simulink model "ScaraRobotApresentacao2023"  (R2024a)
(part 7 of 10)

out1 = ft_5({Ixx4,Ixx5,Ixx6,Ixy4,Ixy5,Ixy6,Ixz4,Ixz5,Ixz6,Iyx4,Iyx5,Iyx6,Iyy4,Iyy5,Iyy6,Iyz4,Iyz5,Iyz6,Izx4,Izx5,Izx6,Izy4,Izy5,Izy6,Izz4,Izz5,Izz6,Lx2,Lx3,Lxcm3,Lxcm4,Lxcm5,Lxcm6,Lycm4,Lycm5,Lycm6,Lz4,Lz5,Lzcm3,Lzcm4,Lzcm5,Lzcm6,dQ1,dQ2,dQ3,dQ4,dQ5,dQ6,et1,et10,et100,et101,et102,et103,et104,et105,et106,et107,et108,et109,et11,et110,et111,et112,et113,et114,et115,et116,et117,et118,et119,et12,et120,et121,et122,et123,et124,et125,et126,et127,et128,et129,et13,et130,et131,et132,et133,et134,et135,et136,et137,et138,et139,et14,et140,et141,et142,et143,et144,et145,et146,et147,et148,et149,et15,et150,et151,et152,et153,et154,et155,et156,et157,et158,et159,et16,et160,et161,et162,et163,et164,et165,et166,et167,et168,et169,et17,et170,et171,et172,et173,et174,et175,et176,et177,et178,et179,et18,et180,et181,et182,et183,et184,et185,et19,et2,et20,et21,et22,et23,et24,et25,et26,et27,et28,et29,et3,et30,et31,et32,et33,et34,et35,et36,et37,et38,et39,et4,et40,et41,et42,et43,et44,et45,et46,et47,et48,et49,et5,et50,et51,et52,et53,et54,et55,et56,et57,et58,et59,et6,et60,et61,et62,et63,et64,et65,et66,et67,et68,et69,et7,et70,et71,et72,et73,et74,et75,et76,et77,et78,et79,et8,et80,et81,et82,et83,et84,et85,et86,et87,et88,et89,et9,et90,et91,et92,et93,et94,et95,et96,et97,et98,et99,m3,m4,m5,m6,t10,t100,t1001,t1002,t1003,t1004,t1005,t1006,t1007,t1008,t1009,t1010,t1011,t1012,t1013,t1014,t1015,t1016,t1017,t1018,t1019,t102,t1020,t1021,t1022,t1023,t1024,t1025,t1026,t1027,t1028,t1029,t1030,t1033,t1034,t1035,t1036,t1037,t1038,t1039,t1041,t1046,t106,t1060,t1061,t1062,t1063,t1064,t1065,t1066,t1067,t107,t1072,t1073,t1074,t1075,t1076,t1077,t1078,t1079,t1082,t1083,t1084,t1085,t1093,t1094,t1095,t1096,t1097,t1098,t1099,t11,t1103,t1104,t1105,t1106,t1107,t1108,t1109,t1110,t1111,t1112,t1113,t1114,t1115,t1116,t1117,t1118,t1120,t1127,t1139,t1140,t1145,t1146,t1147,t1148,t1149,t1150,t1154,t1155,t1158,t1159,t1167,t1169,t1170,t1173,t1174,t1175,t1177,t1178,t1179,t118,t1180,t1181,t1182,t1187,t119,t1193,t1194,t1197,t1198,t1199,t120,t1200,t1202,t1204,t1205,t1206,t1208,t121,t1213,t1214,t1215,t1216,t1217,t1218,t1219,t122,t1223,t1224,t1225,t1226,t1227,t1228,t1229,t123,t1230,t1231,t1236,t1237,t124,t1242,t1243,t1246,t1249,t125,t1250,t1251,t1252,t1253,t1254,t1255,t1256,t1257,t1258,t1259,t126,t1262,t1263,t1264,t1265,t1266,t1269,t127,t1272,t1275,t1276,t1278,t1279,t128,t1283,t1285,t1286,t1287,t1288,t1289,t129,t1290,t1291,t1292,t1293,t1294,t1295,t1296,t1297,t1298,t1299,t130,t1300,t1301,t1302,t1303,t1304,t1305,t1306,t1307,t1308,t1309,t131,t1310,t1311,t1312,t1313,t1314,t1315,t1316,t1317,t1318,t1319,t132,t1320,t1321,t1322,t1323,t1324,t1325,t1326,t1327,t1328,t1329,t1330,t1331,t1332,t1333,t1334,t1335,t1336,t1337,t1338,t1339,t1340,t1341,t1342,t1343,t1344,t1345,t1346,t1347,t1348,t1349,t1350,t1351,t1352,t1353,t1354,t1355,t1356,t1357,t1358,t1359,t136,t1360,t1361,t1362,t1363,t1364,t1365,t1366,t1367,t1368,t1369,t137,t1370,t1371,t1372,t1373,t1374,t1375,t1376,t1377,t1378,t1379,t138,t1381,t1382,t1383,t1384,t1385,t1386,t1387,t1388,t1389,t139,t1390,t1391,t1392,t1393,t1394,t1395,t1396,t1397,t1398,t1399,t1400,t1401,t1402,t1403,t1404,t1405,t1406,t1407,t1408,t1409,t141,t1410,t1411,t142,t1420,t1421,t1422,t1423,t1424,t1425,t1426,t1427,t1428,t1429,t143,t1430,t1431,t1432,t1433,t1434,t1435,t1436,t1437,t1438,t1439,t144,t1440,t1441,t1442,t1443,t1444,t1445,t1446,t1447,t1448,t1449,t145,t1450,t1451,t1452,t1453,t1454,t1455,t1456,t1457,t1458,t146,t1461,t1462,t1469,t147,t1471,t1472,t1474,t1475,t148,t1481,t1482,t1484,t1487,t149,t1490,t1493,t1496,t1497,t1498,t1499,t15,t150,t1500,t1501,t1502,t1503,t1504,t1505,t1506,t1507,t1508,t1509,t151,t1510,t1511,t1512,t1513,t1514,t1515,t1516,t1517,t1518,t1519,t152,t1520,t1521,t1522,t1523,t1524,t1525,t1526,t153,t1531,t1532,t1533,t1534,t1535,t1536,t1539,t154,t1540,t1547,t1548,t1549,t155,t1550,t1555,t156,t1560,t1561,t1562,t1565,t1566,t157,t1575,t1576,t1577,t1578,t1579,t1580,t1581,t1582,t1583,t1589,t1590,t1591,t1592,t1593,t1594,t1595,t1596,t1597,t16,t1600,t1601,t1602,t1603,t1604,t1605,t1610,t1613,t1617,t1618,t1619,t1627,t1628,t1629,t1630,t1631,t1632,t1633,t1634,t1637,t1639,t1640,t1641,t1642,t1643,t1644,t1645,t1646,t1647,t1648,t1649,t1650,t1651,t1652,t1653,t1654,t1655,t1656,t1657,t1658,t1659,t1660,t1661,t1662,t1663,t1664,t1665,t1672,t1673,t1674,t1675,t1676,t1677,t1678,t1679,t1680,t1683,t1684,t1687,t1688,t1691,t1694,t1695,t1696,t1697,t1698,t1699,t17,t170,t1700,t171,t172,t1721,t1722,t1725,t1726,t173,t1730,t1731,t1733,t1734,t1735,t1736,t174,t1740,t1744,t1745,t1754,t1755,t1756,t1759,t1760,t1761,t1762,t1763,t1764,t1765,t1766,t1767,t1768,t1769,t177,t1770,t1771,t1772,t1773,t1774,t1775,t1777,t1778,t1779,t178,t1780,t1781,t1782,t1783,t1784,t1785,t1786,t1787,t1788,t1789,t179,t1790,t1791,t1792,t1793,t1794,t1795,t1796,t1797,t1798,t1799,t18,t180,t1800,t1801,t1802,t1803,t1804,t1808,t1809,t1814,t1815,t1816,t1817,t1818,t1819,t1820,t1821,t1822,t1823,t1827,t1828,t1829,t1830,t1831,t1832,t1833,t1834,t1835,t1840,t1841,t1847,t185,t1850,t1851,t1852,t1853,t1854,t1855,t1856,t1857,t1858,t1859,t186,t1860,t1861,t1862,t1863,t1864,t1865,t1866,t1867,t1868,t1869,t1870,t1871,t1872,t1873,t1874,t1875,t1876,t1877,t1878,t1879,t1880,t1884,t1885,t1886,t1887,t1888,t1889,t1890,t1891,t1892,t1893,t1894,t1895,t1896,t1897,t1898,t1899,t19,t1900,t1901,t1902,t1903,t1904,t1905,t1906,t1907,t1908,t1909,t1910,t1911,t1912,t1913,t1914,t1915,t1916,t1917,t1918,t1919,t1920,t1921,t1922,t1924,t1925,t1926,t1927,t1934,t1935,t1936,t1937,t1938,t1939,t1940,t1944,t1945,t1946,t1947,t1948,t1949,t1950,t1951,t1952,t1959,t1960,t1961,t1962,t1969,t1970,t1971,t1972,t1973,t1974,t1975,t1981,t1982,t1983,t1984,t1985,t1986,t1987,t1988,t1989,t1990,t1991,t1992,t1993,t1994,t1995,t1996,t1997,t1998,t1999,t2,t20,t2000,t2001,t2002,t2003,t201,t202,t2023,t2024,t2025,t2026,t2027,t203,t2034,t2035,t2036,t2037,t2038,t2039,t204,t2040,t2041,t2042,t2043,t2044,t2045,t2047,t2048,t2049,t205,t2050,t2051,t206,t2061,t2062,t2063,t2064,t2065,t2066,t2067,t2068,t207,t2076,t2077,t2078,t208,t2082,t2083,t2084,t209,t2091,t2092,t2093,t2094,t2096,t2097,t2098,t2099,t210,t2100,t2101,t2102,t2103,t2104,t2105,t2106,t2107,t2108,t2109,t211,t2110,t2111,t2112,t2113,t2114,t2115,t2116,t2117,t2118,t2119,t212,t2120,t2121,t2122,t2123,t2125,t2126,t2127,t2128,t2129,t213,t2130,t2131,t2132,t2133,t2134,t2135,t2136,t2137,t2138,t2139,t214,t2140,t2141,t2142,t2143,t2144,t2145,t2147,t2148,t2149,t215,t2150,t2151,t2152,t2153,t2154,t2155,t2156,t2157,t2158,t2159,t216,t2160,t2161,t2162,t2163,t2164,t2165,t2166,t2167,t2168,t2169,t217,t2170,t2171,t2172,t2173,t2174,t2175,t218,t2183,t2184,t2185,t2186,t2187,t2188,t2189,t219,t2190,t2191,t2192,t2193,t2194,t2195,t2196,t2198,t2199,t22,t220,t2200,t2201,t2202,t2203,t2204,t2205,t2206,t2207,t2214,t2215,t2218,t2219,t222,t2220,t2221,t2222,t2223,t2230,t2231,t2232,t2235,t2236,t2237,t2243,t2244,t2245,t2246,t2247,t2248,t225,t2263,t2264,t2265,t2266,t2267,t2268,t2269,t227,t2270,t2271,t2272,t2273,t2274,t2275,t2276,t2277,t2278,t2279,t228,t2280,t2281,t2282,t2283,t2284,t2287,t2288,t2289,t229,t2290,t2291,t2292,t2293,t2294,t2295,t2296,t2297,t2298,t230,t231,t2314,t2315,t2316,t2317,t2318,t2319,t232,t2320,t2321,t2322,t2323,t2324,t2325,t2326,t2327,t233,t2331,t2332,t2333,t2334,t2336,t2337,t2338,t2339,t234,t2340,t2341,t2342,t2343,t2344,t2345,t2346,t2347,t2348,t235,t2353,t2354,t2355,t236,t2360,t2362,t2363,t2364,t2365,t2366,t2367,t2368,t2369,t237,t2370,t2371,t2372,t2373,t2374,t2375,t2376,t2377,t2378,t2383,t2384,t2385,t2386,t2387,t2388,t2389,t239,t2390,t2391,t2392,t2393,t2394,t2395,t2396,t2397,t2398,t2399,t240,t2404,t2405,t2406,t2407,t2408,t2409,t2412,t2413,t2414,t2415,t2416,t2417,t242,t243,t244,t245,t25,t250,t251,t252,t253,t258,t259,t26,t260,t263,t264,t265,t266,t269,t270,t273,t274,t276,t277,t278,t279,t282,t283,t286,t287,t289,t290,t292,t293,t297,t298,t299,t3,t300,t301,t302,t303,t304,t305,t306,t307,t308,t309,t310,t311,t312,t313,t314,t315,t316,t317,t318,t319,t32,t320,t321,t322,t323,t324,t325,t326,t327,t328,t33,t331,t332,t333,t334,t34,t340,t341,t342,t343,t349,t35,t351,t358,t36,t363,t364,t367,t368,t369,t370,t377,t378,t379,t380,t381,t382,t383,t384,t385,t386,t39,t4,t40,t402,t403,t404,t405,t406,t407,t41,t413,t414,t415,t416,t417,t418,t419,t42,t43,t430,t431,t432,t433,t434,t435,t436,t437,t438,t44,t442,t443,t444,t445,t446,t447,t45,t454,t455,t456,t457,t458,t459,t46,t460,t461,t462,t463,t464,t465,t466,t467,t468,t469,t47,t470,t471,t472,t473,t474,t475,t476,t477,t478,t479,t48,t480,t481,t482,t483,t484,t485,t486,t487,t488,t489,t49,t490,t491,t492,t493,t494,t495,t496,t497,t498,t5,t50,t500,t506,t51,t512,t514,t515,t516,t52,t527,t528,t529,t53,t54,t540,t542,t543,t544,t546,t547,t548,t55,t550,t552,t554,t555,t556,t557,t558,t559,t56,t560,t561,t562,t563,t564,t565,t566,t567,t568,t569,t57,t570,t571,t572,t573,t574,t575,t576,t577,t578,t579,t58,t580,t581,t582,t583,t584,t585,t586,t587,t588,t589,t59,t590,t591,t592,t593,t594,t595,t596,t597,t598,t599,t6,t60,t600,t601,t602,t603,t604,t605,t606,t607,t608,t609,t61,t610,t611,t612,t613,t614,t615,t616,t617,t618,t619,t62,t620,t621,t622,t623,t624,t625,t626,t627,t628,t629,t63,t630,t631,t632,t635,t636,t637,t638,t64,t648,t650,t651,t658,t659,t660,t661,t662,t663,t664,t669,t67,t670,t671,t674,t675,t676,t677,t68,t681,t684,t687,t688,t689,t69,t690,t694,t697,t698,t699,t7,t70,t700,t701,t702,t703,t704,t705,t706,t707,t708,t709,t71,t710,t711,t716,t717,t718,t719,t72,t720,t721,t724,t725,t728,t729,t73,t730,t731,t732,t733,t734,t735,t737,t738,t739,t74,t746,t748,t749,t75,t750,t752,t754,t755,t756,t759,t760,t761,t762,t774,t775,t776,t777,t778,t779,t78,t780,t781,t782,t783,t785,t788,t79,t791,t792,t793,t794,t795,t796,t797,t798,t8,t80,t800,t801,t803,t804,t806,t807,t809,t81,t810,t82,t828,t829,t83,t830,t831,t832,t833,t834,t835,t836,t837,t838,t839,t84,t840,t843,t844,t845,t848,t849,t85,t851,t852,t857,t858,t86,t861,t862,t868,t869,t87,t870,t871,t872,t873,t874,t875,t876,t877,t878,t879,t88,t880,t881,t882,t883,t884,t885,t886,t887,t888,t889,t89,t890,t891,t892,t893,t894,t895,t896,t897,t898,t899,t9,t90,t900,t901,t902,t903,t904,t905,t906,t907,t908,t909,t91,t910,t911,t912,t913,t914,t915,t916,t917,t918,t919,t92,t920,t921,t922,t923,t924,t925,t926,t927,t928,t929,t93,t930,t931,t932,t933,t934,t935,t936,t938,t939,t94,t940,t941,t942,t943,t948,t949,t950,t951,t952,t953,t954,t955,t956,t957,t958,t959,t96,t960,t961,t962,t963,t964,t965,t966,t967,t968,t969,t972,t973,t978,t979,t984,t985,t988,t989,t990,t991,t992,t993,t994,t995,t996,t997,t998});
end
function out1 = ft_5(ct)
[Ixx4,Ixx5,Ixx6,Ixy4,Ixy5,Ixy6,Ixz4,Ixz5,Ixz6,Iyx4,Iyx5,Iyx6,Iyy4,Iyy5,Iyy6,Iyz4,Iyz5,Iyz6,Izx4,Izx5,Izx6,Izy4,Izy5,Izy6,Izz4,Izz5,Izz6,Lx2,Lx3,Lxcm3,Lxcm4,Lxcm5,Lxcm6,Lycm4,Lycm5,Lycm6,Lz4,Lz5,Lzcm3,Lzcm4,Lzcm5,Lzcm6,dQ1,dQ2,dQ3,dQ4,dQ5,dQ6,et1,et10,et100,et101,et102,et103,et104,et105,et106,et107,et108,et109,et11,et110,et111,et112,et113,et114,et115,et116,et117,et118,et119,et12,et120,et121,et122,et123,et124,et125,et126,et127,et128,et129,et13,et130,et131,et132,et133,et134,et135,et136,et137,et138,et139,et14,et140,et141,et142,et143,et144,et145,et146,et147,et148,et149,et15,et150,et151,et152,et153,et154,et155,et156,et157,et158,et159,et16,et160,et161,et162,et163,et164,et165,et166,et167,et168,et169,et17,et170,et171,et172,et173,et174,et175,et176,et177,et178,et179,et18,et180,et181,et182,et183,et184,et185,et19,et2,et20,et21,et22,et23,et24,et25,et26,et27,et28,et29,et3,et30,et31,et32,et33,et34,et35,et36,et37,et38,et39,et4,et40,et41,et42,et43,et44,et45,et46,et47,et48,et49,et5,et50,et51,et52,et53,et54,et55,et56,et57,et58,et59,et6,et60,et61,et62,et63,et64,et65,et66,et67,et68,et69,et7,et70,et71,et72,et73,et74,et75,et76,et77,et78,et79,et8,et80,et81,et82,et83,et84,et85,et86,et87,et88,et89,et9,et90,et91,et92,et93,et94,et95,et96,et97,et98,et99,m3,m4,m5,m6,t10,t100,t1001,t1002,t1003,t1004,t1005,t1006,t1007,t1008,t1009,t1010,t1011,t1012,t1013,t1014,t1015,t1016,t1017,t1018,t1019,t102,t1020,t1021,t1022,t1023,t1024,t1025,t1026,t1027,t1028,t1029,t1030,t1033,t1034,t1035,t1036,t1037,t1038,t1039,t1041,t1046,t106,t1060,t1061,t1062,t1063,t1064,t1065,t1066,t1067,t107,t1072,t1073,t1074,t1075,t1076,t1077,t1078,t1079,t1082,t1083,t1084,t1085,t1093,t1094,t1095,t1096,t1097,t1098,t1099,t11,t1103,t1104,t1105,t1106,t1107,t1108,t1109,t1110,t1111,t1112,t1113,t1114,t1115,t1116,t1117,t1118,t1120,t1127,t1139,t1140,t1145,t1146,t1147,t1148,t1149,t1150,t1154,t1155,t1158,t1159,t1167,t1169,t1170,t1173,t1174,t1175,t1177,t1178,t1179,t118,t1180,t1181,t1182,t1187,t119,t1193,t1194,t1197,t1198,t1199,t120,t1200,t1202,t1204,t1205,t1206,t1208,t121,t1213,t1214,t1215,t1216,t1217,t1218,t1219,t122,t1223,t1224,t1225,t1226,t1227,t1228,t1229,t123,t1230,t1231,t1236,t1237,t124,t1242,t1243,t1246,t1249,t125,t1250,t1251,t1252,t1253,t1254,t1255,t1256,t1257,t1258,t1259,t126,t1262,t1263,t1264,t1265,t1266,t1269,t127,t1272,t1275,t1276,t1278,t1279,t128,t1283,t1285,t1286,t1287,t1288,t1289,t129,t1290,t1291,t1292,t1293,t1294,t1295,t1296,t1297,t1298,t1299,t130,t1300,t1301,t1302,t1303,t1304,t1305,t1306,t1307,t1308,t1309,t131,t1310,t1311,t1312,t1313,t1314,t1315,t1316,t1317,t1318,t1319,t132,t1320,t1321,t1322,t1323,t1324,t1325,t1326,t1327,t1328,t1329,t1330,t1331,t1332,t1333,t1334,t1335,t1336,t1337,t1338,t1339,t1340,t1341,t1342,t1343,t1344,t1345,t1346,t1347,t1348,t1349,t1350,t1351,t1352,t1353,t1354,t1355,t1356,t1357,t1358,t1359,t136,t1360,t1361,t1362,t1363,t1364,t1365,t1366,t1367,t1368,t1369,t137,t1370,t1371,t1372,t1373,t1374,t1375,t1376,t1377,t1378,t1379,t138,t1381,t1382,t1383,t1384,t1385,t1386,t1387,t1388,t1389,t139,t1390,t1391,t1392,t1393,t1394,t1395,t1396,t1397,t1398,t1399,t1400,t1401,t1402,t1403,t1404,t1405,t1406,t1407,t1408,t1409,t141,t1410,t1411,t142,t1420,t1421,t1422,t1423,t1424,t1425,t1426,t1427,t1428,t1429,t143,t1430,t1431,t1432,t1433,t1434,t1435,t1436,t1437,t1438,t1439,t144,t1440,t1441,t1442,t1443,t1444,t1445,t1446,t1447,t1448,t1449,t145,t1450,t1451,t1452,t1453,t1454,t1455,t1456,t1457,t1458,t146,t1461,t1462,t1469,t147,t1471,t1472,t1474,t1475,t148,t1481,t1482,t1484,t1487,t149,t1490,t1493,t1496,t1497,t1498,t1499,t15,t150,t1500,t1501,t1502,t1503,t1504,t1505,t1506,t1507,t1508,t1509,t151,t1510,t1511,t1512,t1513,t1514,t1515,t1516,t1517,t1518,t1519,t152,t1520,t1521,t1522,t1523,t1524,t1525,t1526,t153,t1531,t1532,t1533,t1534,t1535,t1536,t1539,t154,t1540,t1547,t1548,t1549,t155,t1550,t1555,t156,t1560,t1561,t1562,t1565,t1566,t157,t1575,t1576,t1577,t1578,t1579,t1580,t1581,t1582,t1583,t1589,t1590,t1591,t1592,t1593,t1594,t1595,t1596,t1597,t16,t1600,t1601,t1602,t1603,t1604,t1605,t1610,t1613,t1617,t1618,t1619,t1627,t1628,t1629,t1630,t1631,t1632,t1633,t1634,t1637,t1639,t1640,t1641,t1642,t1643,t1644,t1645,t1646,t1647,t1648,t1649,t1650,t1651,t1652,t1653,t1654,t1655,t1656,t1657,t1658,t1659,t1660,t1661,t1662,t1663,t1664,t1665,t1672,t1673,t1674,t1675,t1676,t1677,t1678,t1679,t1680,t1683,t1684,t1687,t1688,t1691,t1694,t1695,t1696,t1697,t1698,t1699,t17,t170,t1700,t171,t172,t1721,t1722,t1725,t1726,t173,t1730,t1731,t1733,t1734,t1735,t1736,t174,t1740,t1744,t1745,t1754,t1755,t1756,t1759,t1760,t1761,t1762,t1763,t1764,t1765,t1766,t1767,t1768,t1769,t177,t1770,t1771,t1772,t1773,t1774,t1775,t1777,t1778,t1779,t178,t1780,t1781,t1782,t1783,t1784,t1785,t1786,t1787,t1788,t1789,t179,t1790,t1791,t1792,t1793,t1794,t1795,t1796,t1797,t1798,t1799,t18,t180,t1800,t1801,t1802,t1803,t1804,t1808,t1809,t1814,t1815,t1816,t1817,t1818,t1819,t1820,t1821,t1822,t1823,t1827,t1828,t1829,t1830,t1831,t1832,t1833,t1834,t1835,t1840,t1841,t1847,t185,t1850,t1851,t1852,t1853,t1854,t1855,t1856,t1857,t1858,t1859,t186,t1860,t1861,t1862,t1863,t1864,t1865,t1866,t1867,t1868,t1869,t1870,t1871,t1872,t1873,t1874,t1875,t1876,t1877,t1878,t1879,t1880,t1884,t1885,t1886,t1887,t1888,t1889,t1890,t1891,t1892,t1893,t1894,t1895,t1896,t1897,t1898,t1899,t19,t1900,t1901,t1902,t1903,t1904,t1905,t1906,t1907,t1908,t1909,t1910,t1911,t1912,t1913,t1914,t1915,t1916,t1917,t1918,t1919,t1920,t1921,t1922,t1924,t1925,t1926,t1927,t1934,t1935,t1936,t1937,t1938,t1939,t1940,t1944,t1945,t1946,t1947,t1948,t1949,t1950,t1951,t1952,t1959,t1960,t1961,t1962,t1969,t1970,t1971,t1972,t1973,t1974,t1975,t1981,t1982,t1983,t1984,t1985,t1986,t1987,t1988,t1989,t1990,t1991,t1992,t1993,t1994,t1995,t1996,t1997,t1998,t1999,t2,t20,t2000,t2001,t2002,t2003,t201,t202,t2023,t2024,t2025,t2026,t2027,t203,t2034,t2035,t2036,t2037,t2038,t2039,t204,t2040,t2041,t2042,t2043,t2044,t2045,t2047,t2048,t2049,t205,t2050,t2051,t206,t2061,t2062,t2063,t2064,t2065,t2066,t2067,t2068,t207,t2076,t2077,t2078,t208,t2082,t2083,t2084,t209,t2091,t2092,t2093,t2094,t2096,t2097,t2098,t2099,t210,t2100,t2101,t2102,t2103,t2104,t2105,t2106,t2107,t2108,t2109,t211,t2110,t2111,t2112,t2113,t2114,t2115,t2116,t2117,t2118,t2119,t212,t2120,t2121,t2122,t2123,t2125,t2126,t2127,t2128,t2129,t213,t2130,t2131,t2132,t2133,t2134,t2135,t2136,t2137,t2138,t2139,t214,t2140,t2141,t2142,t2143,t2144,t2145,t2147,t2148,t2149,t215,t2150,t2151,t2152,t2153,t2154,t2155,t2156,t2157,t2158,t2159,t216,t2160,t2161,t2162,t2163,t2164,t2165,t2166,t2167,t2168,t2169,t217,t2170,t2171,t2172,t2173,t2174,t2175,t218,t2183,t2184,t2185,t2186,t2187,t2188,t2189,t219,t2190,t2191,t2192,t2193,t2194,t2195,t2196,t2198,t2199,t22,t220,t2200,t2201,t2202,t2203,t2204,t2205,t2206,t2207,t2214,t2215,t2218,t2219,t222,t2220,t2221,t2222,t2223,t2230,t2231,t2232,t2235,t2236,t2237,t2243,t2244,t2245,t2246,t2247,t2248,t225,t2263,t2264,t2265,t2266,t2267,t2268,t2269,t227,t2270,t2271,t2272,t2273,t2274,t2275,t2276,t2277,t2278,t2279,t228,t2280,t2281,t2282,t2283,t2284,t2287,t2288,t2289,t229,t2290,t2291,t2292,t2293,t2294,t2295,t2296,t2297,t2298,t230,t231,t2314,t2315,t2316,t2317,t2318,t2319,t232,t2320,t2321,t2322,t2323,t2324,t2325,t2326,t2327,t233,t2331,t2332,t2333,t2334,t2336,t2337,t2338,t2339,t234,t2340,t2341,t2342,t2343,t2344,t2345,t2346,t2347,t2348,t235,t2353,t2354,t2355,t236,t2360,t2362,t2363,t2364,t2365,t2366,t2367,t2368,t2369,t237,t2370,t2371,t2372,t2373,t2374,t2375,t2376,t2377,t2378,t2383,t2384,t2385,t2386,t2387,t2388,t2389,t239,t2390,t2391,t2392,t2393,t2394,t2395,t2396,t2397,t2398,t2399,t240,t2404,t2405,t2406,t2407,t2408,t2409,t2412,t2413,t2414,t2415,t2416,t2417,t242,t243,t244,t245,t25,t250,t251,t252,t253,t258,t259,t26,t260,t263,t264,t265,t266,t269,t270,t273,t274,t276,t277,t278,t279,t282,t283,t286,t287,t289,t290,t292,t293,t297,t298,t299,t3,t300,t301,t302,t303,t304,t305,t306,t307,t308,t309,t310,t311,t312,t313,t314,t315,t316,t317,t318,t319,t32,t320,t321,t322,t323,t324,t325,t326,t327,t328,t33,t331,t332,t333,t334,t34,t340,t341,t342,t343,t349,t35,t351,t358,t36,t363,t364,t367,t368,t369,t370,t377,t378,t379,t380,t381,t382,t383,t384,t385,t386,t39,t4,t40,t402,t403,t404,t405,t406,t407,t41,t413,t414,t415,t416,t417,t418,t419,t42,t43,t430,t431,t432,t433,t434,t435,t436,t437,t438,t44,t442,t443,t444,t445,t446,t447,t45,t454,t455,t456,t457,t458,t459,t46,t460,t461,t462,t463,t464,t465,t466,t467,t468,t469,t47,t470,t471,t472,t473,t474,t475,t476,t477,t478,t479,t48,t480,t481,t482,t483,t484,t485,t486,t487,t488,t489,t49,t490,t491,t492,t493,t494,t495,t496,t497,t498,t5,t50,t500,t506,t51,t512,t514,t515,t516,t52,t527,t528,t529,t53,t54,t540,t542,t543,t544,t546,t547,t548,t55,t550,t552,t554,t555,t556,t557,t558,t559,t56,t560,t561,t562,t563,t564,t565,t566,t567,t568,t569,t57,t570,t571,t572,t573,t574,t575,t576,t577,t578,t579,t58,t580,t581,t582,t583,t584,t585,t586,t587,t588,t589,t59,t590,t591,t592,t593,t594,t595,t596,t597,t598,t599,t6,t60,t600,t601,t602,t603,t604,t605,t606,t607,t608,t609,t61,t610,t611,t612,t613,t614,t615,t616,t617,t618,t619,t62,t620,t621,t622,t623,t624,t625,t626,t627,t628,t629,t63,t630,t631,t632,t635,t636,t637,t638,t64,t648,t650,t651,t658,t659,t660,t661,t662,t663,t664,t669,t67,t670,t671,t674,t675,t676,t677,t68,t681,t684,t687,t688,t689,t69,t690,t694,t697,t698,t699,t7,t70,t700,t701,t702,t703,t704,t705,t706,t707,t708,t709,t71,t710,t711,t716,t717,t718,t719,t72,t720,t721,t724,t725,t728,t729,t73,t730,t731,t732,t733,t734,t735,t737,t738,t739,t74,t746,t748,t749,t75,t750,t752,t754,t755,t756,t759,t760,t761,t762,t774,t775,t776,t777,t778,t779,t78,t780,t781,t782,t783,t785,t788,t79,t791,t792,t793,t794,t795,t796,t797,t798,t8,t80,t800,t801,t803,t804,t806,t807,t809,t81,t810,t82,t828,t829,t83,t830,t831,t832,t833,t834,t835,t836,t837,t838,t839,t84,t840,t843,t844,t845,t848,t849,t85,t851,t852,t857,t858,t86,t861,t862,t868,t869,t87,t870,t871,t872,t873,t874,t875,t876,t877,t878,t879,t88,t880,t881,t882,t883,t884,t885,t886,t887,t888,t889,t89,t890,t891,t892,t893,t894,t895,t896,t897,t898,t899,t9,t90,t900,t901,t902,t903,t904,t905,t906,t907,t908,t909,t91,t910,t911,t912,t913,t914,t915,t916,t917,t918,t919,t92,t920,t921,t922,t923,t924,t925,t926,t927,t928,t929,t93,t930,t931,t932,t933,t934,t935,t936,t938,t939,t94,t940,t941,t942,t943,t948,t949,t950,t951,t952,t953,t954,t955,t956,t957,t958,t959,t96,t960,t961,t962,t963,t964,t965,t966,t967,t968,t969,t972,t973,t978,t979,t984,t985,t988,t989,t990,t991,t992,t993,t994,t995,t996,t997,t998] = ct{:};
et186 = Ixz6.*dQ1.*dQ4.*t4.*t5.*t6.*t9.*t10.*t33.*2.0+Ixz6.*dQ3.*dQ4.*t2.*t5.*t6.*t8.*t10.*t34.*2.0+Ixz6.*dQ3.*dQ4.*t3.*t5.*t6.*t7.*t10.*t34.*2.0+Ixz6.*dQ1.*dQ5.*t2.*t7.*t9.*t10.*t11.*t33.*2.0+Ixz6.*dQ1.*dQ5.*t3.*t8.*t9.*t10.*t11.*t32.*2.0-Ixz5.*dQ1.*dQ2.*t2.*t5.*t7.*t10.*t33.*t34.*4.0-Ixz5.*dQ1.*dQ2.*t3.*t5.*t8.*t10.*t32.*t34.*4.0-Ixz5.*dQ1.*dQ3.*t2.*t5.*t7.*t10.*t33.*t34.*4.0-Ixz5.*dQ1.*dQ5.*t2.*t3.*t7.*t8.*t34.*t35.*4.0-Ixz5.*dQ1.*dQ3.*t3.*t5.*t8.*t10.*t32.*t34.*4.0-Ixz5.*dQ1.*dQ4.*t4.*t5.*t9.*t10.*t32.*t33.*4.0-Ixz6.*dQ1.*dQ4.*t2.*t6.*t7.*t9.*t33.*t35.*4.0-Ixz6.*dQ1.*dQ4.*t3.*t6.*t8.*t9.*t32.*t35.*4.0-Ixz6.*dQ1.*dQ6.*t2.*t4.*t7.*t11.*t33.*t35.*4.0-Ixz6.*dQ1.*dQ5.*t4.*t5.*t9.*t11.*t32.*t33.*2.0-Ixz6.*dQ1.*dQ6.*t3.*t4.*t8.*t11.*t32.*t35.*4.0-Ixz6.*dQ1.*dQ6.*t4.*t6.*t9.*t10.*t32.*t33.*2.0;
et187 = Ixz6.*dQ1.*dQ6.*t5.*t10.*t11.*t32.*t33.*t34.*-2.0-Iyx6.*dQ2.*dQ3.*t2.*t3.*t4.*t6.*t9.*t11.*2.0-Iyx5.*dQ1.*dQ2.*t2.*t3.*t7.*t8.*t9.*t10.*4.0-Iyx5.*dQ1.*dQ3.*t2.*t3.*t7.*t8.*t9.*t10.*4.0+Iyx6.*dQ1.*dQ2.*t2.*t3.*t7.*t8.*t9.*t10.*4.0+Iyx6.*dQ1.*dQ3.*t2.*t3.*t7.*t8.*t9.*t10.*4.0-Iyx6.*dQ2.*dQ6.*t2.*t3.*t4.*t6.*t10.*t11.*2.0-Iyx6.*dQ3.*dQ6.*t2.*t3.*t4.*t6.*t10.*t11.*2.0+Iyx6.*dQ4.*dQ5.*t2.*t3.*t5.*t6.*t10.*t11.*2.0+Iyx6.*dQ2.*dQ3.*t4.*t6.*t7.*t8.*t9.*t11.*2.0+Iyx6.*dQ1.*dQ6.*t2.*t6.*t7.*t9.*t10.*t11.*4.0+Iyx6.*dQ1.*dQ6.*t3.*t6.*t8.*t9.*t10.*t11.*4.0+Iyx6.*dQ2.*dQ6.*t4.*t6.*t7.*t8.*t10.*t11.*2.0+Iyx6.*dQ3.*dQ6.*t4.*t6.*t7.*t8.*t10.*t11.*2.0-Iyx6.*dQ4.*dQ5.*t5.*t6.*t7.*t8.*t10.*t11.*2.0-Iyx6.*dQ4.*dQ6.*t2.*t6.*t8.*t9.*t10.*t11.*2.0-Iyx6.*dQ4.*dQ6.*t3.*t6.*t7.*t9.*t10.*t11.*2.0;
et188 = Iyx5.*dQ1.*dQ2.*t2.*t4.*t5.*t7.*t9.*t33.*4.0+Iyx5.*dQ1.*dQ2.*t3.*t4.*t5.*t8.*t9.*t32.*4.0+Iyx5.*dQ1.*dQ3.*t2.*t4.*t5.*t7.*t9.*t33.*4.0+Iyx5.*dQ1.*dQ4.*t2.*t3.*t5.*t7.*t8.*t34.*4.0-Iyx6.*dQ1.*dQ2.*t2.*t4.*t5.*t7.*t9.*t33.*4.0+Iyx5.*dQ1.*dQ3.*t3.*t4.*t5.*t8.*t9.*t32.*4.0-Iyx6.*dQ1.*dQ2.*t3.*t4.*t5.*t8.*t9.*t32.*4.0-Iyx6.*dQ1.*dQ3.*t2.*t4.*t5.*t7.*t9.*t33.*4.0-Iyx6.*dQ1.*dQ4.*t2.*t3.*t5.*t7.*t8.*t34.*4.0-Iyx6.*dQ1.*dQ3.*t3.*t4.*t5.*t8.*t9.*t32.*4.0-Iyx6.*dQ1.*dQ2.*t2.*t4.*t5.*t7.*t9.*t36.*4.0-Iyx6.*dQ1.*dQ4.*t2.*t3.*t5.*t7.*t8.*t36.*4.0-Iyx6.*dQ1.*dQ3.*t2.*t4.*t5.*t7.*t9.*t36.*4.0-Iyx6.*dQ1.*dQ2.*t3.*t4.*t5.*t8.*t9.*t36.*4.0-Iyx6.*dQ1.*dQ6.*t2.*t4.*t5.*t7.*t10.*t33.*4.0-Iyx6.*dQ1.*dQ3.*t3.*t4.*t5.*t8.*t9.*t36.*4.0-Iyx6.*dQ1.*dQ5.*t2.*t4.*t6.*t7.*t11.*t33.*4.0;
et189 = Iyx6.*dQ1.*dQ6.*t3.*t4.*t5.*t8.*t10.*t32.*-4.0-Iyx6.*dQ1.*dQ5.*t3.*t4.*t6.*t8.*t11.*t32.*4.0-Iyx6.*dQ1.*dQ2.*t4.*t5.*t6.*t10.*t11.*t32.*4.0-Iyx6.*dQ1.*dQ5.*t2.*t4.*t6.*t7.*t11.*t35.*4.0-Iyx6.*dQ1.*dQ6.*t2.*t4.*t5.*t7.*t10.*t36.*4.0-Iyx6.*dQ1.*dQ2.*t4.*t5.*t6.*t10.*t11.*t33.*4.0-Iyx6.*dQ1.*dQ3.*t4.*t5.*t6.*t10.*t11.*t32.*4.0-Iyx6.*dQ1.*dQ3.*t4.*t5.*t6.*t10.*t11.*t33.*4.0-Iyx6.*dQ1.*dQ5.*t3.*t4.*t6.*t8.*t11.*t35.*4.0-Iyx6.*dQ1.*dQ6.*t3.*t4.*t5.*t8.*t10.*t36.*4.0-Iyx6.*dQ2.*dQ5.*t2.*t3.*t6.*t9.*t11.*t35.*2.0-Iyx6.*dQ2.*dQ6.*t2.*t3.*t5.*t9.*t10.*t36.*2.0-Iyx6.*dQ1.*dQ6.*t4.*t5.*t6.*t9.*t11.*t32.*4.0-Iyx6.*dQ3.*dQ5.*t2.*t3.*t6.*t9.*t11.*t35.*2.0-Iyx6.*dQ3.*dQ6.*t2.*t3.*t5.*t9.*t10.*t36.*2.0-Iyx6.*dQ1.*dQ6.*t4.*t5.*t6.*t9.*t11.*t33.*4.0;
et190 = Iyx6.*dQ4.*dQ5.*t2.*t4.*t6.*t8.*t11.*t35.*2.0+Iyx6.*dQ4.*dQ5.*t3.*t4.*t6.*t7.*t11.*t35.*2.0+Iyx6.*dQ4.*dQ6.*t2.*t4.*t5.*t8.*t10.*t36.*2.0+Iyx6.*dQ4.*dQ6.*t3.*t4.*t5.*t7.*t10.*t36.*2.0+Iyx6.*dQ2.*dQ5.*t6.*t7.*t8.*t9.*t11.*t35.*2.0+Iyx6.*dQ2.*dQ6.*t5.*t7.*t8.*t9.*t10.*t36.*2.0+Iyx6.*dQ3.*dQ5.*t6.*t7.*t8.*t9.*t11.*t35.*2.0+Iyx6.*dQ3.*dQ6.*t5.*t7.*t8.*t9.*t10.*t36.*2.0+Iyx6.*dQ1.*dQ2.*t2.*t6.*t7.*t11.*t33.*t34.*4.0-Iyx6.*dQ1.*dQ6.*t2.*t3.*t7.*t8.*t34.*t35.*2.0+Iyx6.*dQ1.*dQ2.*t2.*t6.*t7.*t11.*t33.*t35.*4.0+Iyx6.*dQ1.*dQ2.*t3.*t6.*t8.*t11.*t32.*t34.*4.0+Iyx6.*dQ1.*dQ3.*t2.*t6.*t7.*t11.*t33.*t34.*4.0+Iyx6.*dQ1.*dQ4.*t2.*t4.*t7.*t10.*t33.*t36.*4.0+Iyx6.*dQ1.*dQ6.*t2.*t3.*t7.*t8.*t34.*t36.*4.0-Iyx6.*dQ1.*dQ2.*t2.*t6.*t7.*t11.*t34.*t35.*2.0+Iyx6.*dQ1.*dQ2.*t3.*t6.*t8.*t11.*t32.*t35.*4.0+Iyx6.*dQ1.*dQ3.*t2.*t6.*t7.*t11.*t33.*t35.*4.0;
et191 = Iyx6.*dQ1.*dQ3.*t3.*t6.*t8.*t11.*t32.*t34.*4.0+Iyx6.*dQ1.*dQ4.*t3.*t4.*t8.*t10.*t32.*t36.*4.0+Iyx6.*dQ1.*dQ5.*t2.*t5.*t7.*t9.*t33.*t36.*4.0+Iyx6.*dQ1.*dQ6.*t2.*t3.*t7.*t8.*t35.*t36.*4.0-Iyx6.*dQ1.*dQ3.*t2.*t6.*t7.*t11.*t34.*t35.*2.0+Iyx6.*dQ1.*dQ3.*t3.*t6.*t8.*t11.*t32.*t35.*4.0+Iyx6.*dQ1.*dQ5.*t3.*t5.*t8.*t9.*t32.*t36.*4.0-Iyx6.*dQ1.*dQ2.*t3.*t6.*t8.*t11.*t34.*t35.*2.0+Iyx6.*dQ1.*dQ4.*t4.*t6.*t9.*t11.*t32.*t33.*4.0-Iyx6.*dQ1.*dQ3.*t3.*t6.*t8.*t11.*t34.*t35.*2.0-Iyx6.*dQ1.*dQ4.*t4.*t6.*t9.*t11.*t32.*t35.*2.0-Iyx6.*dQ2.*dQ4.*t2.*t6.*t8.*t11.*t34.*t35.*2.0-Iyx6.*dQ2.*dQ4.*t3.*t6.*t7.*t11.*t34.*t35.*2.0-Iyx6.*dQ1.*dQ4.*t4.*t6.*t9.*t11.*t33.*t35.*2.0+Iyx6.*dQ1.*dQ5.*t5.*t6.*t10.*t11.*t32.*t33.*4.0-Iyx6.*dQ3.*dQ4.*t2.*t6.*t8.*t11.*t34.*t35.*2.0-Iyx6.*dQ3.*dQ4.*t3.*t6.*t7.*t11.*t34.*t35.*2.0;
et192 = Iyx6.*dQ1.*dQ5.*t5.*t6.*t10.*t11.*t32.*t34.*-2.0-Iyx6.*dQ1.*dQ5.*t5.*t6.*t10.*t11.*t33.*t34.*2.0+Iyx6.*dQ1.*dQ5.*t4.*t9.*t10.*t32.*t33.*t36.*4.0+Iyy6.*dQ2.*dQ5.*t2.*t3.*t4.*t5.*t6.*t11.*2.0+Iyy6.*dQ3.*dQ5.*t2.*t3.*t4.*t5.*t6.*t11.*2.0-Iyy6.*dQ1.*dQ5.*t2.*t3.*t5.*t7.*t8.*t10.*4.0-Iyy6.*dQ1.*dQ6.*t2.*t3.*t6.*t7.*t8.*t11.*8.0-Iyy6.*dQ1.*dQ4.*t2.*t4.*t6.*t7.*t10.*t11.*2.0+Iyy6.*dQ2.*dQ5.*t2.*t4.*t5.*t8.*t9.*t10.*2.0+Iyy6.*dQ2.*dQ5.*t3.*t4.*t5.*t7.*t9.*t10.*2.0-Iyy6.*dQ1.*dQ5.*t2.*t5.*t6.*t7.*t9.*t11.*2.0-Iyy6.*dQ2.*dQ3.*t2.*t4.*t6.*t8.*t10.*t11.*2.0-Iyy6.*dQ2.*dQ3.*t3.*t4.*t6.*t7.*t10.*t11.*2.0+Iyy6.*dQ3.*dQ5.*t2.*t4.*t5.*t8.*t9.*t10.*2.0+Iyy6.*dQ3.*dQ5.*t3.*t4.*t5.*t7.*t9.*t10.*2.0-Iyy6.*dQ1.*dQ4.*t3.*t4.*t6.*t8.*t10.*t11.*2.0-Iyy6.*dQ1.*dQ5.*t3.*t5.*t6.*t8.*t9.*t11.*2.0;
et193 = Iyy6.*dQ2.*dQ5.*t4.*t5.*t6.*t7.*t8.*t11.*-2.0-Iyy6.*dQ2.*dQ6.*t2.*t4.*t6.*t8.*t9.*t11.*2.0-Iyy6.*dQ2.*dQ6.*t3.*t4.*t6.*t7.*t9.*t11.*2.0-Iyy6.*dQ3.*dQ5.*t4.*t5.*t6.*t7.*t8.*t11.*2.0-Iyy6.*dQ3.*dQ6.*t2.*t4.*t6.*t8.*t9.*t11.*2.0-Iyy6.*dQ3.*dQ6.*t3.*t4.*t6.*t7.*t9.*t11.*2.0+Iyy6.*dQ2.*dQ3.*t2.*t3.*t5.*t6.*t11.*t34.*4.0-Iyy6.*dQ1.*dQ4.*t2.*t5.*t7.*t9.*t10.*t33.*4.0-Iyy6.*dQ1.*dQ4.*t3.*t5.*t8.*t9.*t10.*t32.*4.0-Iyy6.*dQ1.*dQ4.*t2.*t5.*t7.*t9.*t10.*t36.*2.0-Iyy6.*dQ2.*dQ3.*t2.*t5.*t8.*t9.*t10.*t36.*2.0-Iyy6.*dQ2.*dQ3.*t3.*t5.*t7.*t9.*t10.*t36.*2.0-Iyy6.*dQ1.*dQ4.*t3.*t5.*t8.*t9.*t10.*t36.*2.0-Iyy6.*dQ2.*dQ3.*t5.*t6.*t7.*t8.*t11.*t34.*4.0-Iyy6.*dQ1.*dQ5.*t4.*t6.*t9.*t10.*t11.*t32.*2.0-Iyy6.*dQ2.*dQ5.*t2.*t6.*t8.*t10.*t11.*t34.*2.0;
et194 = Iyy6.*dQ2.*dQ5.*t3.*t6.*t7.*t10.*t11.*t34.*-2.0-Iyy6.*dQ1.*dQ5.*t4.*t6.*t9.*t10.*t11.*t33.*2.0-Iyy6.*dQ3.*dQ5.*t2.*t6.*t8.*t10.*t11.*t34.*2.0-Iyy6.*dQ3.*dQ5.*t3.*t6.*t7.*t10.*t11.*t34.*2.0+Iyy6.*dQ2.*dQ3.*t2.*t3.*t4.*t9.*t35.*t36.*2.0+Iyy6.*dQ1.*dQ2.*t6.*t9.*t10.*t11.*t32.*t33.*8.0+Iyy6.*dQ1.*dQ6.*t2.*t7.*t9.*t10.*t33.*t36.*8.0-Iyy6.*dQ2.*dQ3.*t4.*t7.*t8.*t9.*t35.*t36.*2.0+Iyy6.*dQ1.*dQ3.*t6.*t9.*t10.*t11.*t32.*t33.*8.0+Iyy6.*dQ1.*dQ6.*t3.*t8.*t9.*t10.*t32.*t36.*8.0-Iyy6.*dQ1.*dQ2.*t4.*t5.*t10.*t32.*t33.*t36.*8.0-Iyy6.*dQ1.*dQ5.*t2.*t4.*t7.*t33.*t35.*t36.*8.0-Iyy6.*dQ1.*dQ3.*t4.*t5.*t10.*t32.*t33.*t36.*8.0-Iyy6.*dQ1.*dQ5.*t3.*t4.*t8.*t32.*t35.*t36.*8.0-Iyy6.*dQ1.*dQ4.*t5.*t6.*t11.*t32.*t33.*t34.*8.0-Iyy6.*dQ1.*dQ6.*t4.*t5.*t9.*t32.*t33.*t36.*8.0;
et195 = Iyy6.*dQ1.*dQ2.*t2.*t7.*t33.*t34.*t35.*t36.*-4.0-Iyy6.*dQ1.*dQ2.*t3.*t8.*t32.*t34.*t35.*t36.*4.0-Iyy6.*dQ1.*dQ3.*t2.*t7.*t33.*t34.*t35.*t36.*4.0-Iyy6.*dQ1.*dQ3.*t3.*t8.*t32.*t34.*t35.*t36.*4.0-Iyy6.*dQ1.*dQ4.*t4.*t9.*t32.*t33.*t35.*t36.*4.0-Iyy6.*dQ1.*dQ5.*t5.*t10.*t32.*t33.*t34.*t36.*4.0-Iyy6.*dQ1.*dQ6.*t6.*t11.*t32.*t33.*t34.*t35.*4.0+Iyz5.*dQ1.*dQ2.*t2.*t3.*t5.*t7.*t8.*t9.*4.0+Iyz5.*dQ1.*dQ3.*t2.*t3.*t5.*t7.*t8.*t9.*4.0-Iyz6.*dQ1.*dQ2.*t2.*t3.*t4.*t7.*t8.*t11.*4.0-Iyz6.*dQ1.*dQ3.*t2.*t3.*t4.*t7.*t8.*t11.*4.0-Iyz6.*dQ1.*dQ2.*t2.*t4.*t6.*t7.*t9.*t10.*2.0-Iyz6.*dQ1.*dQ4.*t2.*t3.*t6.*t7.*t8.*t10.*2.0-Iyz6.*dQ1.*dQ3.*t2.*t4.*t6.*t7.*t9.*t10.*2.0-Iyz6.*dQ1.*dQ2.*t3.*t4.*t6.*t8.*t9.*t10.*2.0-Iyz6.*dQ1.*dQ3.*t3.*t4.*t6.*t8.*t9.*t10.*2.0;
et196 = Iyz6.*dQ1.*dQ5.*t2.*t4.*t5.*t7.*t10.*t11.*-4.0-Iyz6.*dQ1.*dQ5.*t3.*t4.*t5.*t8.*t10.*t11.*4.0+Iyz6.*dQ4.*dQ5.*t2.*t4.*t5.*t8.*t10.*t11.*2.0+Iyz6.*dQ4.*dQ5.*t3.*t4.*t5.*t7.*t10.*t11.*2.0-Iyz6.*dQ1.*dQ4.*t2.*t4.*t5.*t6.*t7.*t33.*2.0-Iyz6.*dQ1.*dQ4.*t3.*t4.*t5.*t6.*t8.*t32.*2.0+Iyz5.*dQ1.*dQ2.*t2.*t4.*t7.*t9.*t10.*t33.*4.0+Iyz5.*dQ1.*dQ2.*t3.*t4.*t8.*t9.*t10.*t32.*4.0+Iyz5.*dQ1.*dQ3.*t2.*t4.*t7.*t9.*t10.*t33.*4.0+Iyz5.*dQ1.*dQ4.*t2.*t3.*t7.*t8.*t10.*t34.*4.0+Iyz5.*dQ1.*dQ3.*t3.*t4.*t8.*t9.*t10.*t32.*4.0+Iyz6.*dQ1.*dQ2.*t2.*t5.*t7.*t10.*t11.*t33.*4.0-Iyz6.*dQ1.*dQ5.*t2.*t3.*t7.*t8.*t11.*t34.*2.0-Iyz6.*dQ1.*dQ2.*t2.*t5.*t7.*t10.*t11.*t34.*2.0+Iyz6.*dQ1.*dQ2.*t3.*t5.*t8.*t10.*t11.*t32.*4.0+Iyz6.*dQ1.*dQ3.*t2.*t5.*t7.*t10.*t11.*t33.*4.0+Iyz6.*dQ1.*dQ5.*t2.*t3.*t7.*t8.*t11.*t35.*4.0;
et197 = Iyz6.*dQ1.*dQ3.*t2.*t5.*t7.*t10.*t11.*t34.*-2.0+Iyz6.*dQ1.*dQ3.*t3.*t5.*t8.*t10.*t11.*t32.*4.0+Iyz6.*dQ1.*dQ5.*t2.*t6.*t7.*t9.*t10.*t33.*2.0-Iyz6.*dQ1.*dQ2.*t3.*t5.*t8.*t10.*t11.*t34.*2.0+Iyz6.*dQ1.*dQ5.*t3.*t6.*t8.*t9.*t10.*t32.*2.0+Iyz6.*dQ1.*dQ6.*t2.*t5.*t7.*t9.*t11.*t33.*2.0-Iyz6.*dQ1.*dQ3.*t3.*t5.*t8.*t10.*t11.*t34.*2.0+Iyz6.*dQ1.*dQ6.*t3.*t5.*t8.*t9.*t11.*t32.*2.0-Iyz6.*dQ1.*dQ4.*t4.*t5.*t9.*t10.*t11.*t32.*2.0-Iyz6.*dQ2.*dQ4.*t2.*t5.*t8.*t10.*t11.*t34.*2.0-Iyz6.*dQ2.*dQ4.*t3.*t5.*t7.*t10.*t11.*t34.*2.0-Iyz6.*dQ1.*dQ4.*t4.*t5.*t9.*t10.*t11.*t33.*2.0-Iyz6.*dQ3.*dQ4.*t2.*t5.*t8.*t10.*t11.*t34.*2.0-Iyz6.*dQ3.*dQ4.*t3.*t5.*t7.*t10.*t11.*t34.*2.0-Iyz6.*dQ1.*dQ6.*t2.*t4.*t6.*t7.*t33.*t35.*4.0-Iyz6.*dQ1.*dQ5.*t4.*t5.*t6.*t9.*t32.*t33.*2.0-Iyz6.*dQ1.*dQ6.*t3.*t4.*t6.*t8.*t32.*t35.*4.0;
et198 = Iyz6.*dQ1.*dQ4.*t2.*t7.*t9.*t11.*t33.*t35.*4.0+Iyz6.*dQ1.*dQ4.*t3.*t8.*t9.*t11.*t32.*t35.*4.0+Iyz6.*dQ1.*dQ6.*t4.*t9.*t10.*t11.*t32.*t33.*2.0-Iyz6.*dQ1.*dQ6.*t5.*t6.*t10.*t32.*t33.*t34.*2.0+Izx6.*dQ1.*dQ2.*t2.*t3.*t4.*t6.*t7.*t8.*4.0+Izx6.*dQ1.*dQ3.*t2.*t3.*t4.*t6.*t7.*t8.*4.0+Izx5.*dQ2.*dQ3.*t2.*t3.*t4.*t5.*t9.*t10.*2.0+Izx6.*dQ1.*dQ5.*t2.*t4.*t5.*t6.*t7.*t10.*4.0+Izx6.*dQ1.*dQ5.*t3.*t4.*t5.*t6.*t8.*t10.*4.0-Izx6.*dQ4.*dQ5.*t2.*t4.*t5.*t6.*t8.*t10.*2.0-Izx6.*dQ4.*dQ5.*t3.*t4.*t5.*t6.*t7.*t10.*2.0-Izx6.*dQ1.*dQ2.*t2.*t4.*t7.*t9.*t10.*t11.*2.0-Izx6.*dQ1.*dQ4.*t2.*t3.*t7.*t8.*t10.*t11.*2.0-Izx5.*dQ2.*dQ3.*t4.*t5.*t7.*t8.*t9.*t10.*2.0-Izx6.*dQ1.*dQ3.*t2.*t4.*t7.*t9.*t10.*t11.*2.0-Izx6.*dQ1.*dQ2.*t3.*t4.*t8.*t9.*t10.*t11.*2.0-Izx6.*dQ1.*dQ3.*t3.*t4.*t8.*t9.*t10.*t11.*2.0;
et199 = Izx5.*dQ1.*dQ2.*t2.*t3.*t4.*t7.*t8.*t35.*-8.0-Izx5.*dQ1.*dQ3.*t2.*t3.*t4.*t7.*t8.*t35.*8.0-Izx5.*dQ1.*dQ5.*t2.*t4.*t5.*t7.*t10.*t33.*8.0-Izx6.*dQ1.*dQ2.*t2.*t5.*t6.*t7.*t10.*t33.*4.0+Izx6.*dQ1.*dQ5.*t2.*t3.*t6.*t7.*t8.*t34.*2.0-Izx5.*dQ1.*dQ5.*t3.*t4.*t5.*t8.*t10.*t32.*8.0+Izx6.*dQ1.*dQ2.*t2.*t5.*t6.*t7.*t10.*t34.*2.0-Izx6.*dQ1.*dQ2.*t3.*t5.*t6.*t8.*t10.*t32.*4.0-Izx6.*dQ1.*dQ3.*t2.*t5.*t6.*t7.*t10.*t33.*4.0-Izx6.*dQ1.*dQ4.*t2.*t4.*t5.*t7.*t11.*t33.*2.0-Izx6.*dQ1.*dQ5.*t2.*t3.*t6.*t7.*t8.*t35.*4.0+Izx6.*dQ1.*dQ3.*t2.*t5.*t6.*t7.*t10.*t34.*2.0-Izx6.*dQ1.*dQ3.*t3.*t5.*t6.*t8.*t10.*t32.*4.0-Izx6.*dQ1.*dQ4.*t3.*t4.*t5.*t8.*t11.*t32.*2.0+Izx6.*dQ1.*dQ2.*t3.*t5.*t6.*t8.*t10.*t34.*2.0-Izx6.*dQ1.*dQ6.*t2.*t5.*t6.*t7.*t9.*t33.*2.0;
et200 = Izx6.*dQ1.*dQ3.*t3.*t5.*t6.*t8.*t10.*t34.*2.0-Izx6.*dQ1.*dQ6.*t3.*t5.*t6.*t8.*t9.*t32.*2.0+Izx6.*dQ1.*dQ4.*t4.*t5.*t6.*t9.*t10.*t32.*2.0+Izx6.*dQ2.*dQ4.*t2.*t5.*t6.*t8.*t10.*t34.*2.0+Izx6.*dQ2.*dQ4.*t3.*t5.*t6.*t7.*t10.*t34.*2.0+Izx6.*dQ1.*dQ4.*t4.*t5.*t6.*t9.*t10.*t33.*2.0+Izx6.*dQ3.*dQ4.*t2.*t5.*t6.*t8.*t10.*t34.*2.0+Izx6.*dQ3.*dQ4.*t3.*t5.*t6.*t7.*t10.*t34.*2.0+Izx6.*dQ1.*dQ5.*t2.*t7.*t9.*t10.*t11.*t33.*2.0+Izx6.*dQ1.*dQ5.*t3.*t8.*t9.*t10.*t11.*t32.*2.0-Izx5.*dQ1.*dQ2.*t2.*t5.*t7.*t10.*t33.*t34.*4.0-Izx5.*dQ1.*dQ2.*t3.*t5.*t8.*t10.*t32.*t34.*4.0-Izx5.*dQ1.*dQ3.*t2.*t5.*t7.*t10.*t33.*t34.*4.0-Izx5.*dQ1.*dQ5.*t2.*t3.*t7.*t8.*t34.*t35.*4.0-Izx5.*dQ1.*dQ3.*t3.*t5.*t8.*t10.*t32.*t34.*4.0-Izx5.*dQ1.*dQ4.*t4.*t5.*t9.*t10.*t32.*t33.*4.0-Izx6.*dQ1.*dQ4.*t2.*t6.*t7.*t9.*t33.*t35.*4.0;
et201 = Izx6.*dQ1.*dQ4.*t3.*t6.*t8.*t9.*t32.*t35.*-4.0-Izx6.*dQ1.*dQ6.*t2.*t4.*t7.*t11.*t33.*t35.*4.0-Izx6.*dQ1.*dQ5.*t4.*t5.*t9.*t11.*t32.*t33.*2.0-Izx6.*dQ1.*dQ6.*t3.*t4.*t8.*t11.*t32.*t35.*4.0-Izx6.*dQ1.*dQ6.*t4.*t6.*t9.*t10.*t32.*t33.*2.0-Izx6.*dQ1.*dQ6.*t5.*t10.*t11.*t32.*t33.*t34.*2.0+Izy5.*dQ1.*dQ2.*t2.*t3.*t5.*t7.*t8.*t9.*4.0+Izy5.*dQ1.*dQ3.*t2.*t3.*t5.*t7.*t8.*t9.*4.0-Izy6.*dQ1.*dQ2.*t2.*t3.*t4.*t7.*t8.*t11.*4.0-Izy6.*dQ1.*dQ3.*t2.*t3.*t4.*t7.*t8.*t11.*4.0-Izy6.*dQ1.*dQ2.*t2.*t4.*t6.*t7.*t9.*t10.*2.0-Izy6.*dQ1.*dQ4.*t2.*t3.*t6.*t7.*t8.*t10.*2.0-Izy6.*dQ1.*dQ3.*t2.*t4.*t6.*t7.*t9.*t10.*2.0-Izy6.*dQ1.*dQ2.*t3.*t4.*t6.*t8.*t9.*t10.*2.0-Izy6.*dQ1.*dQ3.*t3.*t4.*t6.*t8.*t9.*t10.*2.0-Izy6.*dQ1.*dQ5.*t2.*t4.*t5.*t7.*t10.*t11.*4.0;
et202 = Izy6.*dQ1.*dQ5.*t3.*t4.*t5.*t8.*t10.*t11.*-4.0+Izy6.*dQ4.*dQ5.*t2.*t4.*t5.*t8.*t10.*t11.*2.0+Izy6.*dQ4.*dQ5.*t3.*t4.*t5.*t7.*t10.*t11.*2.0-Izy6.*dQ1.*dQ4.*t2.*t4.*t5.*t6.*t7.*t33.*2.0-Izy6.*dQ1.*dQ4.*t3.*t4.*t5.*t6.*t8.*t32.*2.0+Izy5.*dQ1.*dQ2.*t2.*t4.*t7.*t9.*t10.*t33.*4.0+Izy5.*dQ1.*dQ2.*t3.*t4.*t8.*t9.*t10.*t32.*4.0+Izy5.*dQ1.*dQ3.*t2.*t4.*t7.*t9.*t10.*t33.*4.0+Izy5.*dQ1.*dQ4.*t2.*t3.*t7.*t8.*t10.*t34.*4.0+Izy5.*dQ1.*dQ3.*t3.*t4.*t8.*t9.*t10.*t32.*4.0+Izy6.*dQ1.*dQ2.*t2.*t5.*t7.*t10.*t11.*t33.*4.0-Izy6.*dQ1.*dQ5.*t2.*t3.*t7.*t8.*t11.*t34.*2.0-Izy6.*dQ1.*dQ2.*t2.*t5.*t7.*t10.*t11.*t34.*2.0+Izy6.*dQ1.*dQ2.*t3.*t5.*t8.*t10.*t11.*t32.*4.0+Izy6.*dQ1.*dQ3.*t2.*t5.*t7.*t10.*t11.*t33.*4.0+Izy6.*dQ1.*dQ5.*t2.*t3.*t7.*t8.*t11.*t35.*4.0-Izy6.*dQ1.*dQ3.*t2.*t5.*t7.*t10.*t11.*t34.*2.0;
et203 = Izy6.*dQ1.*dQ3.*t3.*t5.*t8.*t10.*t11.*t32.*4.0+Izy6.*dQ1.*dQ5.*t2.*t6.*t7.*t9.*t10.*t33.*2.0-Izy6.*dQ1.*dQ2.*t3.*t5.*t8.*t10.*t11.*t34.*2.0+Izy6.*dQ1.*dQ5.*t3.*t6.*t8.*t9.*t10.*t32.*2.0+Izy6.*dQ1.*dQ6.*t2.*t5.*t7.*t9.*t11.*t33.*2.0-Izy6.*dQ1.*dQ3.*t3.*t5.*t8.*t10.*t11.*t34.*2.0+Izy6.*dQ1.*dQ6.*t3.*t5.*t8.*t9.*t11.*t32.*2.0-Izy6.*dQ1.*dQ4.*t4.*t5.*t9.*t10.*t11.*t32.*2.0-Izy6.*dQ2.*dQ4.*t2.*t5.*t8.*t10.*t11.*t34.*2.0-Izy6.*dQ2.*dQ4.*t3.*t5.*t7.*t10.*t11.*t34.*2.0-Izy6.*dQ1.*dQ4.*t4.*t5.*t9.*t10.*t11.*t33.*2.0-Izy6.*dQ3.*dQ4.*t2.*t5.*t8.*t10.*t11.*t34.*2.0-Izy6.*dQ3.*dQ4.*t3.*t5.*t7.*t10.*t11.*t34.*2.0-Izy6.*dQ1.*dQ6.*t2.*t4.*t6.*t7.*t33.*t35.*4.0-Izy6.*dQ1.*dQ5.*t4.*t5.*t6.*t9.*t32.*t33.*2.0-Izy6.*dQ1.*dQ6.*t3.*t4.*t6.*t8.*t32.*t35.*4.0+Izy6.*dQ1.*dQ4.*t2.*t7.*t9.*t11.*t33.*t35.*4.0;
et204 = Izy6.*dQ1.*dQ4.*t3.*t8.*t9.*t11.*t32.*t35.*4.0+Izy6.*dQ1.*dQ6.*t4.*t9.*t10.*t11.*t32.*t33.*2.0-Izy6.*dQ1.*dQ6.*t5.*t6.*t10.*t32.*t33.*t34.*2.0+Izz5.*dQ1.*dQ5.*t2.*t3.*t5.*t7.*t8.*t10.*4.0+Izz6.*dQ1.*dQ5.*t2.*t3.*t5.*t7.*t8.*t10.*4.0-Izz5.*dQ2.*dQ5.*t2.*t4.*t5.*t8.*t9.*t10.*2.0-Izz5.*dQ2.*dQ5.*t3.*t4.*t5.*t7.*t9.*t10.*2.0-Izz5.*dQ3.*dQ5.*t2.*t4.*t5.*t8.*t9.*t10.*2.0-Izz5.*dQ3.*dQ5.*t3.*t4.*t5.*t7.*t9.*t10.*2.0-Izz6.*dQ2.*dQ5.*t2.*t4.*t5.*t8.*t9.*t10.*2.0-Izz6.*dQ2.*dQ5.*t3.*t4.*t5.*t7.*t9.*t10.*2.0-Izz6.*dQ3.*dQ5.*t2.*t4.*t5.*t8.*t9.*t10.*2.0-Izz6.*dQ3.*dQ5.*t3.*t4.*t5.*t7.*t9.*t10.*2.0+Izz5.*dQ1.*dQ4.*t2.*t5.*t7.*t9.*t10.*t33.*4.0+Izz5.*dQ1.*dQ4.*t3.*t5.*t8.*t9.*t10.*t32.*4.0+Izz6.*dQ1.*dQ4.*t2.*t5.*t7.*t9.*t10.*t33.*4.0+Izz6.*dQ1.*dQ4.*t3.*t5.*t8.*t9.*t10.*t32.*4.0;
et205 = dQ2.*dQ3.*m6.*t2.*t3.*t5.*t6.*t11.*t17.*-2.0+dQ2.*dQ3.*m6.*t2.*t3.*t5.*t6.*t11.*t20.*2.0-dQ1.*dQ4.*m5.*t2.*t5.*t7.*t9.*t10.*t16.*2.0-dQ2.*dQ3.*m5.*t2.*t5.*t8.*t9.*t10.*t16.*2.0-dQ2.*dQ3.*m5.*t3.*t5.*t7.*t9.*t10.*t16.*2.0-dQ1.*dQ4.*m5.*t3.*t5.*t8.*t9.*t10.*t16.*2.0-dQ1.*dQ4.*m6.*t2.*t5.*t7.*t9.*t10.*t20.*2.0-dQ2.*dQ3.*m6.*t2.*t5.*t8.*t9.*t10.*t20.*2.0-dQ2.*dQ3.*m6.*t3.*t5.*t7.*t9.*t10.*t20.*2.0+dQ2.*dQ3.*m6.*t5.*t6.*t7.*t8.*t11.*t17.*2.0+dQ1.*dQ4.*m6.*t2.*t5.*t7.*t9.*t10.*t22.*2.0-dQ1.*dQ4.*m6.*t3.*t5.*t8.*t9.*t10.*t20.*2.0+dQ2.*dQ3.*m6.*t2.*t5.*t8.*t9.*t10.*t22.*2.0+dQ2.*dQ3.*m6.*t3.*t5.*t7.*t9.*t10.*t22.*2.0+dQ1.*dQ4.*m5.*t2.*t5.*t7.*t9.*t10.*t25.*2.0+dQ1.*dQ4.*m6.*t3.*t5.*t8.*t9.*t10.*t22.*2.0-dQ2.*dQ3.*m6.*t5.*t6.*t7.*t8.*t11.*t20.*2.0;
et206 = dQ2.*dQ3.*m5.*t2.*t5.*t8.*t9.*t10.*t25.*2.0+dQ2.*dQ3.*m5.*t3.*t5.*t7.*t9.*t10.*t25.*2.0+dQ1.*dQ4.*m5.*t3.*t5.*t8.*t9.*t10.*t25.*2.0+dQ1.*dQ4.*m6.*t2.*t5.*t7.*t9.*t10.*t26.*2.0-dQ5.*dQ6.*m6.*t2.*t6.*t8.*t9.*t11.*t17.*2.0-dQ5.*dQ6.*m6.*t3.*t6.*t7.*t9.*t11.*t17.*2.0+dQ2.*dQ3.*m6.*t2.*t5.*t8.*t9.*t10.*t26.*2.0+dQ2.*dQ3.*m6.*t3.*t5.*t7.*t9.*t10.*t26.*2.0+dQ1.*dQ4.*m6.*t3.*t5.*t8.*t9.*t10.*t26.*2.0+dQ5.*dQ6.*m6.*t2.*t6.*t8.*t9.*t11.*t20.*2.0+dQ5.*dQ6.*m6.*t3.*t6.*t7.*t9.*t11.*t20.*2.0+dQ2.*dQ3.*m5.*t2.*t3.*t4.*t9.*t16.*t35.*2.0+dQ2.*dQ3.*m6.*t2.*t3.*t4.*t9.*t17.*t36.*2.0+dQ2.*dQ3.*m6.*t2.*t3.*t4.*t9.*t20.*t35.*2.0-dQ2.*dQ3.*m6.*t2.*t3.*t4.*t9.*t20.*t36.*2.0-dQ2.*dQ3.*m6.*t2.*t3.*t4.*t9.*t22.*t35.*2.0+dQ2.*dQ6.*m6.*t2.*t3.*t4.*t10.*t17.*t36.*2.0;
et207 = dQ3.*dQ6.*m6.*t2.*t3.*t4.*t10.*t17.*t36.*2.0-dQ2.*dQ3.*m5.*t2.*t3.*t4.*t9.*t25.*t35.*2.0-dQ4.*dQ5.*m6.*t2.*t3.*t5.*t10.*t17.*t36.*2.0-dQ2.*dQ3.*m5.*t4.*t7.*t8.*t9.*t16.*t35.*2.0-dQ2.*dQ6.*m6.*t2.*t3.*t4.*t10.*t20.*t36.*2.0+dQ5.*dQ6.*m6.*t2.*t4.*t5.*t8.*t17.*t36.*2.0+dQ5.*dQ6.*m6.*t3.*t4.*t5.*t7.*t17.*t36.*2.0-dQ2.*dQ3.*m6.*t2.*t3.*t4.*t9.*t26.*t35.*2.0-dQ3.*dQ6.*m6.*t2.*t3.*t4.*t10.*t20.*t36.*2.0-dQ4.*dQ6.*m6.*t2.*t3.*t6.*t11.*t17.*t35.*2.0-dQ1.*dQ6.*m6.*t2.*t7.*t9.*t10.*t17.*t33.*4.0+dQ4.*dQ5.*m6.*t2.*t3.*t5.*t10.*t20.*t36.*2.0-dQ1.*dQ6.*m6.*t3.*t8.*t9.*t10.*t17.*t32.*4.0-dQ2.*dQ3.*m6.*t4.*t7.*t8.*t9.*t17.*t36.*2.0-dQ5.*dQ6.*m6.*t2.*t4.*t5.*t8.*t20.*t36.*2.0-dQ5.*dQ6.*m6.*t3.*t4.*t5.*t7.*t20.*t36.*2.0+dQ4.*dQ6.*m6.*t2.*t3.*t6.*t11.*t20.*t35.*2.0;
et208 = dQ1.*dQ2.*m6.*t6.*t9.*t10.*t11.*t17.*t32.*-4.0-dQ1.*dQ6.*m6.*t2.*t7.*t9.*t10.*t17.*t36.*4.0+dQ1.*dQ6.*m6.*t2.*t7.*t9.*t10.*t20.*t33.*4.0-dQ2.*dQ3.*m6.*t4.*t7.*t8.*t9.*t20.*t35.*2.0-dQ1.*dQ2.*m6.*t6.*t9.*t10.*t11.*t17.*t33.*4.0-dQ1.*dQ3.*m6.*t6.*t9.*t10.*t11.*t17.*t32.*4.0+dQ1.*dQ6.*m6.*t3.*t8.*t9.*t10.*t20.*t32.*4.0+dQ2.*dQ3.*m6.*t4.*t7.*t8.*t9.*t20.*t36.*2.0-dQ1.*dQ3.*m6.*t6.*t9.*t10.*t11.*t17.*t33.*4.0-dQ1.*dQ6.*m6.*t3.*t8.*t9.*t10.*t17.*t36.*4.0+dQ2.*dQ3.*m6.*t4.*t7.*t8.*t9.*t22.*t35.*2.0-dQ2.*dQ6.*m6.*t4.*t7.*t8.*t10.*t17.*t36.*2.0+dQ1.*dQ2.*m6.*t6.*t9.*t10.*t11.*t20.*t32.*4.0+dQ1.*dQ6.*m6.*t2.*t7.*t9.*t10.*t20.*t36.*4.0-dQ3.*dQ6.*m6.*t4.*t7.*t8.*t10.*t17.*t36.*2.0+dQ1.*dQ2.*m6.*t6.*t9.*t10.*t11.*t20.*t33.*4.0+dQ1.*dQ3.*m6.*t6.*t9.*t10.*t11.*t20.*t32.*4.0;
et209 = dQ2.*dQ3.*m5.*t4.*t7.*t8.*t9.*t25.*t35.*2.0+dQ4.*dQ5.*m6.*t5.*t7.*t8.*t10.*t17.*t36.*2.0+dQ4.*dQ6.*m6.*t2.*t8.*t9.*t10.*t17.*t36.*2.0+dQ4.*dQ6.*m6.*t3.*t7.*t9.*t10.*t17.*t36.*2.0+dQ1.*dQ3.*m6.*t6.*t9.*t10.*t11.*t20.*t33.*4.0+dQ1.*dQ6.*m6.*t3.*t8.*t9.*t10.*t20.*t36.*4.0+dQ2.*dQ6.*m6.*t4.*t7.*t8.*t10.*t20.*t36.*2.0+dQ2.*dQ3.*m6.*t4.*t7.*t8.*t9.*t26.*t35.*2.0+dQ3.*dQ6.*m6.*t4.*t7.*t8.*t10.*t20.*t36.*2.0+dQ4.*dQ6.*m6.*t6.*t7.*t8.*t11.*t17.*t35.*2.0-dQ4.*dQ5.*m6.*t5.*t7.*t8.*t10.*t20.*t36.*2.0-dQ4.*dQ6.*m6.*t2.*t8.*t9.*t10.*t20.*t36.*2.0-dQ4.*dQ6.*m6.*t3.*t7.*t9.*t10.*t20.*t36.*2.0-dQ4.*dQ6.*m6.*t6.*t7.*t8.*t11.*t20.*t35.*2.0-dQ1.*dQ2.*m5.*t4.*t5.*t10.*t16.*t32.*t33.*8.0-dQ1.*dQ5.*m5.*t2.*t4.*t7.*t16.*t33.*t35.*8.0-dQ1.*dQ3.*m5.*t4.*t5.*t10.*t16.*t32.*t33.*8.0;
et210 = dQ1.*dQ5.*m5.*t3.*t4.*t8.*t16.*t32.*t35.*-8.0+dQ1.*dQ5.*m6.*t2.*t4.*t7.*t17.*t33.*t36.*4.0+dQ1.*dQ5.*m6.*t3.*t4.*t8.*t17.*t32.*t36.*4.0+dQ1.*dQ2.*m6.*t4.*t5.*t10.*t17.*t32.*t36.*4.0-dQ1.*dQ2.*m6.*t4.*t5.*t10.*t20.*t32.*t33.*8.0+dQ1.*dQ5.*m6.*t2.*t4.*t7.*t17.*t35.*t36.*4.0-dQ1.*dQ5.*m6.*t2.*t4.*t7.*t20.*t33.*t35.*8.0+dQ1.*dQ6.*m6.*t4.*t5.*t9.*t17.*t32.*t33.*4.0+dQ1.*dQ2.*m6.*t4.*t5.*t10.*t17.*t33.*t36.*4.0+dQ1.*dQ3.*m6.*t4.*t5.*t10.*t17.*t32.*t36.*4.0-dQ1.*dQ3.*m6.*t4.*t5.*t10.*t20.*t32.*t33.*8.0-dQ1.*dQ5.*m6.*t2.*t4.*t7.*t20.*t33.*t36.*4.0-dQ1.*dQ5.*m6.*t3.*t4.*t8.*t20.*t32.*t35.*8.0+dQ1.*dQ2.*m6.*t4.*t5.*t10.*t22.*t32.*t33.*8.0+dQ1.*dQ3.*m6.*t4.*t5.*t10.*t17.*t33.*t36.*4.0+dQ1.*dQ4.*m6.*t5.*t6.*t11.*t17.*t32.*t33.*4.0+dQ1.*dQ5.*m6.*t2.*t4.*t7.*t22.*t33.*t35.*8.0;
et211 = dQ1.*dQ5.*m6.*t3.*t4.*t8.*t17.*t35.*t36.*4.0-dQ1.*dQ5.*m6.*t3.*t4.*t8.*t20.*t32.*t36.*4.0+dQ2.*dQ5.*m6.*t2.*t3.*t9.*t17.*t35.*t36.*2.0-dQ1.*dQ2.*m6.*t4.*t5.*t10.*t20.*t32.*t36.*4.0+dQ1.*dQ3.*m6.*t4.*t5.*t10.*t22.*t32.*t33.*8.0+dQ1.*dQ4.*m6.*t5.*t6.*t11.*t17.*t32.*t34.*4.0-dQ1.*dQ5.*m6.*t2.*t4.*t7.*t20.*t35.*t36.*4.0+dQ1.*dQ5.*m6.*t3.*t4.*t8.*t22.*t32.*t35.*8.0+dQ1.*dQ6.*m6.*t4.*t5.*t9.*t17.*t32.*t36.*4.0-dQ1.*dQ6.*m6.*t4.*t5.*t9.*t20.*t32.*t33.*4.0+dQ2.*dQ6.*m6.*t2.*t5.*t8.*t17.*t34.*t36.*4.0+dQ2.*dQ6.*m6.*t3.*t5.*t7.*t17.*t34.*t36.*4.0+dQ3.*dQ5.*m6.*t2.*t3.*t9.*t17.*t35.*t36.*2.0+dQ1.*dQ2.*m5.*t4.*t5.*t10.*t25.*t32.*t33.*8.0-dQ1.*dQ2.*m6.*t4.*t5.*t10.*t20.*t33.*t36.*4.0-dQ1.*dQ3.*m6.*t4.*t5.*t10.*t20.*t32.*t36.*4.0+dQ1.*dQ4.*m6.*t5.*t6.*t11.*t17.*t33.*t34.*4.0;
et212 = dQ1.*dQ5.*m5.*t2.*t4.*t7.*t25.*t33.*t35.*8.0+dQ1.*dQ6.*m6.*t4.*t5.*t9.*t17.*t33.*t36.*4.0+dQ3.*dQ6.*m6.*t2.*t5.*t8.*t17.*t34.*t36.*4.0+dQ3.*dQ6.*m6.*t3.*t5.*t7.*t17.*t34.*t36.*4.0-dQ4.*dQ5.*m6.*t2.*t4.*t8.*t17.*t35.*t36.*2.0-dQ4.*dQ5.*m6.*t3.*t4.*t7.*t17.*t35.*t36.*2.0+dQ1.*dQ3.*m5.*t4.*t5.*t10.*t25.*t32.*t33.*8.0-dQ1.*dQ3.*m6.*t4.*t5.*t10.*t20.*t33.*t36.*4.0-dQ1.*dQ4.*m6.*t5.*t6.*t11.*t20.*t32.*t33.*4.0+dQ1.*dQ5.*m5.*t3.*t4.*t8.*t25.*t32.*t35.*8.0-dQ1.*dQ5.*m6.*t3.*t4.*t8.*t20.*t35.*t36.*4.0-dQ2.*dQ5.*m6.*t2.*t3.*t9.*t20.*t35.*t36.*2.0+dQ1.*dQ2.*m6.*t4.*t5.*t10.*t26.*t32.*t33.*8.0-dQ1.*dQ4.*m6.*t5.*t6.*t11.*t20.*t32.*t34.*4.0+dQ1.*dQ5.*m6.*t2.*t4.*t7.*t26.*t33.*t35.*8.0-dQ1.*dQ6.*m6.*t4.*t5.*t9.*t20.*t32.*t36.*4.0;
et213 = dQ2.*dQ6.*m6.*t2.*t5.*t8.*t20.*t34.*t36.*-4.0-dQ2.*dQ6.*m6.*t3.*t5.*t7.*t20.*t34.*t36.*4.0-dQ3.*dQ5.*m6.*t2.*t3.*t9.*t20.*t35.*t36.*2.0+dQ1.*dQ3.*m6.*t4.*t5.*t10.*t26.*t32.*t33.*8.0-dQ1.*dQ4.*m6.*t5.*t6.*t11.*t20.*t33.*t34.*4.0+dQ1.*dQ5.*m6.*t3.*t4.*t8.*t26.*t32.*t35.*8.0-dQ1.*dQ6.*m6.*t4.*t5.*t9.*t20.*t33.*t36.*4.0-dQ3.*dQ6.*m6.*t2.*t5.*t8.*t20.*t34.*t36.*4.0-dQ3.*dQ6.*m6.*t3.*t5.*t7.*t20.*t34.*t36.*4.0+dQ4.*dQ5.*m6.*t2.*t4.*t8.*t20.*t35.*t36.*2.0+dQ4.*dQ5.*m6.*t3.*t4.*t7.*t20.*t35.*t36.*2.0-dQ2.*dQ5.*m6.*t7.*t8.*t9.*t17.*t35.*t36.*2.0-dQ3.*dQ5.*m6.*t7.*t8.*t9.*t17.*t35.*t36.*2.0+dQ2.*dQ5.*m6.*t7.*t8.*t9.*t20.*t35.*t36.*2.0+dQ3.*dQ5.*m6.*t7.*t8.*t9.*t20.*t35.*t36.*2.0-dQ1.*dQ2.*m5.*t2.*t7.*t16.*t33.*t34.*t35.*4.0-dQ1.*dQ2.*m5.*t3.*t8.*t16.*t32.*t34.*t35.*4.0;
et214 = dQ1.*dQ3.*m5.*t2.*t7.*t16.*t33.*t34.*t35.*-4.0-dQ1.*dQ3.*m5.*t3.*t8.*t16.*t32.*t34.*t35.*4.0-dQ1.*dQ2.*m6.*t2.*t7.*t17.*t33.*t34.*t36.*4.0-dQ1.*dQ2.*m6.*t2.*t7.*t17.*t33.*t35.*t36.*4.0-dQ1.*dQ2.*m6.*t3.*t8.*t17.*t32.*t34.*t36.*4.0-dQ1.*dQ3.*m6.*t2.*t7.*t17.*t33.*t34.*t36.*4.0-dQ1.*dQ4.*m5.*t4.*t9.*t16.*t32.*t33.*t35.*4.0+dQ1.*dQ2.*m6.*t2.*t7.*t17.*t34.*t35.*t36.*2.0-dQ1.*dQ2.*m6.*t2.*t7.*t20.*t33.*t34.*t35.*4.0-dQ1.*dQ2.*m6.*t3.*t8.*t17.*t32.*t35.*t36.*4.0-dQ1.*dQ3.*m6.*t2.*t7.*t17.*t33.*t35.*t36.*4.0-dQ1.*dQ3.*m6.*t3.*t8.*t17.*t32.*t34.*t36.*4.0+dQ1.*dQ2.*m6.*t2.*t7.*t20.*t33.*t34.*t36.*4.0-dQ1.*dQ2.*m6.*t3.*t8.*t20.*t32.*t34.*t35.*4.0+dQ1.*dQ3.*m6.*t2.*t7.*t17.*t34.*t35.*t36.*2.0-dQ1.*dQ3.*m6.*t2.*t7.*t20.*t33.*t34.*t35.*4.0;
et215 = dQ1.*dQ3.*m6.*t3.*t8.*t17.*t32.*t35.*t36.*-4.0-dQ1.*dQ5.*m5.*t5.*t10.*t16.*t32.*t33.*t34.*4.0+dQ1.*dQ2.*m6.*t2.*t7.*t20.*t33.*t35.*t36.*4.0+dQ1.*dQ2.*m6.*t2.*t7.*t22.*t33.*t34.*t35.*4.0+dQ1.*dQ2.*m6.*t3.*t8.*t17.*t34.*t35.*t36.*2.0+dQ1.*dQ2.*m6.*t3.*t8.*t20.*t32.*t34.*t36.*4.0+dQ1.*dQ3.*m6.*t2.*t7.*t20.*t33.*t34.*t36.*4.0-dQ1.*dQ3.*m6.*t3.*t8.*t20.*t32.*t34.*t35.*4.0-dQ1.*dQ4.*m6.*t4.*t9.*t17.*t32.*t33.*t36.*4.0-dQ1.*dQ2.*m6.*t2.*t7.*t20.*t34.*t35.*t36.*2.0+dQ1.*dQ2.*m6.*t3.*t8.*t20.*t32.*t35.*t36.*4.0+dQ1.*dQ2.*m6.*t3.*t8.*t22.*t32.*t34.*t35.*4.0+dQ1.*dQ3.*m6.*t2.*t7.*t20.*t33.*t35.*t36.*4.0+dQ1.*dQ3.*m6.*t2.*t7.*t22.*t33.*t34.*t35.*4.0+dQ1.*dQ3.*m6.*t3.*t8.*t17.*t34.*t35.*t36.*2.0+dQ1.*dQ3.*m6.*t3.*t8.*t20.*t32.*t34.*t36.*4.0+dQ1.*dQ2.*m5.*t2.*t7.*t25.*t33.*t34.*t35.*4.0;
et216 = dQ1.*dQ3.*m6.*t2.*t7.*t20.*t34.*t35.*t36.*-2.0+dQ1.*dQ3.*m6.*t3.*t8.*t20.*t32.*t35.*t36.*4.0+dQ1.*dQ3.*m6.*t3.*t8.*t22.*t32.*t34.*t35.*4.0+dQ1.*dQ4.*m6.*t4.*t9.*t17.*t32.*t35.*t36.*2.0-dQ1.*dQ4.*m6.*t4.*t9.*t20.*t32.*t33.*t35.*4.0+dQ2.*dQ4.*m6.*t2.*t8.*t17.*t34.*t35.*t36.*2.0+dQ2.*dQ4.*m6.*t3.*t7.*t17.*t34.*t35.*t36.*2.0+dQ1.*dQ2.*m5.*t3.*t8.*t25.*t32.*t34.*t35.*4.0-dQ1.*dQ2.*m6.*t3.*t8.*t20.*t34.*t35.*t36.*2.0+dQ1.*dQ3.*m5.*t2.*t7.*t25.*t33.*t34.*t35.*4.0+dQ1.*dQ4.*m6.*t4.*t9.*t17.*t33.*t35.*t36.*2.0+dQ1.*dQ4.*m6.*t4.*t9.*t20.*t32.*t33.*t36.*4.0-dQ1.*dQ5.*m6.*t5.*t10.*t17.*t32.*t33.*t36.*4.0+dQ3.*dQ4.*m6.*t2.*t8.*t17.*t34.*t35.*t36.*2.0+dQ3.*dQ4.*m6.*t3.*t7.*t17.*t34.*t35.*t36.*2.0+dQ1.*dQ2.*m6.*t2.*t7.*t26.*t33.*t34.*t35.*4.0+dQ1.*dQ3.*m5.*t3.*t8.*t25.*t32.*t34.*t35.*4.0;
et217 = dQ1.*dQ3.*m6.*t3.*t8.*t20.*t34.*t35.*t36.*-2.0+dQ1.*dQ4.*m6.*t4.*t9.*t22.*t32.*t33.*t35.*4.0+dQ1.*dQ5.*m6.*t5.*t10.*t17.*t32.*t34.*t36.*2.0-dQ1.*dQ5.*m6.*t5.*t10.*t20.*t32.*t33.*t34.*4.0-dQ1.*dQ6.*m6.*t6.*t11.*t17.*t32.*t33.*t34.*4.0+dQ1.*dQ2.*m6.*t3.*t8.*t26.*t32.*t34.*t35.*4.0+dQ1.*dQ3.*m6.*t2.*t7.*t26.*t33.*t34.*t35.*4.0-dQ1.*dQ4.*m6.*t4.*t9.*t20.*t32.*t35.*t36.*2.0+dQ1.*dQ5.*m6.*t5.*t10.*t17.*t33.*t34.*t36.*2.0-dQ1.*dQ6.*m6.*t6.*t11.*t17.*t32.*t33.*t35.*4.0-dQ2.*dQ4.*m6.*t2.*t8.*t20.*t34.*t35.*t36.*2.0-dQ2.*dQ4.*m6.*t3.*t7.*t20.*t34.*t35.*t36.*2.0+dQ1.*dQ3.*m6.*t3.*t8.*t26.*t32.*t34.*t35.*4.0+dQ1.*dQ4.*m5.*t4.*t9.*t25.*t32.*t33.*t35.*4.0-dQ1.*dQ4.*m6.*t4.*t9.*t20.*t33.*t35.*t36.*2.0+dQ1.*dQ5.*m6.*t5.*t10.*t20.*t32.*t33.*t36.*4.0+dQ1.*dQ5.*m6.*t5.*t10.*t22.*t32.*t33.*t34.*4.0;
et218 = dQ1.*dQ6.*m6.*t6.*t11.*t17.*t32.*t34.*t35.*2.0-dQ3.*dQ4.*m6.*t2.*t8.*t20.*t34.*t35.*t36.*2.0-dQ3.*dQ4.*m6.*t3.*t7.*t20.*t34.*t35.*t36.*2.0-dQ1.*dQ5.*m6.*t5.*t10.*t20.*t32.*t34.*t36.*2.0+dQ1.*dQ6.*m6.*t6.*t11.*t17.*t33.*t34.*t35.*2.0+dQ1.*dQ6.*m6.*t6.*t11.*t20.*t32.*t33.*t34.*4.0+dQ1.*dQ4.*m6.*t4.*t9.*t26.*t32.*t33.*t35.*4.0+dQ1.*dQ5.*m5.*t5.*t10.*t25.*t32.*t33.*t34.*4.0-dQ1.*dQ5.*m6.*t5.*t10.*t20.*t33.*t34.*t36.*2.0+dQ1.*dQ6.*m6.*t6.*t11.*t20.*t32.*t33.*t35.*4.0-dQ1.*dQ6.*m6.*t6.*t11.*t20.*t32.*t34.*t35.*2.0+dQ1.*dQ5.*m6.*t5.*t10.*t26.*t32.*t33.*t34.*4.0-dQ1.*dQ6.*m6.*t6.*t11.*t20.*t33.*t34.*t35.*2.0-Lx2.*Lxcm4.*dQ1.*dQ2.*m4.*t2.*t3.*t4.*t7.*4.0-Lx2.*Lxcm4.*dQ1.*dQ3.*m4.*t2.*t3.*t4.*t7.*2.0+Lx3.*Lxcm5.*dQ1.*dQ2.*m5.*t2.*t4.*t5.*t7.*4.0-Lx2.*Lxcm5.*dQ1.*dQ5.*m5.*t2.*t3.*t5.*t7.*2.0;
et219 = Lx3.*Lxcm5.*dQ1.*dQ3.*m5.*t2.*t4.*t5.*t7.*4.0+Lx3.*Lxcm5.*dQ1.*dQ2.*m5.*t3.*t4.*t5.*t8.*4.0+Lx3.*Lxcm5.*dQ1.*dQ3.*m5.*t3.*t4.*t5.*t8.*4.0+Lx3.*Lxcm5.*dQ2.*dQ3.*m5.*t2.*t3.*t5.*t9.*2.0+Lx2.*Lxcm6.*dQ1.*dQ2.*m6.*t4.*t5.*t6.*t8.*2.0+Lx3.*Lxcm6.*dQ2.*dQ3.*m6.*t2.*t3.*t4.*t11.*2.0+Lx2.*Lxcm4.*dQ1.*dQ4.*m4.*t2.*t7.*t8.*t9.*2.0-Lx3.*Lxcm5.*dQ4.*dQ5.*m5.*t2.*t3.*t4.*t10.*2.0+Lx3.*Lxcm6.*dQ1.*dQ5.*m6.*t2.*t5.*t6.*t7.*2.0+Lx2.*Lxcm5.*dQ1.*dQ2.*m5.*t2.*t7.*t8.*t10.*4.0+Lx2.*Lxcm5.*dQ1.*dQ3.*m5.*t2.*t7.*t8.*t10.*2.0+Lx3.*Lxcm6.*dQ1.*dQ5.*m6.*t3.*t5.*t6.*t8.*2.0-Lx2.*Lxcm6.*dQ4.*dQ5.*m6.*t2.*t4.*t6.*t10.*2.0-Lx3.*Lxcm6.*dQ4.*dQ6.*m6.*t2.*t3.*t6.*t9.*2.0-Lx2.*Lxcm6.*dQ4.*dQ6.*m6.*t2.*t4.*t5.*t11.*2.0-Lx3.*Lxcm5.*dQ2.*dQ3.*m5.*t5.*t7.*t8.*t9.*2.0-Lx3.*Lxcm6.*dQ1.*dQ2.*m6.*t2.*t7.*t9.*t11.*4.0;
et220 = Lx3.*Lxcm6.*dQ1.*dQ3.*m6.*t2.*t7.*t9.*t11.*-4.0-Lx3.*Lxcm6.*dQ1.*dQ2.*m6.*t3.*t8.*t9.*t11.*4.0-Lx3.*Lxcm6.*dQ1.*dQ3.*m6.*t3.*t8.*t9.*t11.*4.0-Lx3.*Lxcm6.*dQ2.*dQ3.*m6.*t4.*t7.*t8.*t11.*2.0+Lx3.*Lxcm5.*dQ4.*dQ5.*m5.*t4.*t7.*t8.*t10.*2.0-Lx3.*Lxcm6.*dQ1.*dQ6.*m6.*t2.*t7.*t10.*t11.*2.0-Lx3.*Lxcm6.*dQ1.*dQ6.*m6.*t3.*t8.*t10.*t11.*2.0+Lx3.*Lxcm6.*dQ4.*dQ6.*m6.*t6.*t7.*t8.*t9.*2.0+Lx2.*Lxcm6.*dQ5.*dQ6.*m6.*t2.*t9.*t10.*t11.*2.0-Lx3.*Lxcm4.*dQ1.*dQ2.*m4.*t2.*t4.*t7.*t33.*8.0-Lx3.*Lxcm4.*dQ1.*dQ2.*m4.*t3.*t4.*t8.*t32.*8.0-Lx3.*Lxcm4.*dQ1.*dQ3.*m4.*t2.*t4.*t7.*t33.*8.0-Lx3.*Lxcm4.*dQ1.*dQ3.*m4.*t3.*t4.*t8.*t32.*8.0-Lx2.*Lxcm5.*dQ1.*dQ2.*m5.*t4.*t5.*t8.*t32.*4.0-Lx2.*Lxcm5.*dQ1.*dQ3.*m5.*t4.*t5.*t8.*t32.*2.0-Lx2.*Lxcm5.*dQ1.*dQ4.*m5.*t3.*t5.*t9.*t32.*2.0;
et221 = Lx3.*Lxcm5.*dQ1.*dQ5.*m5.*t2.*t5.*t7.*t33.*-4.0-Lx2.*Lxcm5.*dQ1.*dQ5.*m5.*t3.*t4.*t10.*t32.*2.0-Lx3.*Lxcm5.*dQ1.*dQ5.*m5.*t3.*t5.*t8.*t32.*4.0-Lx2.*Lxcm6.*dQ1.*dQ2.*m6.*t3.*t6.*t10.*t32.*4.0-Lx2.*Lxcm6.*dQ1.*dQ3.*m6.*t3.*t6.*t10.*t32.*2.0-Lx2.*Lxcm6.*dQ1.*dQ4.*m6.*t3.*t4.*t11.*t32.*2.0-Lx2.*Lxcm6.*dQ1.*dQ5.*m6.*t5.*t6.*t8.*t32.*2.0-Lx2.*Lxcm6.*dQ1.*dQ6.*m6.*t3.*t6.*t9.*t32.*2.0+Lx3.*Lxcm6.*dQ1.*dQ4.*m6.*t5.*t6.*t9.*t32.*2.0+Lx3.*Lxcm6.*dQ1.*dQ4.*m6.*t5.*t6.*t9.*t33.*2.0+Lx3.*Lxcm6.*dQ1.*dQ5.*m6.*t4.*t6.*t10.*t32.*2.0+Lx3.*Lxcm6.*dQ1.*dQ5.*m6.*t4.*t6.*t10.*t33.*2.0+Lx3.*Lxcm6.*dQ1.*dQ6.*m6.*t4.*t5.*t11.*t32.*2.0+Lx3.*Lxcm6.*dQ1.*dQ6.*m6.*t4.*t5.*t11.*t33.*2.0+Lx2.*Lxcm6.*dQ1.*dQ2.*m6.*t8.*t9.*t11.*t32.*4.0+Lx2.*Lxcm6.*dQ1.*dQ3.*m6.*t8.*t9.*t11.*t32.*2.0+Lx2.*Lxcm6.*dQ1.*dQ6.*m6.*t8.*t10.*t11.*t32.*2.0;
et222 = Lx3.*Lxcm5.*dQ1.*dQ4.*m5.*t5.*t9.*t32.*t33.*-4.0-Lx3.*Lxcm5.*dQ1.*dQ5.*m5.*t4.*t10.*t32.*t33.*4.0-Lx3.*Lxcm6.*dQ1.*dQ2.*m6.*t6.*t10.*t32.*t33.*8.0-Lx3.*Lxcm6.*dQ1.*dQ3.*m6.*t6.*t10.*t32.*t33.*8.0-Lx3.*Lxcm6.*dQ1.*dQ4.*m6.*t4.*t11.*t32.*t33.*4.0-Lx3.*Lxcm6.*dQ1.*dQ6.*m6.*t6.*t9.*t32.*t33.*4.0+Lx2.*Lycm4.*dQ1.*dQ2.*m4.*t2.*t3.*t7.*t9.*4.0+Lx2.*Lycm4.*dQ1.*dQ3.*m4.*t2.*t3.*t7.*t9.*2.0+Lx3.*Lycm6.*dQ2.*dQ3.*m6.*t2.*t3.*t4.*t6.*2.0+Lx2.*Lycm4.*dQ1.*dQ4.*m4.*t2.*t4.*t7.*t8.*2.0+Lx2.*Lycm5.*dQ1.*dQ2.*m5.*t2.*t3.*t7.*t9.*4.0+Lx2.*Lycm5.*dQ1.*dQ3.*m5.*t2.*t3.*t7.*t9.*2.0+Lx2.*Lycm5.*dQ1.*dQ4.*m5.*t2.*t4.*t7.*t8.*2.0-Lx2.*Lycm6.*dQ4.*dQ6.*m6.*t2.*t4.*t5.*t6.*2.0-Lx3.*Lycm6.*dQ1.*dQ2.*m6.*t2.*t6.*t7.*t9.*4.0-Lx3.*Lycm6.*dQ1.*dQ3.*m6.*t2.*t6.*t7.*t9.*4.0-Lx3.*Lycm6.*dQ1.*dQ2.*m6.*t3.*t6.*t8.*t9.*4.0;
et223 = Lx2.*Lycm6.*dQ1.*dQ2.*m6.*t4.*t5.*t8.*t11.*-2.0-Lx3.*Lycm6.*dQ1.*dQ3.*m6.*t3.*t6.*t8.*t9.*4.0-Lx3.*Lycm6.*dQ2.*dQ3.*m6.*t4.*t6.*t7.*t8.*2.0-Lx3.*Lycm6.*dQ1.*dQ5.*m6.*t2.*t5.*t7.*t11.*2.0-Lx3.*Lycm6.*dQ1.*dQ6.*m6.*t2.*t6.*t7.*t10.*2.0-Lx3.*Lycm6.*dQ1.*dQ5.*m6.*t3.*t5.*t8.*t11.*2.0-Lx3.*Lycm6.*dQ1.*dQ6.*m6.*t3.*t6.*t8.*t10.*2.0+Lx2.*Lycm6.*dQ4.*dQ5.*m6.*t2.*t4.*t10.*t11.*2.0+Lx3.*Lycm6.*dQ4.*dQ6.*m6.*t2.*t3.*t9.*t11.*2.0+Lx2.*Lycm6.*dQ5.*dQ6.*m6.*t2.*t6.*t9.*t10.*2.0-Lx3.*Lycm6.*dQ4.*dQ6.*m6.*t7.*t8.*t9.*t11.*2.0-Lx2.*Lycm6.*dQ1.*dQ4.*m6.*t3.*t4.*t6.*t32.*2.0+Lx3.*Lycm4.*dQ1.*dQ2.*m4.*t2.*t7.*t9.*t33.*8.0+Lx3.*Lycm4.*dQ1.*dQ2.*m4.*t3.*t8.*t9.*t32.*8.0+Lx3.*Lycm4.*dQ1.*dQ3.*m4.*t2.*t7.*t9.*t33.*8.0+Lx3.*Lycm4.*dQ1.*dQ3.*m4.*t3.*t8.*t9.*t32.*8.0;
et224 = Lx3.*Lycm5.*dQ1.*dQ2.*m5.*t2.*t7.*t9.*t33.*8.0+Lx3.*Lycm5.*dQ1.*dQ2.*m5.*t3.*t8.*t9.*t32.*8.0+Lx3.*Lycm5.*dQ1.*dQ3.*m5.*t2.*t7.*t9.*t33.*8.0+Lx3.*Lycm5.*dQ1.*dQ3.*m5.*t3.*t8.*t9.*t32.*8.0+Lx3.*Lycm6.*dQ1.*dQ6.*m6.*t4.*t5.*t6.*t32.*2.0+Lx3.*Lycm6.*dQ1.*dQ6.*m6.*t4.*t5.*t6.*t33.*2.0+Lx2.*Lycm6.*dQ1.*dQ2.*m6.*t6.*t8.*t9.*t32.*4.0+Lx2.*Lycm6.*dQ1.*dQ2.*m6.*t3.*t10.*t11.*t32.*4.0+Lx2.*Lycm6.*dQ1.*dQ3.*m6.*t6.*t8.*t9.*t32.*2.0+Lx2.*Lycm6.*dQ1.*dQ3.*m6.*t3.*t10.*t11.*t32.*2.0+Lx2.*Lycm6.*dQ1.*dQ5.*m6.*t5.*t8.*t11.*t32.*2.0+Lx2.*Lycm6.*dQ1.*dQ6.*m6.*t3.*t9.*t11.*t32.*2.0+Lx2.*Lycm6.*dQ1.*dQ6.*m6.*t6.*t8.*t10.*t32.*2.0-Lx3.*Lycm6.*dQ1.*dQ4.*m6.*t5.*t9.*t11.*t32.*2.0-Lx3.*Lycm6.*dQ1.*dQ4.*m6.*t5.*t9.*t11.*t33.*2.0-Lx3.*Lycm6.*dQ1.*dQ5.*m6.*t4.*t10.*t11.*t32.*2.0-Lx3.*Lycm6.*dQ1.*dQ5.*m6.*t4.*t10.*t11.*t33.*2.0;
et225 = Lx3.*Lycm6.*dQ1.*dQ4.*m6.*t4.*t6.*t32.*t33.*-4.0+Lx3.*Lycm6.*dQ1.*dQ2.*m6.*t10.*t11.*t32.*t33.*8.0+Lx3.*Lycm6.*dQ1.*dQ3.*m6.*t10.*t11.*t32.*t33.*8.0+Lx3.*Lycm6.*dQ1.*dQ6.*m6.*t9.*t11.*t32.*t33.*4.0+Lxcm5.*Lycm5.*dQ2.*dQ5.*m5.*t2.*t3.*t4.*t5.*2.0-Lxcm4.*Lycm4.*dQ1.*dQ2.*m4.*t2.*t4.*t7.*t9.*4.0-Lxcm4.*Lycm4.*dQ1.*dQ4.*m4.*t2.*t3.*t7.*t8.*4.0+Lxcm5.*Lycm5.*dQ3.*dQ5.*m5.*t2.*t3.*t4.*t5.*2.0-Lxcm4.*Lycm4.*dQ1.*dQ3.*m4.*t2.*t4.*t7.*t9.*4.0-Lxcm4.*Lycm4.*dQ1.*dQ2.*m4.*t3.*t4.*t8.*t9.*4.0-Lxcm6.*Lycm6.*dQ2.*dQ5.*m6.*t2.*t3.*t4.*t5.*2.0-Lxcm4.*Lycm4.*dQ1.*dQ3.*m4.*t3.*t4.*t8.*t9.*4.0-Lxcm6.*Lycm6.*dQ3.*dQ5.*m6.*t2.*t3.*t4.*t5.*2.0-Lxcm4.*Lycm4.*dQ2.*dQ4.*m4.*t2.*t4.*t8.*t9.*4.0-Lxcm4.*Lycm4.*dQ2.*dQ4.*m4.*t3.*t4.*t7.*t9.*4.0-Lxcm4.*Lycm4.*dQ3.*dQ4.*m4.*t2.*t4.*t8.*t9.*4.0;
et226 = Lxcm4.*Lycm4.*dQ3.*dQ4.*m4.*t3.*t4.*t7.*t9.*-4.0-Lxcm5.*Lycm5.*dQ1.*dQ4.*m5.*t2.*t4.*t7.*t10.*2.0-Lxcm5.*Lycm5.*dQ1.*dQ5.*m5.*t2.*t5.*t7.*t9.*2.0-Lxcm5.*Lycm5.*dQ2.*dQ3.*m5.*t2.*t4.*t8.*t10.*2.0-Lxcm5.*Lycm5.*dQ2.*dQ3.*m5.*t3.*t4.*t7.*t10.*2.0-Lxcm5.*Lycm5.*dQ1.*dQ4.*m5.*t3.*t4.*t8.*t10.*2.0+Lxcm6.*Lycm6.*dQ1.*dQ6.*m6.*t2.*t3.*t7.*t8.*8.0-Lxcm5.*Lycm5.*dQ1.*dQ5.*m5.*t3.*t5.*t8.*t9.*2.0-Lxcm5.*Lycm5.*dQ2.*dQ5.*m5.*t4.*t5.*t7.*t8.*2.0+Lxcm6.*Lycm6.*dQ1.*dQ4.*m6.*t2.*t4.*t7.*t10.*2.0-Lxcm5.*Lycm5.*dQ3.*dQ5.*m5.*t4.*t5.*t7.*t8.*2.0+Lxcm6.*Lycm6.*dQ1.*dQ2.*m6.*t2.*t6.*t7.*t11.*8.0+Lxcm6.*Lycm6.*dQ1.*dQ5.*m6.*t2.*t5.*t7.*t9.*2.0+Lxcm6.*Lycm6.*dQ2.*dQ3.*m6.*t2.*t4.*t8.*t10.*2.0+Lxcm6.*Lycm6.*dQ2.*dQ3.*m6.*t3.*t4.*t7.*t10.*2.0+Lxcm6.*Lycm6.*dQ1.*dQ3.*m6.*t2.*t6.*t7.*t11.*8.0+Lxcm6.*Lycm6.*dQ1.*dQ4.*m6.*t3.*t4.*t8.*t10.*2.0;
et227 = Lxcm6.*Lycm6.*dQ1.*dQ2.*m6.*t3.*t6.*t8.*t11.*8.0+Lxcm6.*Lycm6.*dQ1.*dQ5.*m6.*t3.*t5.*t8.*t9.*2.0+Lxcm6.*Lycm6.*dQ2.*dQ5.*m6.*t4.*t5.*t7.*t8.*2.0+Lxcm6.*Lycm6.*dQ2.*dQ6.*m6.*t2.*t4.*t8.*t9.*2.0+Lxcm6.*Lycm6.*dQ2.*dQ6.*m6.*t3.*t4.*t7.*t9.*2.0+Lxcm6.*Lycm6.*dQ1.*dQ3.*m6.*t3.*t6.*t8.*t11.*8.0+Lxcm6.*Lycm6.*dQ3.*dQ5.*m6.*t4.*t5.*t7.*t8.*2.0+Lxcm6.*Lycm6.*dQ3.*dQ6.*m6.*t2.*t4.*t8.*t9.*2.0+Lxcm6.*Lycm6.*dQ3.*dQ6.*m6.*t3.*t4.*t7.*t9.*2.0+Lxcm6.*Lycm6.*dQ1.*dQ5.*m6.*t5.*t6.*t10.*t11.*4.0+Lxcm5.*Lycm5.*dQ2.*dQ3.*m5.*t2.*t3.*t5.*t34.*4.0-Lxcm6.*Lycm6.*dQ2.*dQ3.*m6.*t2.*t3.*t5.*t34.*4.0-Lxcm6.*Lycm6.*dQ2.*dQ3.*m6.*t2.*t3.*t5.*t36.*4.0-Lxcm5.*Lycm5.*dQ2.*dQ3.*m5.*t5.*t7.*t8.*t34.*4.0-Lxcm5.*Lycm5.*dQ1.*dQ5.*m5.*t4.*t9.*t10.*t32.*2.0-Lxcm5.*Lycm5.*dQ2.*dQ5.*m5.*t2.*t8.*t10.*t34.*2.0-Lxcm5.*Lycm5.*dQ2.*dQ5.*m5.*t3.*t7.*t10.*t34.*2.0;
et228 = Lxcm5.*Lycm5.*dQ1.*dQ5.*m5.*t4.*t9.*t10.*t33.*-2.0-Lxcm5.*Lycm5.*dQ3.*dQ5.*m5.*t2.*t8.*t10.*t34.*2.0-Lxcm5.*Lycm5.*dQ3.*dQ5.*m5.*t3.*t7.*t10.*t34.*2.0+Lxcm6.*Lycm6.*dQ2.*dQ3.*m6.*t5.*t7.*t8.*t34.*4.0+Lxcm6.*Lycm6.*dQ1.*dQ5.*m6.*t4.*t9.*t10.*t32.*2.0+Lxcm6.*Lycm6.*dQ2.*dQ3.*m6.*t5.*t7.*t8.*t36.*4.0+Lxcm6.*Lycm6.*dQ2.*dQ5.*m6.*t2.*t8.*t10.*t34.*2.0+Lxcm6.*Lycm6.*dQ2.*dQ5.*m6.*t3.*t7.*t10.*t34.*2.0+Lxcm6.*Lycm6.*dQ1.*dQ5.*m6.*t4.*t9.*t10.*t33.*2.0+Lxcm6.*Lycm6.*dQ3.*dQ5.*m6.*t2.*t8.*t10.*t34.*2.0+Lxcm6.*Lycm6.*dQ3.*dQ5.*m6.*t3.*t7.*t10.*t34.*2.0-Lxcm6.*Lycm6.*dQ5.*dQ6.*m6.*t2.*t8.*t9.*t36.*4.0-Lxcm6.*Lycm6.*dQ5.*dQ6.*m6.*t3.*t7.*t9.*t36.*4.0+Lxcm5.*Lycm5.*dQ1.*dQ2.*m5.*t9.*t10.*t32.*t33.*8.0+Lxcm5.*Lycm5.*dQ1.*dQ3.*m5.*t9.*t10.*t32.*t33.*8.0-Lxcm6.*Lycm6.*dQ4.*dQ6.*m6.*t2.*t3.*t35.*t36.*4.0-Lxcm6.*Lycm6.*dQ1.*dQ2.*m6.*t9.*t10.*t32.*t33.*8.0;
et229 = Lxcm6.*Lycm6.*dQ1.*dQ3.*m6.*t9.*t10.*t32.*t33.*-8.0-Lxcm6.*Lycm6.*dQ1.*dQ2.*m6.*t9.*t10.*t32.*t36.*8.0-Lxcm6.*Lycm6.*dQ1.*dQ2.*m6.*t9.*t10.*t33.*t36.*8.0-Lxcm6.*Lycm6.*dQ1.*dQ3.*m6.*t9.*t10.*t32.*t36.*8.0-Lxcm6.*Lycm6.*dQ1.*dQ3.*m6.*t9.*t10.*t33.*t36.*8.0+Lxcm6.*Lycm6.*dQ4.*dQ6.*m6.*t7.*t8.*t35.*t36.*4.0-Lxcm5.*Lycm5.*dQ1.*dQ4.*m5.*t5.*t32.*t33.*t34.*8.0+Lxcm6.*Lycm6.*dQ1.*dQ4.*m6.*t5.*t32.*t33.*t34.*8.0+Lxcm6.*Lycm6.*dQ1.*dQ4.*m6.*t5.*t32.*t33.*t36.*8.0+Lxcm6.*Lycm6.*dQ1.*dQ4.*m6.*t5.*t32.*t34.*t36.*8.0+Lxcm6.*Lycm6.*dQ1.*dQ4.*m6.*t5.*t33.*t34.*t36.*8.0+Lxcm6.*Lycm6.*dQ1.*dQ6.*m6.*t32.*t33.*t34.*t35.*4.0-Lxcm6.*Lycm6.*dQ1.*dQ6.*m6.*t32.*t33.*t34.*t36.*8.0-Lxcm6.*Lycm6.*dQ1.*dQ6.*m6.*t32.*t33.*t35.*t36.*8.0+Lxcm6.*Lycm6.*dQ1.*dQ6.*m6.*t32.*t34.*t35.*t36.*4.0+Lxcm6.*Lycm6.*dQ1.*dQ6.*m6.*t33.*t34.*t35.*t36.*4.0;
et230 = Lx3.*Lz4.*dQ1.*dQ2.*m5.*t2.*t3.*t7.*t8.*-8.0-Lx3.*Lz4.*dQ1.*dQ2.*m6.*t2.*t3.*t7.*t8.*8.0-Lx3.*Lz4.*dQ1.*dQ3.*m5.*t2.*t3.*t7.*t8.*8.0-Lx3.*Lz4.*dQ1.*dQ3.*m6.*t2.*t3.*t7.*t8.*8.0+Lx3.*Lz5.*dQ4.*dQ5.*m6.*t2.*t3.*t4.*t5.*2.0-Lx2.*Lz5.*dQ1.*dQ2.*m6.*t2.*t5.*t7.*t8.*4.0-Lx2.*Lz5.*dQ1.*dQ3.*m6.*t2.*t5.*t7.*t8.*2.0+Lx3.*Lz5.*dQ1.*dQ2.*m6.*t2.*t4.*t7.*t10.*4.0-Lx2.*Lz5.*dQ1.*dQ5.*m6.*t2.*t3.*t7.*t10.*2.0+Lx3.*Lz5.*dQ1.*dQ3.*m6.*t2.*t4.*t7.*t10.*4.0+Lx3.*Lz5.*dQ1.*dQ2.*m6.*t3.*t4.*t8.*t10.*4.0+Lx3.*Lz5.*dQ1.*dQ3.*m6.*t3.*t4.*t8.*t10.*4.0+Lx3.*Lz5.*dQ2.*dQ3.*m6.*t2.*t3.*t9.*t10.*2.0-Lx3.*Lz5.*dQ4.*dQ5.*m6.*t4.*t5.*t7.*t8.*2.0-Lx3.*Lz5.*dQ2.*dQ3.*m6.*t7.*t8.*t9.*t10.*2.0+Lx2.*Lz5.*dQ1.*dQ5.*m6.*t3.*t4.*t5.*t32.*2.0;
et231 = Lx2.*Lz5.*dQ1.*dQ2.*m6.*t4.*t8.*t10.*t32.*-4.0-Lx2.*Lz5.*dQ1.*dQ3.*m6.*t4.*t8.*t10.*t32.*2.0-Lx2.*Lz5.*dQ1.*dQ4.*m6.*t3.*t9.*t10.*t32.*2.0-Lx3.*Lz5.*dQ1.*dQ5.*m6.*t2.*t7.*t10.*t33.*4.0-Lx3.*Lz5.*dQ1.*dQ5.*m6.*t3.*t8.*t10.*t32.*4.0+Lx3.*Lz5.*dQ1.*dQ5.*m6.*t4.*t5.*t32.*t33.*4.0-Lx3.*Lz5.*dQ1.*dQ4.*m6.*t9.*t10.*t32.*t33.*4.0-Lx3.*Lzcm4.*dQ1.*dQ2.*m4.*t2.*t3.*t7.*t8.*8.0-Lx3.*Lzcm4.*dQ1.*dQ3.*m4.*t2.*t3.*t7.*t8.*8.0+Lx3.*Lzcm5.*dQ4.*dQ5.*m5.*t2.*t3.*t4.*t5.*2.0-Lx2.*Lzcm5.*dQ1.*dQ2.*m5.*t2.*t5.*t7.*t8.*4.0-Lx2.*Lzcm5.*dQ1.*dQ3.*m5.*t2.*t5.*t7.*t8.*2.0+Lx3.*Lzcm6.*dQ4.*dQ5.*m6.*t2.*t3.*t4.*t5.*2.0-Lx2.*Lzcm6.*dQ1.*dQ2.*m6.*t2.*t5.*t7.*t8.*4.0+Lx3.*Lzcm5.*dQ1.*dQ2.*m5.*t2.*t4.*t7.*t10.*4.0-Lx2.*Lzcm5.*dQ1.*dQ5.*m5.*t2.*t3.*t7.*t10.*2.0;
et232 = Lx2.*Lzcm6.*dQ1.*dQ3.*m6.*t2.*t5.*t7.*t8.*-2.0+Lx3.*Lzcm5.*dQ1.*dQ3.*m5.*t2.*t4.*t7.*t10.*4.0+Lx3.*Lzcm5.*dQ1.*dQ2.*m5.*t3.*t4.*t8.*t10.*4.0+Lx3.*Lzcm6.*dQ1.*dQ2.*m6.*t2.*t4.*t7.*t10.*4.0-Lx2.*Lzcm6.*dQ1.*dQ5.*m6.*t2.*t3.*t7.*t10.*2.0+Lx3.*Lzcm5.*dQ1.*dQ3.*m5.*t3.*t4.*t8.*t10.*4.0+Lx3.*Lzcm5.*dQ2.*dQ3.*m5.*t2.*t3.*t9.*t10.*2.0+Lx3.*Lzcm6.*dQ1.*dQ3.*m6.*t2.*t4.*t7.*t10.*4.0+Lxcm5.*Lz4.*dQ1.*dQ4.*m5.*t2.*t5.*t7.*t9.*2.0+Lx3.*Lzcm6.*dQ1.*dQ2.*m6.*t3.*t4.*t8.*t10.*4.0+Lxcm5.*Lz4.*dQ1.*dQ5.*m5.*t2.*t4.*t7.*t10.*2.0+Lxcm5.*Lz4.*dQ2.*dQ3.*m5.*t2.*t5.*t8.*t9.*2.0+Lxcm5.*Lz4.*dQ2.*dQ3.*m5.*t3.*t5.*t7.*t9.*2.0+Lx3.*Lzcm6.*dQ1.*dQ3.*m6.*t3.*t4.*t8.*t10.*4.0+Lx3.*Lzcm6.*dQ2.*dQ3.*m6.*t2.*t3.*t9.*t10.*2.0+Lxcm5.*Lz4.*dQ1.*dQ4.*m5.*t3.*t5.*t8.*t9.*2.0+Lxcm6.*Lz4.*dQ1.*dQ2.*m6.*t2.*t6.*t7.*t10.*4.0+Lxcm5.*Lz4.*dQ1.*dQ5.*m5.*t3.*t4.*t8.*t10.*2.0;
et233 = Lxcm6.*Lz4.*dQ1.*dQ3.*m6.*t2.*t6.*t7.*t10.*4.0+Lxcm6.*Lz4.*dQ1.*dQ4.*m6.*t2.*t4.*t7.*t11.*2.0-Lx3.*Lzcm5.*dQ4.*dQ5.*m5.*t4.*t5.*t7.*t8.*2.0+Lxcm6.*Lz4.*dQ1.*dQ2.*m6.*t3.*t6.*t8.*t10.*4.0+Lxcm6.*Lz4.*dQ2.*dQ3.*m6.*t2.*t4.*t8.*t11.*2.0+Lxcm6.*Lz4.*dQ2.*dQ3.*m6.*t3.*t4.*t7.*t11.*2.0-Lxcm6.*Lz5.*dQ1.*dQ4.*m6.*t2.*t6.*t7.*t9.*2.0-Lxcm5.*Lz4.*dQ4.*dQ5.*m5.*t2.*t4.*t8.*t10.*2.0-Lxcm5.*Lz4.*dQ4.*dQ5.*m5.*t3.*t4.*t7.*t10.*2.0+Lxcm6.*Lz4.*dQ1.*dQ3.*m6.*t3.*t6.*t8.*t10.*4.0+Lxcm6.*Lz4.*dQ1.*dQ4.*m6.*t3.*t4.*t8.*t11.*2.0+Lxcm6.*Lz4.*dQ1.*dQ6.*m6.*t2.*t6.*t7.*t9.*2.0-Lxcm6.*Lz5.*dQ2.*dQ3.*m6.*t2.*t6.*t8.*t9.*2.0-Lxcm6.*Lz5.*dQ2.*dQ3.*m6.*t3.*t6.*t7.*t9.*2.0-Lx3.*Lzcm6.*dQ4.*dQ5.*m6.*t4.*t5.*t7.*t8.*2.0-Lxcm6.*Lz5.*dQ1.*dQ4.*m6.*t3.*t6.*t8.*t9.*2.0-Lxcm6.*Lz5.*dQ1.*dQ6.*m6.*t2.*t4.*t7.*t11.*2.0;
et234 = Lxcm6.*Lz5.*dQ2.*dQ3.*m6.*t2.*t3.*t10.*t11.*-2.0+Lxcm6.*Lz4.*dQ1.*dQ6.*m6.*t3.*t6.*t8.*t9.*2.0-Lxcm6.*Lz5.*dQ1.*dQ6.*m6.*t3.*t4.*t8.*t11.*2.0-Lxcm6.*Lz5.*dQ2.*dQ6.*m6.*t2.*t3.*t9.*t11.*2.0-Lxcm6.*Lz4.*dQ4.*dQ6.*m6.*t2.*t6.*t8.*t9.*2.0-Lxcm6.*Lz4.*dQ4.*dQ6.*m6.*t3.*t6.*t7.*t9.*2.0-Lxcm6.*Lz5.*dQ2.*dQ6.*m6.*t2.*t6.*t8.*t10.*2.0-Lxcm6.*Lz5.*dQ2.*dQ6.*m6.*t3.*t6.*t7.*t10.*2.0-Lxcm6.*Lz5.*dQ3.*dQ6.*m6.*t2.*t3.*t9.*t11.*2.0-Lx3.*Lzcm5.*dQ2.*dQ3.*m5.*t7.*t8.*t9.*t10.*2.0-Lxcm6.*Lz5.*dQ3.*dQ6.*m6.*t2.*t6.*t8.*t10.*2.0-Lxcm6.*Lz5.*dQ3.*dQ6.*m6.*t3.*t6.*t7.*t10.*2.0-Lx3.*Lzcm6.*dQ2.*dQ3.*m6.*t7.*t8.*t9.*t10.*2.0+Lxcm6.*Lz5.*dQ2.*dQ3.*m6.*t7.*t8.*t10.*t11.*2.0+Lxcm6.*Lz5.*dQ2.*dQ6.*m6.*t7.*t8.*t9.*t11.*2.0+Lxcm6.*Lz5.*dQ3.*dQ6.*m6.*t7.*t8.*t9.*t11.*2.0+Lx2.*Lzcm5.*dQ1.*dQ5.*m5.*t3.*t4.*t5.*t32.*2.0;
et235 = Lx2.*Lzcm6.*dQ1.*dQ5.*m6.*t3.*t4.*t5.*t32.*2.0-Lxcm6.*Lz4.*dQ1.*dQ2.*m6.*t4.*t5.*t6.*t32.*4.0-Lxcm6.*Lz4.*dQ1.*dQ2.*m6.*t4.*t5.*t6.*t33.*4.0-Lxcm6.*Lz4.*dQ1.*dQ3.*m6.*t4.*t5.*t6.*t32.*4.0-Lxcm6.*Lz4.*dQ1.*dQ3.*m6.*t4.*t5.*t6.*t33.*4.0-Lx2.*Lzcm5.*dQ1.*dQ2.*m5.*t4.*t8.*t10.*t32.*4.0-Lxcm5.*Lz4.*dQ1.*dQ2.*m5.*t2.*t7.*t10.*t33.*8.0-Lx2.*Lzcm5.*dQ1.*dQ3.*m5.*t4.*t8.*t10.*t32.*2.0-Lxcm5.*Lz4.*dQ1.*dQ2.*m5.*t3.*t8.*t10.*t32.*8.0-Lxcm5.*Lz4.*dQ1.*dQ3.*m5.*t2.*t7.*t10.*t33.*8.0-Lx2.*Lzcm5.*dQ1.*dQ4.*m5.*t3.*t9.*t10.*t32.*2.0-Lx2.*Lzcm6.*dQ1.*dQ2.*m6.*t4.*t8.*t10.*t32.*4.0-Lx3.*Lzcm5.*dQ1.*dQ5.*m5.*t2.*t7.*t10.*t33.*4.0-Lxcm5.*Lz4.*dQ1.*dQ3.*m5.*t3.*t8.*t10.*t32.*8.0-Lx2.*Lzcm6.*dQ1.*dQ3.*m6.*t4.*t8.*t10.*t32.*2.0-Lx3.*Lzcm5.*dQ1.*dQ5.*m5.*t3.*t8.*t10.*t32.*4.0;
et236 = Lxcm6.*Lz5.*dQ4.*dQ5.*m6.*t2.*t3.*t6.*t35.*4.0-Lx2.*Lzcm6.*dQ1.*dQ4.*m6.*t3.*t9.*t10.*t32.*2.0-Lx3.*Lzcm6.*dQ1.*dQ5.*m6.*t2.*t7.*t10.*t33.*4.0-Lx3.*Lzcm6.*dQ1.*dQ5.*m6.*t3.*t8.*t10.*t32.*4.0+Lxcm6.*Lz5.*dQ1.*dQ2.*m6.*t5.*t9.*t11.*t32.*4.0+Lxcm6.*Lz5.*dQ1.*dQ2.*m6.*t5.*t9.*t11.*t33.*4.0+Lxcm6.*Lz5.*dQ1.*dQ3.*m6.*t5.*t9.*t11.*t32.*4.0+Lxcm6.*Lz5.*dQ1.*dQ3.*m6.*t5.*t9.*t11.*t33.*4.0+Lxcm6.*Lz5.*dQ1.*dQ6.*m6.*t5.*t10.*t11.*t32.*2.0-Lxcm6.*Lz5.*dQ4.*dQ5.*m6.*t6.*t7.*t8.*t35.*4.0+Lxcm6.*Lz5.*dQ1.*dQ6.*m6.*t5.*t10.*t11.*t33.*2.0+Lxcm5.*Lz4.*dQ1.*dQ2.*m5.*t4.*t5.*t32.*t33.*8.0+Lxcm5.*Lz4.*dQ1.*dQ3.*m5.*t4.*t5.*t32.*t33.*8.0+Lx3.*Lzcm5.*dQ1.*dQ5.*m5.*t4.*t5.*t32.*t33.*4.0+Lx3.*Lzcm6.*dQ1.*dQ5.*m6.*t4.*t5.*t32.*t33.*4.0-Lxcm6.*Lz5.*dQ1.*dQ2.*m6.*t4.*t6.*t32.*t33.*8.0-Lxcm6.*Lz5.*dQ1.*dQ3.*m6.*t4.*t6.*t32.*t33.*8.0;
et237 = Lxcm6.*Lz5.*dQ1.*dQ2.*m6.*t4.*t6.*t32.*t35.*-8.0+Lxcm6.*Lz4.*dQ1.*dQ5.*m6.*t5.*t6.*t32.*t33.*4.0-Lxcm6.*Lz5.*dQ1.*dQ2.*m6.*t4.*t6.*t33.*t35.*8.0-Lxcm6.*Lz5.*dQ1.*dQ3.*m6.*t4.*t6.*t32.*t35.*8.0-Lxcm6.*Lz5.*dQ1.*dQ3.*m6.*t4.*t6.*t33.*t35.*8.0-Lx3.*Lzcm5.*dQ1.*dQ4.*m5.*t9.*t10.*t32.*t33.*4.0-Lx3.*Lzcm6.*dQ1.*dQ4.*m6.*t9.*t10.*t32.*t33.*4.0-Lxcm6.*Lz4.*dQ1.*dQ2.*m6.*t9.*t11.*t32.*t33.*8.0-Lxcm6.*Lz4.*dQ1.*dQ3.*m6.*t9.*t11.*t32.*t33.*8.0+Lxcm6.*Lz5.*dQ1.*dQ4.*m6.*t10.*t11.*t32.*t33.*4.0-Lxcm6.*Lz4.*dQ1.*dQ6.*m6.*t10.*t11.*t32.*t33.*4.0+Lxcm6.*Lz5.*dQ1.*dQ4.*m6.*t10.*t11.*t32.*t34.*4.0+Lxcm6.*Lz5.*dQ1.*dQ4.*m6.*t10.*t11.*t33.*t34.*4.0-Lxcm6.*Lz5.*dQ1.*dQ5.*m6.*t6.*t32.*t33.*t34.*4.0+Lxcm6.*Lz5.*dQ1.*dQ5.*m6.*t6.*t32.*t33.*t35.*8.0-Lxcm6.*Lz5.*dQ1.*dQ5.*m6.*t6.*t32.*t34.*t35.*4.0;
et238 = Lxcm6.*Lz5.*dQ1.*dQ5.*m6.*t6.*t33.*t34.*t35.*-4.0-Lxcm3.*Lzcm3.*dQ1.*dQ2.*m3.*t2.*t3.*t7.*t8.*8.0-Lxcm3.*Lzcm3.*dQ1.*dQ3.*m3.*t2.*t3.*t7.*t8.*8.0+Lxcm5.*Lzcm5.*dQ1.*dQ5.*m5.*t2.*t3.*t7.*t8.*4.0+Lxcm5.*Lzcm5.*dQ1.*dQ2.*m5.*t2.*t5.*t7.*t10.*4.0+Lxcm5.*Lzcm5.*dQ1.*dQ3.*m5.*t2.*t5.*t7.*t10.*4.0+Lxcm5.*Lzcm5.*dQ1.*dQ2.*m5.*t3.*t5.*t8.*t10.*4.0+Lxcm5.*Lzcm5.*dQ1.*dQ3.*m5.*t3.*t5.*t8.*t10.*4.0-Lxcm5.*Lzcm5.*dQ2.*dQ5.*m5.*t2.*t4.*t8.*t9.*2.0-Lxcm5.*Lzcm5.*dQ2.*dQ5.*m5.*t3.*t4.*t7.*t9.*2.0-Lxcm5.*Lzcm5.*dQ2.*dQ4.*m5.*t2.*t5.*t8.*t10.*4.0-Lxcm5.*Lzcm5.*dQ2.*dQ4.*m5.*t3.*t5.*t7.*t10.*4.0-Lxcm5.*Lzcm5.*dQ3.*dQ5.*m5.*t2.*t4.*t8.*t9.*2.0-Lxcm5.*Lzcm5.*dQ3.*dQ5.*m5.*t3.*t4.*t7.*t9.*2.0-Lxcm5.*Lzcm5.*dQ3.*dQ4.*m5.*t2.*t5.*t8.*t10.*4.0-Lxcm5.*Lzcm5.*dQ3.*dQ4.*m5.*t3.*t5.*t7.*t10.*4.0;
et239 = Lxcm6.*Lzcm6.*dQ1.*dQ4.*m6.*t2.*t6.*t7.*t9.*-2.0-Lxcm6.*Lzcm6.*dQ2.*dQ3.*m6.*t2.*t6.*t8.*t9.*2.0-Lxcm6.*Lzcm6.*dQ2.*dQ3.*m6.*t3.*t6.*t7.*t9.*2.0-Lxcm6.*Lzcm6.*dQ1.*dQ4.*m6.*t3.*t6.*t8.*t9.*2.0-Lxcm6.*Lzcm6.*dQ1.*dQ6.*m6.*t2.*t4.*t7.*t11.*2.0-Lxcm6.*Lzcm6.*dQ2.*dQ3.*m6.*t2.*t3.*t10.*t11.*2.0-Lxcm6.*Lzcm6.*dQ1.*dQ6.*m6.*t3.*t4.*t8.*t11.*2.0-Lxcm6.*Lzcm6.*dQ2.*dQ6.*m6.*t2.*t3.*t9.*t11.*2.0-Lxcm6.*Lzcm6.*dQ2.*dQ6.*m6.*t2.*t6.*t8.*t10.*2.0-Lxcm6.*Lzcm6.*dQ2.*dQ6.*m6.*t3.*t6.*t7.*t10.*2.0-Lxcm6.*Lzcm6.*dQ3.*dQ6.*m6.*t2.*t3.*t9.*t11.*2.0-Lxcm6.*Lzcm6.*dQ3.*dQ6.*m6.*t2.*t6.*t8.*t10.*2.0-Lxcm6.*Lzcm6.*dQ3.*dQ6.*m6.*t3.*t6.*t7.*t10.*2.0+Lxcm6.*Lzcm6.*dQ2.*dQ3.*m6.*t7.*t8.*t10.*t11.*2.0+Lxcm6.*Lzcm6.*dQ2.*dQ6.*m6.*t7.*t8.*t9.*t11.*2.0+Lxcm6.*Lzcm6.*dQ3.*dQ6.*m6.*t7.*t8.*t9.*t11.*2.0;
et240 = Lxcm4.*Lzcm4.*dQ1.*dQ4.*m4.*t2.*t7.*t9.*t33.*-4.0-Lxcm4.*Lzcm4.*dQ1.*dQ4.*m4.*t3.*t8.*t9.*t32.*4.0+Lxcm5.*Lzcm5.*dQ1.*dQ4.*m5.*t2.*t7.*t9.*t33.*4.0+Lxcm5.*Lzcm5.*dQ1.*dQ4.*m5.*t3.*t8.*t9.*t32.*4.0+Lxcm5.*Lzcm5.*dQ1.*dQ4.*m5.*t2.*t7.*t9.*t35.*4.0+Lxcm6.*Lzcm6.*dQ4.*dQ5.*m6.*t2.*t3.*t6.*t35.*4.0+Lxcm5.*Lzcm5.*dQ2.*dQ3.*m5.*t2.*t8.*t9.*t35.*4.0+Lxcm5.*Lzcm5.*dQ2.*dQ3.*m5.*t3.*t7.*t9.*t35.*4.0+Lxcm5.*Lzcm5.*dQ1.*dQ4.*m5.*t3.*t8.*t9.*t35.*4.0+Lxcm6.*Lzcm6.*dQ1.*dQ2.*m6.*t5.*t9.*t11.*t32.*4.0+Lxcm6.*Lzcm6.*dQ1.*dQ2.*m6.*t5.*t9.*t11.*t33.*4.0+Lxcm6.*Lzcm6.*dQ1.*dQ3.*m6.*t5.*t9.*t11.*t32.*4.0+Lxcm6.*Lzcm6.*dQ1.*dQ3.*m6.*t5.*t9.*t11.*t33.*4.0+Lxcm6.*Lzcm6.*dQ1.*dQ6.*m6.*t5.*t10.*t11.*t32.*2.0-Lxcm6.*Lzcm6.*dQ4.*dQ5.*m6.*t6.*t7.*t8.*t35.*4.0+Lxcm6.*Lzcm6.*dQ1.*dQ6.*m6.*t5.*t10.*t11.*t33.*2.0-Lxcm6.*Lzcm6.*dQ1.*dQ2.*m6.*t4.*t6.*t32.*t33.*8.0;
et241 = Lxcm6.*Lzcm6.*dQ1.*dQ3.*m6.*t4.*t6.*t32.*t33.*-8.0-Lxcm6.*Lzcm6.*dQ1.*dQ2.*m6.*t4.*t6.*t32.*t35.*8.0-Lxcm6.*Lzcm6.*dQ1.*dQ2.*m6.*t4.*t6.*t33.*t35.*8.0-Lxcm6.*Lzcm6.*dQ1.*dQ3.*m6.*t4.*t6.*t32.*t35.*8.0-Lxcm6.*Lzcm6.*dQ1.*dQ3.*m6.*t4.*t6.*t33.*t35.*8.0+Lxcm6.*Lzcm6.*dQ1.*dQ4.*m6.*t10.*t11.*t32.*t33.*4.0+Lxcm6.*Lzcm6.*dQ1.*dQ4.*m6.*t10.*t11.*t32.*t34.*4.0+Lxcm6.*Lzcm6.*dQ1.*dQ4.*m6.*t10.*t11.*t33.*t34.*4.0+Lxcm5.*Lzcm5.*dQ1.*dQ2.*m5.*t4.*t32.*t33.*t35.*1.6e+1+Lxcm5.*Lzcm5.*dQ1.*dQ3.*m5.*t4.*t32.*t33.*t35.*1.6e+1-Lxcm6.*Lzcm6.*dQ1.*dQ5.*m6.*t6.*t32.*t33.*t34.*4.0+Lxcm6.*Lzcm6.*dQ1.*dQ5.*m6.*t6.*t32.*t33.*t35.*8.0-Lxcm6.*Lzcm6.*dQ1.*dQ5.*m6.*t6.*t32.*t34.*t35.*4.0-Lxcm6.*Lzcm6.*dQ1.*dQ5.*m6.*t6.*t33.*t34.*t35.*4.0+Lxcm5.*Lzcm5.*dQ1.*dQ5.*m5.*t32.*t33.*t34.*t35.*8.0+Lycm6.*Lz4.*dQ1.*dQ4.*m6.*t2.*t4.*t6.*t7.*2.0;
et242 = Lycm6.*Lz4.*dQ2.*dQ3.*m6.*t2.*t4.*t6.*t8.*2.0+Lycm6.*Lz4.*dQ2.*dQ3.*m6.*t3.*t4.*t6.*t7.*2.0+Lycm6.*Lz4.*dQ1.*dQ4.*m6.*t3.*t4.*t6.*t8.*2.0-Lycm6.*Lz5.*dQ1.*dQ6.*m6.*t2.*t4.*t6.*t7.*2.0-Lycm6.*Lz5.*dQ2.*dQ3.*m6.*t2.*t3.*t6.*t10.*2.0-Lycm6.*Lz5.*dQ1.*dQ6.*m6.*t3.*t4.*t6.*t8.*2.0-Lycm6.*Lz5.*dQ2.*dQ6.*m6.*t2.*t3.*t6.*t9.*2.0-Lycm6.*Lz5.*dQ3.*dQ6.*m6.*t2.*t3.*t6.*t9.*2.0-Lycm6.*Lz4.*dQ1.*dQ2.*m6.*t2.*t7.*t10.*t11.*4.0-Lycm6.*Lz4.*dQ1.*dQ3.*m6.*t2.*t7.*t10.*t11.*4.0-Lycm6.*Lz4.*dQ1.*dQ2.*m6.*t3.*t8.*t10.*t11.*4.0+Lycm6.*Lz5.*dQ1.*dQ4.*m6.*t2.*t7.*t9.*t11.*2.0-Lycm6.*Lz4.*dQ1.*dQ3.*m6.*t3.*t8.*t10.*t11.*4.0-Lycm6.*Lz4.*dQ1.*dQ6.*m6.*t2.*t7.*t9.*t11.*2.0+Lycm6.*Lz5.*dQ2.*dQ3.*m6.*t2.*t8.*t9.*t11.*2.0+Lycm6.*Lz5.*dQ2.*dQ3.*m6.*t3.*t7.*t9.*t11.*2.0+Lycm6.*Lz5.*dQ1.*dQ4.*m6.*t3.*t8.*t9.*t11.*2.0;
et243 = Lycm6.*Lz5.*dQ2.*dQ3.*m6.*t6.*t7.*t8.*t10.*2.0-Lycm6.*Lz4.*dQ1.*dQ6.*m6.*t3.*t8.*t9.*t11.*2.0+Lycm6.*Lz5.*dQ2.*dQ6.*m6.*t6.*t7.*t8.*t9.*2.0+Lycm6.*Lz4.*dQ4.*dQ6.*m6.*t2.*t8.*t9.*t11.*2.0+Lycm6.*Lz4.*dQ4.*dQ6.*m6.*t3.*t7.*t9.*t11.*2.0+Lycm6.*Lz5.*dQ2.*dQ6.*m6.*t2.*t8.*t10.*t11.*2.0+Lycm6.*Lz5.*dQ2.*dQ6.*m6.*t3.*t7.*t10.*t11.*2.0+Lycm6.*Lz5.*dQ3.*dQ6.*m6.*t6.*t7.*t8.*t9.*2.0+Lycm6.*Lz5.*dQ3.*dQ6.*m6.*t2.*t8.*t10.*t11.*2.0+Lycm6.*Lz5.*dQ3.*dQ6.*m6.*t3.*t7.*t10.*t11.*2.0-Lycm5.*Lz4.*dQ1.*dQ4.*m5.*t2.*t4.*t7.*t33.*4.0-Lycm5.*Lz4.*dQ1.*dQ4.*m5.*t3.*t4.*t8.*t32.*4.0+Lycm6.*Lz4.*dQ1.*dQ2.*m6.*t4.*t5.*t11.*t32.*4.0+Lycm6.*Lz4.*dQ1.*dQ2.*m6.*t4.*t5.*t11.*t33.*4.0+Lycm6.*Lz4.*dQ1.*dQ3.*m6.*t4.*t5.*t11.*t32.*4.0+Lycm6.*Lz5.*dQ1.*dQ2.*m6.*t5.*t6.*t9.*t32.*4.0+Lycm6.*Lz4.*dQ1.*dQ3.*m6.*t4.*t5.*t11.*t33.*4.0;
et244 = Lycm6.*Lz5.*dQ1.*dQ2.*m6.*t5.*t6.*t9.*t33.*4.0+Lycm6.*Lz5.*dQ1.*dQ3.*m6.*t5.*t6.*t9.*t32.*4.0+Lycm6.*Lz5.*dQ1.*dQ3.*m6.*t5.*t6.*t9.*t33.*4.0+Lycm6.*Lz5.*dQ1.*dQ6.*m6.*t5.*t6.*t10.*t32.*2.0-Lycm6.*Lz5.*dQ4.*dQ5.*m6.*t2.*t3.*t11.*t35.*4.0+Lycm6.*Lz5.*dQ1.*dQ6.*m6.*t5.*t6.*t10.*t33.*2.0+Lycm6.*Lz5.*dQ4.*dQ5.*m6.*t7.*t8.*t11.*t35.*4.0-Lycm6.*Lz4.*dQ1.*dQ2.*m6.*t6.*t9.*t32.*t33.*8.0-Lycm6.*Lz4.*dQ1.*dQ3.*m6.*t6.*t9.*t32.*t33.*8.0+Lycm6.*Lz5.*dQ1.*dQ2.*m6.*t4.*t11.*t32.*t33.*8.0+Lycm6.*Lz5.*dQ1.*dQ3.*m6.*t4.*t11.*t32.*t33.*8.0+Lycm6.*Lz5.*dQ1.*dQ2.*m6.*t4.*t11.*t32.*t35.*8.0-Lycm6.*Lz4.*dQ1.*dQ5.*m6.*t5.*t11.*t32.*t33.*4.0+Lycm6.*Lz5.*dQ1.*dQ2.*m6.*t4.*t11.*t33.*t35.*8.0+Lycm6.*Lz5.*dQ1.*dQ3.*m6.*t4.*t11.*t32.*t35.*8.0+Lycm6.*Lz5.*dQ1.*dQ4.*m6.*t6.*t10.*t32.*t33.*4.0-Lycm6.*Lz4.*dQ1.*dQ6.*m6.*t6.*t10.*t32.*t33.*4.0;
et245 = Lycm6.*Lz5.*dQ1.*dQ3.*m6.*t4.*t11.*t33.*t35.*8.0+Lycm6.*Lz5.*dQ1.*dQ4.*m6.*t6.*t10.*t32.*t34.*4.0+Lycm6.*Lz5.*dQ1.*dQ4.*m6.*t6.*t10.*t33.*t34.*4.0+Lycm6.*Lz5.*dQ1.*dQ5.*m6.*t11.*t32.*t33.*t34.*4.0-Lycm6.*Lz5.*dQ1.*dQ5.*m6.*t11.*t32.*t33.*t35.*8.0+Lycm6.*Lz5.*dQ1.*dQ5.*m6.*t11.*t32.*t34.*t35.*4.0+Lycm6.*Lz5.*dQ1.*dQ5.*m6.*t11.*t33.*t34.*t35.*4.0+Lycm5.*Lzcm5.*dQ1.*dQ4.*m5.*t2.*t4.*t5.*t7.*2.0+Lycm5.*Lzcm5.*dQ2.*dQ3.*m5.*t2.*t4.*t5.*t8.*2.0+Lycm5.*Lzcm5.*dQ2.*dQ3.*m5.*t3.*t4.*t5.*t7.*2.0+Lycm5.*Lzcm5.*dQ1.*dQ4.*m5.*t3.*t4.*t5.*t8.*2.0+Lycm5.*Lzcm5.*dQ2.*dQ5.*m5.*t2.*t3.*t4.*t10.*2.0+Lycm5.*Lzcm5.*dQ3.*dQ5.*m5.*t2.*t3.*t4.*t10.*2.0-Lycm6.*Lzcm6.*dQ1.*dQ6.*m6.*t2.*t4.*t6.*t7.*2.0-Lycm6.*Lzcm6.*dQ2.*dQ3.*m6.*t2.*t3.*t6.*t10.*2.0-Lycm6.*Lzcm6.*dQ1.*dQ6.*m6.*t3.*t4.*t6.*t8.*2.0-Lycm6.*Lzcm6.*dQ2.*dQ6.*m6.*t2.*t3.*t6.*t9.*2.0;
et246 = Lycm6.*Lzcm6.*dQ3.*dQ6.*m6.*t2.*t3.*t6.*t9.*-2.0-Lycm5.*Lzcm5.*dQ1.*dQ5.*m5.*t2.*t7.*t9.*t10.*2.0-Lycm5.*Lzcm5.*dQ1.*dQ5.*m5.*t3.*t8.*t9.*t10.*2.0-Lycm5.*Lzcm5.*dQ2.*dQ5.*m5.*t4.*t7.*t8.*t10.*2.0-Lycm5.*Lzcm5.*dQ3.*dQ5.*m5.*t4.*t7.*t8.*t10.*2.0+Lycm6.*Lzcm6.*dQ1.*dQ4.*m6.*t2.*t7.*t9.*t11.*2.0+Lycm6.*Lzcm6.*dQ2.*dQ3.*m6.*t2.*t8.*t9.*t11.*2.0+Lycm6.*Lzcm6.*dQ2.*dQ3.*m6.*t3.*t7.*t9.*t11.*2.0+Lycm6.*Lzcm6.*dQ1.*dQ4.*m6.*t3.*t8.*t9.*t11.*2.0+Lycm6.*Lzcm6.*dQ2.*dQ3.*m6.*t6.*t7.*t8.*t10.*2.0+Lycm6.*Lzcm6.*dQ2.*dQ6.*m6.*t6.*t7.*t8.*t9.*2.0+Lycm6.*Lzcm6.*dQ2.*dQ6.*m6.*t2.*t8.*t10.*t11.*2.0+Lycm6.*Lzcm6.*dQ2.*dQ6.*m6.*t3.*t7.*t10.*t11.*2.0+Lycm6.*Lzcm6.*dQ3.*dQ6.*m6.*t6.*t7.*t8.*t9.*2.0+Lycm6.*Lzcm6.*dQ3.*dQ6.*m6.*t2.*t8.*t10.*t11.*2.0+Lycm6.*Lzcm6.*dQ3.*dQ6.*m6.*t3.*t7.*t10.*t11.*2.0-Lycm4.*Lzcm4.*dQ1.*dQ4.*m4.*t2.*t4.*t7.*t33.*4.0;
et247 = Lycm4.*Lzcm4.*dQ1.*dQ4.*m4.*t3.*t4.*t8.*t32.*-4.0+Lycm5.*Lzcm5.*dQ2.*dQ3.*m5.*t2.*t3.*t10.*t34.*4.0+Lycm5.*Lzcm5.*dQ1.*dQ5.*m5.*t4.*t5.*t9.*t32.*2.0+Lycm5.*Lzcm5.*dQ2.*dQ5.*m5.*t2.*t5.*t8.*t34.*2.0+Lycm5.*Lzcm5.*dQ2.*dQ5.*m5.*t3.*t5.*t7.*t34.*2.0+Lycm5.*Lzcm5.*dQ1.*dQ5.*m5.*t4.*t5.*t9.*t33.*2.0+Lycm5.*Lzcm5.*dQ3.*dQ5.*m5.*t2.*t5.*t8.*t34.*2.0+Lycm5.*Lzcm5.*dQ3.*dQ5.*m5.*t3.*t5.*t7.*t34.*2.0+Lycm6.*Lzcm6.*dQ1.*dQ2.*m6.*t5.*t6.*t9.*t32.*4.0+Lycm6.*Lzcm6.*dQ1.*dQ2.*m6.*t5.*t6.*t9.*t33.*4.0+Lycm6.*Lzcm6.*dQ1.*dQ3.*m6.*t5.*t6.*t9.*t32.*4.0+Lycm6.*Lzcm6.*dQ1.*dQ3.*m6.*t5.*t6.*t9.*t33.*4.0+Lycm6.*Lzcm6.*dQ1.*dQ6.*m6.*t5.*t6.*t10.*t32.*2.0-Lycm6.*Lzcm6.*dQ4.*dQ5.*m6.*t2.*t3.*t11.*t35.*4.0-Lycm5.*Lzcm5.*dQ2.*dQ3.*m5.*t7.*t8.*t10.*t34.*4.0+Lycm6.*Lzcm6.*dQ1.*dQ6.*m6.*t5.*t6.*t10.*t33.*2.0+Lycm6.*Lzcm6.*dQ4.*dQ5.*m6.*t7.*t8.*t11.*t35.*4.0;
et248 = Lycm5.*Lzcm5.*dQ1.*dQ2.*m5.*t5.*t9.*t32.*t33.*-8.0-Lycm5.*Lzcm5.*dQ1.*dQ3.*m5.*t5.*t9.*t32.*t33.*8.0+Lycm6.*Lzcm6.*dQ1.*dQ2.*m6.*t4.*t11.*t32.*t33.*8.0+Lycm6.*Lzcm6.*dQ1.*dQ3.*m6.*t4.*t11.*t32.*t33.*8.0+Lycm6.*Lzcm6.*dQ1.*dQ2.*m6.*t4.*t11.*t32.*t35.*8.0+Lycm6.*Lzcm6.*dQ1.*dQ2.*m6.*t4.*t11.*t33.*t35.*8.0+Lycm6.*Lzcm6.*dQ1.*dQ3.*m6.*t4.*t11.*t32.*t35.*8.0+Lycm6.*Lzcm6.*dQ1.*dQ4.*m6.*t6.*t10.*t32.*t33.*4.0+Lycm6.*Lzcm6.*dQ1.*dQ3.*m6.*t4.*t11.*t33.*t35.*8.0+Lycm6.*Lzcm6.*dQ1.*dQ4.*m6.*t6.*t10.*t32.*t34.*4.0+Lycm6.*Lzcm6.*dQ1.*dQ4.*m6.*t6.*t10.*t33.*t34.*4.0-Lycm5.*Lzcm5.*dQ1.*dQ4.*m5.*t10.*t32.*t33.*t34.*8.0+Lycm6.*Lzcm6.*dQ1.*dQ5.*m6.*t11.*t32.*t33.*t34.*4.0-Lycm6.*Lzcm6.*dQ1.*dQ5.*m6.*t11.*t32.*t33.*t35.*8.0+Lycm6.*Lzcm6.*dQ1.*dQ5.*m6.*t11.*t32.*t34.*t35.*4.0+Lycm6.*Lzcm6.*dQ1.*dQ5.*m6.*t11.*t33.*t34.*t35.*4.0;
et249 = Lz4.*Lz5.*dQ1.*dQ5.*m6.*t2.*t4.*t5.*t7.*-2.0-Lz4.*Lz5.*dQ1.*dQ5.*m6.*t3.*t4.*t5.*t8.*2.0+Lz4.*Lz5.*dQ4.*dQ5.*m6.*t2.*t4.*t5.*t8.*2.0+Lz4.*Lz5.*dQ4.*dQ5.*m6.*t3.*t4.*t5.*t7.*2.0+Lz4.*Lz5.*dQ1.*dQ4.*m6.*t2.*t7.*t9.*t10.*2.0+Lz4.*Lz5.*dQ2.*dQ3.*m6.*t2.*t8.*t9.*t10.*2.0+Lz4.*Lz5.*dQ2.*dQ3.*m6.*t3.*t7.*t9.*t10.*2.0+Lz4.*Lz5.*dQ1.*dQ4.*m6.*t3.*t8.*t9.*t10.*2.0+Lz4.*Lz5.*dQ1.*dQ2.*m6.*t2.*t5.*t7.*t33.*8.0+Lz4.*Lz5.*dQ1.*dQ2.*m6.*t3.*t5.*t8.*t32.*8.0+Lz4.*Lz5.*dQ1.*dQ3.*m6.*t2.*t5.*t7.*t33.*8.0+Lz4.*Lz5.*dQ1.*dQ3.*m6.*t3.*t5.*t8.*t32.*8.0+Lz4.*Lz5.*dQ1.*dQ2.*m6.*t4.*t10.*t32.*t33.*8.0+Lz4.*Lz5.*dQ1.*dQ3.*m6.*t4.*t10.*t32.*t33.*8.0-Lz4.*Lzcm5.*dQ1.*dQ5.*m5.*t2.*t4.*t5.*t7.*2.0-Lz4.*Lzcm5.*dQ1.*dQ5.*m5.*t3.*t4.*t5.*t8.*2.0-Lz4.*Lzcm6.*dQ1.*dQ5.*m6.*t2.*t4.*t5.*t7.*2.0;
et250 = Lz5.*Lzcm6.*dQ2.*dQ3.*m6.*t2.*t3.*t4.*t9.*4.0+Lz4.*Lzcm5.*dQ4.*dQ5.*m5.*t2.*t4.*t5.*t8.*2.0+Lz4.*Lzcm5.*dQ4.*dQ5.*m5.*t3.*t4.*t5.*t7.*2.0-Lz4.*Lzcm6.*dQ1.*dQ5.*m6.*t3.*t4.*t5.*t8.*2.0+Lz4.*Lzcm6.*dQ4.*dQ5.*m6.*t2.*t4.*t5.*t8.*2.0+Lz4.*Lzcm6.*dQ4.*dQ5.*m6.*t3.*t4.*t5.*t7.*2.0+Lz5.*Lzcm6.*dQ4.*dQ5.*m6.*t2.*t3.*t5.*t10.*4.0+Lz4.*Lzcm5.*dQ1.*dQ4.*m5.*t2.*t7.*t9.*t10.*2.0+Lz4.*Lzcm5.*dQ2.*dQ3.*m5.*t2.*t8.*t9.*t10.*2.0+Lz4.*Lzcm5.*dQ2.*dQ3.*m5.*t3.*t7.*t9.*t10.*2.0+Lz4.*Lzcm5.*dQ1.*dQ4.*m5.*t3.*t8.*t9.*t10.*2.0+Lz4.*Lzcm6.*dQ1.*dQ4.*m6.*t2.*t7.*t9.*t10.*2.0+Lz4.*Lzcm6.*dQ2.*dQ3.*m6.*t2.*t8.*t9.*t10.*2.0+Lz4.*Lzcm6.*dQ2.*dQ3.*m6.*t3.*t7.*t9.*t10.*2.0-Lz5.*Lzcm6.*dQ2.*dQ3.*m6.*t4.*t7.*t8.*t9.*4.0+Lz4.*Lzcm6.*dQ1.*dQ4.*m6.*t3.*t8.*t9.*t10.*2.0-Lz5.*Lzcm6.*dQ4.*dQ5.*m6.*t5.*t7.*t8.*t10.*4.0;
et251 = Lz4.*Lzcm5.*dQ1.*dQ2.*m5.*t2.*t5.*t7.*t33.*8.0+Lz4.*Lzcm5.*dQ1.*dQ2.*m5.*t3.*t5.*t8.*t32.*8.0+Lz4.*Lzcm5.*dQ1.*dQ3.*m5.*t2.*t5.*t7.*t33.*8.0+Lz4.*Lzcm5.*dQ1.*dQ3.*m5.*t3.*t5.*t8.*t32.*8.0+Lz4.*Lzcm6.*dQ1.*dQ2.*m6.*t2.*t5.*t7.*t33.*8.0+Lz4.*Lzcm6.*dQ1.*dQ2.*m6.*t3.*t5.*t8.*t32.*8.0+Lz4.*Lzcm6.*dQ1.*dQ3.*m6.*t2.*t5.*t7.*t33.*8.0+Lz4.*Lzcm6.*dQ1.*dQ3.*m6.*t3.*t5.*t8.*t32.*8.0-Lz5.*Lzcm6.*dQ1.*dQ5.*m6.*t2.*t4.*t7.*t33.*8.0-Lz5.*Lzcm6.*dQ1.*dQ5.*m6.*t3.*t4.*t8.*t32.*8.0-Lz5.*Lzcm6.*dQ1.*dQ2.*m6.*t4.*t5.*t10.*t32.*8.0-Lz5.*Lzcm6.*dQ1.*dQ5.*m6.*t2.*t4.*t7.*t35.*8.0-Lz5.*Lzcm6.*dQ1.*dQ2.*m6.*t4.*t5.*t10.*t33.*8.0-Lz5.*Lzcm6.*dQ1.*dQ3.*m6.*t4.*t5.*t10.*t32.*8.0-Lz5.*Lzcm6.*dQ1.*dQ3.*m6.*t4.*t5.*t10.*t33.*8.0-Lz5.*Lzcm6.*dQ1.*dQ5.*m6.*t3.*t4.*t8.*t35.*8.0;
et252 = Lz5.*Lzcm6.*dQ2.*dQ5.*m6.*t2.*t3.*t9.*t35.*-4.0-Lz5.*Lzcm6.*dQ3.*dQ5.*m6.*t2.*t3.*t9.*t35.*4.0+Lz5.*Lzcm6.*dQ4.*dQ5.*m6.*t2.*t4.*t8.*t35.*4.0+Lz5.*Lzcm6.*dQ4.*dQ5.*m6.*t3.*t4.*t7.*t35.*4.0+Lz5.*Lzcm6.*dQ2.*dQ5.*m6.*t7.*t8.*t9.*t35.*4.0+Lz5.*Lzcm6.*dQ3.*dQ5.*m6.*t7.*t8.*t9.*t35.*4.0+Lz4.*Lzcm5.*dQ1.*dQ2.*m5.*t4.*t10.*t32.*t33.*8.0-Lz5.*Lzcm6.*dQ1.*dQ2.*m6.*t2.*t7.*t33.*t34.*8.0+Lz4.*Lzcm5.*dQ1.*dQ3.*m5.*t4.*t10.*t32.*t33.*8.0+Lz5.*Lzcm6.*dQ1.*dQ2.*m6.*t2.*t7.*t33.*t35.*8.0-Lz5.*Lzcm6.*dQ1.*dQ2.*m6.*t3.*t8.*t32.*t34.*8.0-Lz5.*Lzcm6.*dQ1.*dQ3.*m6.*t2.*t7.*t33.*t34.*8.0+Lz4.*Lzcm6.*dQ1.*dQ2.*m6.*t4.*t10.*t32.*t33.*8.0-Lz5.*Lzcm6.*dQ1.*dQ2.*m6.*t2.*t7.*t34.*t35.*4.0+Lz5.*Lzcm6.*dQ1.*dQ2.*m6.*t3.*t8.*t32.*t35.*8.0+Lz5.*Lzcm6.*dQ1.*dQ3.*m6.*t2.*t7.*t33.*t35.*8.0;
et253 = Lz5.*Lzcm6.*dQ1.*dQ3.*m6.*t3.*t8.*t32.*t34.*-8.0+Lz4.*Lzcm6.*dQ1.*dQ3.*m6.*t4.*t10.*t32.*t33.*8.0-Lz5.*Lzcm6.*dQ1.*dQ3.*m6.*t2.*t7.*t34.*t35.*4.0+Lz5.*Lzcm6.*dQ1.*dQ3.*m6.*t3.*t8.*t32.*t35.*8.0-Lz5.*Lzcm6.*dQ1.*dQ2.*m6.*t3.*t8.*t34.*t35.*4.0-Lz5.*Lzcm6.*dQ1.*dQ4.*m6.*t4.*t9.*t32.*t33.*8.0-Lz5.*Lzcm6.*dQ1.*dQ3.*m6.*t3.*t8.*t34.*t35.*4.0-Lz5.*Lzcm6.*dQ1.*dQ4.*m6.*t4.*t9.*t32.*t35.*4.0-Lz5.*Lzcm6.*dQ2.*dQ4.*m6.*t2.*t8.*t34.*t35.*4.0-Lz5.*Lzcm6.*dQ2.*dQ4.*m6.*t3.*t7.*t34.*t35.*4.0-Lz5.*Lzcm6.*dQ1.*dQ4.*m6.*t4.*t9.*t33.*t35.*4.0+Lz5.*Lzcm6.*dQ1.*dQ5.*m6.*t5.*t10.*t32.*t33.*8.0-Lz5.*Lzcm6.*dQ3.*dQ4.*m6.*t2.*t8.*t34.*t35.*4.0-Lz5.*Lzcm6.*dQ3.*dQ4.*m6.*t3.*t7.*t34.*t35.*4.0-Lz5.*Lzcm6.*dQ1.*dQ5.*m6.*t5.*t10.*t32.*t34.*4.0-Lz5.*Lzcm6.*dQ1.*dQ5.*m6.*t5.*t10.*t33.*t34.*4.0;
et254 = Lx2.*Lxcm5.*dQ1.*dQ2.*m5.*t2.*t3.*t4.*t5.*t7.*-4.0-Lx2.*Lxcm5.*dQ1.*dQ3.*m5.*t2.*t3.*t4.*t5.*t7.*2.0+Lx3.*Lxcm6.*dQ1.*dQ2.*m6.*t2.*t4.*t5.*t6.*t7.*4.0-Lx2.*Lxcm6.*dQ1.*dQ5.*m6.*t2.*t3.*t5.*t6.*t7.*2.0+Lx3.*Lxcm6.*dQ1.*dQ3.*m6.*t2.*t4.*t5.*t6.*t7.*4.0+Lx3.*Lxcm6.*dQ1.*dQ2.*m6.*t3.*t4.*t5.*t6.*t8.*4.0+Lx3.*Lxcm4.*dQ1.*dQ4.*m4.*t2.*t3.*t7.*t8.*t9.*4.0+Lx3.*Lxcm6.*dQ1.*dQ3.*m6.*t3.*t4.*t5.*t6.*t8.*4.0+Lx3.*Lxcm6.*dQ2.*dQ3.*m6.*t2.*t3.*t5.*t6.*t9.*2.0+Lx3.*Lxcm5.*dQ1.*dQ2.*m5.*t2.*t3.*t7.*t8.*t10.*8.0+Lx3.*Lxcm5.*dQ1.*dQ3.*m5.*t2.*t3.*t7.*t8.*t10.*8.0+Lx2.*Lxcm5.*dQ1.*dQ4.*m5.*t2.*t5.*t7.*t8.*t9.*2.0+Lx2.*Lxcm5.*dQ1.*dQ5.*m5.*t2.*t4.*t7.*t8.*t10.*2.0+Lx2.*Lxcm6.*dQ1.*dQ2.*m6.*t2.*t3.*t7.*t9.*t11.*4.0-Lx3.*Lxcm6.*dQ4.*dQ5.*m6.*t2.*t3.*t4.*t6.*t10.*2.0+Lx2.*Lxcm6.*dQ1.*dQ2.*m6.*t2.*t6.*t7.*t8.*t10.*4.0;
et255 = Lx2.*Lxcm6.*dQ1.*dQ3.*m6.*t2.*t3.*t7.*t9.*t11.*2.0-Lx3.*Lxcm6.*dQ4.*dQ6.*m6.*t2.*t3.*t4.*t5.*t11.*2.0+Lx2.*Lxcm6.*dQ1.*dQ3.*m6.*t2.*t6.*t7.*t8.*t10.*2.0+Lx2.*Lxcm6.*dQ1.*dQ4.*m6.*t2.*t4.*t7.*t8.*t11.*2.0+Lx2.*Lxcm6.*dQ1.*dQ6.*m6.*t2.*t6.*t7.*t8.*t9.*2.0+Lx2.*Lxcm6.*dQ1.*dQ6.*m6.*t2.*t3.*t7.*t10.*t11.*2.0-Lx3.*Lxcm6.*dQ2.*dQ3.*m6.*t5.*t6.*t7.*t8.*t9.*2.0+Lx3.*Lxcm6.*dQ4.*dQ5.*m6.*t4.*t6.*t7.*t8.*t10.*2.0+Lx3.*Lxcm6.*dQ4.*dQ6.*m6.*t4.*t5.*t7.*t8.*t11.*2.0+Lx3.*Lxcm6.*dQ5.*dQ6.*m6.*t2.*t3.*t9.*t10.*t11.*2.0-Lx3.*Lxcm5.*dQ1.*dQ2.*m5.*t2.*t4.*t5.*t7.*t33.*8.0-Lx3.*Lxcm5.*dQ1.*dQ2.*m5.*t3.*t4.*t5.*t8.*t32.*8.0-Lx3.*Lxcm5.*dQ1.*dQ3.*m5.*t2.*t4.*t5.*t7.*t33.*8.0-Lx3.*Lxcm5.*dQ1.*dQ3.*m5.*t3.*t4.*t5.*t8.*t32.*8.0-Lx3.*Lxcm6.*dQ5.*dQ6.*m6.*t7.*t8.*t9.*t10.*t11.*2.0;
et256 = Lx2.*Lxcm6.*dQ1.*dQ2.*m6.*t4.*t5.*t6.*t8.*t32.*-4.0-Lx2.*Lxcm6.*dQ1.*dQ3.*m6.*t4.*t5.*t6.*t8.*t32.*2.0-Lx2.*Lxcm6.*dQ1.*dQ4.*m6.*t3.*t5.*t6.*t9.*t32.*2.0-Lx3.*Lxcm6.*dQ1.*dQ5.*m6.*t2.*t5.*t6.*t7.*t33.*4.0-Lx2.*Lxcm6.*dQ1.*dQ5.*m6.*t3.*t4.*t6.*t10.*t32.*2.0-Lx3.*Lxcm6.*dQ1.*dQ5.*m6.*t3.*t5.*t6.*t8.*t32.*4.0-Lx2.*Lxcm6.*dQ1.*dQ6.*m6.*t3.*t4.*t5.*t11.*t32.*2.0+Lx3.*Lxcm6.*dQ1.*dQ2.*m6.*t2.*t7.*t9.*t11.*t33.*8.0+Lx3.*Lxcm6.*dQ1.*dQ2.*m6.*t3.*t8.*t9.*t11.*t32.*8.0+Lx3.*Lxcm6.*dQ1.*dQ3.*m6.*t2.*t7.*t9.*t11.*t33.*8.0+Lx3.*Lxcm6.*dQ1.*dQ3.*m6.*t3.*t8.*t9.*t11.*t32.*8.0+Lx3.*Lxcm6.*dQ1.*dQ6.*m6.*t2.*t7.*t10.*t11.*t33.*4.0+Lx3.*Lxcm6.*dQ1.*dQ6.*m6.*t3.*t8.*t10.*t11.*t32.*4.0-Lx3.*Lxcm6.*dQ1.*dQ4.*m6.*t5.*t6.*t9.*t32.*t33.*4.0-Lx3.*Lxcm6.*dQ1.*dQ5.*m6.*t4.*t6.*t10.*t32.*t33.*4.0;
et257 = Lx3.*Lxcm6.*dQ1.*dQ6.*m6.*t4.*t5.*t11.*t32.*t33.*-4.0+Lx3.*Lycm4.*dQ1.*dQ4.*m4.*t2.*t3.*t4.*t7.*t8.*4.0+Lx3.*Lycm5.*dQ1.*dQ4.*m5.*t2.*t3.*t4.*t7.*t8.*4.0+Lx2.*Lycm6.*dQ1.*dQ2.*m6.*t2.*t3.*t6.*t7.*t9.*4.0+Lx2.*Lycm6.*dQ1.*dQ3.*m6.*t2.*t3.*t6.*t7.*t9.*2.0-Lx3.*Lycm6.*dQ4.*dQ6.*m6.*t2.*t3.*t4.*t5.*t6.*2.0+Lx2.*Lycm6.*dQ1.*dQ4.*m6.*t2.*t4.*t6.*t7.*t8.*2.0-Lx3.*Lycm6.*dQ1.*dQ2.*m6.*t2.*t4.*t5.*t7.*t11.*4.0+Lx2.*Lycm6.*dQ1.*dQ5.*m6.*t2.*t3.*t5.*t7.*t11.*2.0-Lx3.*Lycm6.*dQ1.*dQ3.*m6.*t2.*t4.*t5.*t7.*t11.*4.0+Lx2.*Lycm6.*dQ1.*dQ6.*m6.*t2.*t3.*t6.*t7.*t10.*2.0-Lx3.*Lycm6.*dQ1.*dQ2.*m6.*t3.*t4.*t5.*t8.*t11.*4.0-Lx3.*Lycm6.*dQ1.*dQ3.*m6.*t3.*t4.*t5.*t8.*t11.*4.0-Lx3.*Lycm6.*dQ2.*dQ3.*m6.*t2.*t3.*t5.*t9.*t11.*2.0+Lx3.*Lycm6.*dQ4.*dQ5.*m6.*t2.*t3.*t4.*t10.*t11.*2.0-Lx2.*Lycm6.*dQ1.*dQ2.*m6.*t2.*t7.*t8.*t10.*t11.*4.0;
et258 = Lx3.*Lycm6.*dQ4.*dQ6.*m6.*t4.*t5.*t6.*t7.*t8.*2.0-Lx2.*Lycm6.*dQ1.*dQ3.*m6.*t2.*t7.*t8.*t10.*t11.*2.0+Lx3.*Lycm6.*dQ5.*dQ6.*m6.*t2.*t3.*t6.*t9.*t10.*2.0-Lx2.*Lycm6.*dQ1.*dQ6.*m6.*t2.*t7.*t8.*t9.*t11.*2.0+Lx3.*Lycm6.*dQ2.*dQ3.*m6.*t5.*t7.*t8.*t9.*t11.*2.0-Lx3.*Lycm6.*dQ4.*dQ5.*m6.*t4.*t7.*t8.*t10.*t11.*2.0-Lx3.*Lycm6.*dQ5.*dQ6.*m6.*t6.*t7.*t8.*t9.*t10.*2.0-Lx2.*Lycm6.*dQ1.*dQ6.*m6.*t3.*t4.*t5.*t6.*t32.*2.0+Lx3.*Lycm6.*dQ1.*dQ2.*m6.*t2.*t6.*t7.*t9.*t33.*8.0+Lx3.*Lycm6.*dQ1.*dQ2.*m6.*t3.*t6.*t8.*t9.*t32.*8.0+Lx3.*Lycm6.*dQ1.*dQ3.*m6.*t2.*t6.*t7.*t9.*t33.*8.0+Lx2.*Lycm6.*dQ1.*dQ2.*m6.*t4.*t5.*t8.*t11.*t32.*4.0+Lx3.*Lycm6.*dQ1.*dQ3.*m6.*t3.*t6.*t8.*t9.*t32.*8.0+Lx2.*Lycm6.*dQ1.*dQ3.*m6.*t4.*t5.*t8.*t11.*t32.*2.0+Lx2.*Lycm6.*dQ1.*dQ4.*m6.*t3.*t5.*t9.*t11.*t32.*2.0;
et259 = Lx3.*Lycm6.*dQ1.*dQ5.*m6.*t2.*t5.*t7.*t11.*t33.*4.0+Lx2.*Lycm6.*dQ1.*dQ5.*m6.*t3.*t4.*t10.*t11.*t32.*2.0+Lx3.*Lycm6.*dQ1.*dQ5.*m6.*t3.*t5.*t8.*t11.*t32.*4.0+Lx3.*Lycm6.*dQ1.*dQ6.*m6.*t2.*t6.*t7.*t10.*t33.*4.0+Lx3.*Lycm6.*dQ1.*dQ6.*m6.*t3.*t6.*t8.*t10.*t32.*4.0-Lx3.*Lycm6.*dQ1.*dQ6.*m6.*t4.*t5.*t6.*t32.*t33.*4.0+Lx3.*Lycm6.*dQ1.*dQ4.*m6.*t5.*t9.*t11.*t32.*t33.*4.0+Lx3.*Lycm6.*dQ1.*dQ5.*m6.*t4.*t10.*t11.*t32.*t33.*4.0-Lxcm5.*Lycm5.*dQ1.*dQ2.*m5.*t2.*t4.*t5.*t7.*t9.*4.0-Lxcm5.*Lycm5.*dQ1.*dQ4.*m5.*t2.*t3.*t5.*t7.*t8.*4.0-Lxcm5.*Lycm5.*dQ1.*dQ3.*m5.*t2.*t4.*t5.*t7.*t9.*4.0-Lxcm5.*Lycm5.*dQ1.*dQ2.*m5.*t3.*t4.*t5.*t8.*t9.*4.0-Lxcm5.*Lycm5.*dQ1.*dQ3.*m5.*t3.*t4.*t5.*t8.*t9.*4.0+Lxcm6.*Lycm6.*dQ1.*dQ2.*m6.*t2.*t4.*t5.*t7.*t9.*4.0+Lxcm6.*Lycm6.*dQ1.*dQ4.*m6.*t2.*t3.*t5.*t7.*t8.*4.0-Lxcm5.*Lycm5.*dQ2.*dQ4.*m5.*t2.*t4.*t5.*t8.*t9.*4.0;
et260 = Lxcm5.*Lycm5.*dQ2.*dQ4.*m5.*t3.*t4.*t5.*t7.*t9.*-4.0+Lxcm6.*Lycm6.*dQ1.*dQ3.*m6.*t2.*t4.*t5.*t7.*t9.*4.0-Lxcm5.*Lycm5.*dQ3.*dQ4.*m5.*t2.*t4.*t5.*t8.*t9.*4.0-Lxcm5.*Lycm5.*dQ3.*dQ4.*m5.*t3.*t4.*t5.*t7.*t9.*4.0+Lxcm6.*Lycm6.*dQ1.*dQ2.*m6.*t3.*t4.*t5.*t8.*t9.*4.0+Lxcm6.*Lycm6.*dQ1.*dQ3.*m6.*t3.*t4.*t5.*t8.*t9.*4.0+Lxcm6.*Lycm6.*dQ2.*dQ4.*m6.*t2.*t4.*t5.*t8.*t9.*4.0+Lxcm6.*Lycm6.*dQ2.*dQ4.*m6.*t3.*t4.*t5.*t7.*t9.*4.0+Lxcm6.*Lycm6.*dQ1.*dQ6.*m6.*t2.*t4.*t5.*t7.*t10.*4.0+Lxcm6.*Lycm6.*dQ3.*dQ4.*m6.*t2.*t4.*t5.*t8.*t9.*4.0+Lxcm6.*Lycm6.*dQ3.*dQ4.*m6.*t3.*t4.*t5.*t7.*t9.*4.0+Lxcm6.*Lycm6.*dQ1.*dQ5.*m6.*t2.*t4.*t6.*t7.*t11.*4.0+Lxcm6.*Lycm6.*dQ1.*dQ6.*m6.*t3.*t4.*t5.*t8.*t10.*4.0+Lxcm6.*Lycm6.*dQ2.*dQ6.*m6.*t2.*t3.*t5.*t9.*t10.*2.0+Lxcm6.*Lycm6.*dQ1.*dQ5.*m6.*t3.*t4.*t6.*t8.*t11.*4.0+Lxcm6.*Lycm6.*dQ3.*dQ6.*m6.*t2.*t3.*t5.*t9.*t10.*2.0;
et261 = Lxcm6.*Lycm6.*dQ1.*dQ2.*m6.*t4.*t5.*t6.*t10.*t11.*4.0-Lxcm6.*Lycm6.*dQ4.*dQ6.*m6.*t2.*t4.*t5.*t8.*t10.*2.0-Lxcm6.*Lycm6.*dQ4.*dQ6.*m6.*t3.*t4.*t5.*t7.*t10.*2.0+Lxcm6.*Lycm6.*dQ1.*dQ3.*m6.*t4.*t5.*t6.*t10.*t11.*4.0+Lxcm6.*Lycm6.*dQ2.*dQ6.*m6.*t2.*t5.*t6.*t8.*t11.*4.0+Lxcm6.*Lycm6.*dQ2.*dQ6.*m6.*t3.*t5.*t6.*t7.*t11.*4.0-Lxcm6.*Lycm6.*dQ4.*dQ5.*m6.*t2.*t4.*t6.*t8.*t11.*4.0-Lxcm6.*Lycm6.*dQ4.*dQ5.*m6.*t3.*t4.*t6.*t7.*t11.*4.0+Lxcm6.*Lycm6.*dQ3.*dQ6.*m6.*t2.*t5.*t6.*t8.*t11.*4.0+Lxcm6.*Lycm6.*dQ3.*dQ6.*m6.*t3.*t5.*t6.*t7.*t11.*4.0-Lxcm6.*Lycm6.*dQ5.*dQ6.*m6.*t2.*t3.*t6.*t10.*t11.*4.0-Lxcm6.*Lycm6.*dQ2.*dQ6.*m6.*t5.*t7.*t8.*t9.*t10.*2.0-Lxcm6.*Lycm6.*dQ3.*dQ6.*m6.*t5.*t7.*t8.*t9.*t10.*2.0+Lxcm4.*Lycm4.*dQ1.*dQ2.*m4.*t2.*t4.*t7.*t9.*t33.*8.0+Lxcm4.*Lycm4.*dQ1.*dQ2.*m4.*t3.*t4.*t8.*t9.*t32.*8.0;
et262 = Lxcm4.*Lycm4.*dQ1.*dQ3.*m4.*t2.*t4.*t7.*t9.*t33.*8.0+Lxcm4.*Lycm4.*dQ1.*dQ4.*m4.*t2.*t3.*t7.*t8.*t34.*8.0+Lxcm6.*Lycm6.*dQ5.*dQ6.*m6.*t6.*t7.*t8.*t10.*t11.*4.0+Lxcm4.*Lycm4.*dQ1.*dQ3.*m4.*t3.*t4.*t8.*t9.*t32.*8.0+Lxcm6.*Lycm6.*dQ2.*dQ5.*m6.*t2.*t3.*t4.*t5.*t36.*4.0+Lxcm5.*Lycm5.*dQ1.*dQ4.*m5.*t2.*t4.*t7.*t10.*t33.*4.0+Lxcm6.*Lycm6.*dQ3.*dQ5.*m6.*t2.*t3.*t4.*t5.*t36.*4.0+Lxcm5.*Lycm5.*dQ1.*dQ4.*m5.*t3.*t4.*t8.*t10.*t32.*4.0+Lxcm5.*Lycm5.*dQ1.*dQ5.*m5.*t2.*t5.*t7.*t9.*t33.*4.0+Lxcm5.*Lycm5.*dQ1.*dQ5.*m5.*t3.*t5.*t8.*t9.*t32.*4.0-Lxcm6.*Lycm6.*dQ1.*dQ4.*m6.*t2.*t4.*t7.*t10.*t33.*4.0-Lxcm6.*Lycm6.*dQ1.*dQ6.*m6.*t2.*t3.*t7.*t8.*t34.*4.0-Lxcm6.*Lycm6.*dQ1.*dQ2.*m6.*t2.*t6.*t7.*t11.*t33.*1.6e+1-Lxcm6.*Lycm6.*dQ1.*dQ4.*m6.*t3.*t4.*t8.*t10.*t32.*4.0-Lxcm6.*Lycm6.*dQ1.*dQ5.*m6.*t2.*t5.*t7.*t9.*t33.*4.0;
et263 = Lxcm6.*Lycm6.*dQ1.*dQ6.*m6.*t2.*t3.*t7.*t8.*t35.*-4.0-Lxcm6.*Lycm6.*dQ1.*dQ2.*m6.*t2.*t6.*t7.*t11.*t34.*4.0-Lxcm6.*Lycm6.*dQ1.*dQ2.*m6.*t3.*t6.*t8.*t11.*t32.*1.6e+1-Lxcm6.*Lycm6.*dQ1.*dQ3.*m6.*t2.*t6.*t7.*t11.*t33.*1.6e+1-Lxcm6.*Lycm6.*dQ1.*dQ5.*m6.*t3.*t5.*t8.*t9.*t32.*4.0-Lxcm6.*Lycm6.*dQ1.*dQ6.*m6.*t2.*t3.*t7.*t8.*t36.*1.6e+1-Lxcm6.*Lycm6.*dQ1.*dQ2.*m6.*t2.*t6.*t7.*t11.*t35.*4.0-Lxcm6.*Lycm6.*dQ1.*dQ3.*m6.*t2.*t6.*t7.*t11.*t34.*4.0-Lxcm6.*Lycm6.*dQ1.*dQ3.*m6.*t3.*t6.*t8.*t11.*t32.*1.6e+1-Lxcm6.*Lycm6.*dQ1.*dQ4.*m6.*t2.*t4.*t7.*t10.*t36.*4.0-Lxcm6.*Lycm6.*dQ1.*dQ2.*m6.*t3.*t6.*t8.*t11.*t34.*4.0-Lxcm6.*Lycm6.*dQ1.*dQ3.*m6.*t2.*t6.*t7.*t11.*t35.*4.0-Lxcm6.*Lycm6.*dQ1.*dQ5.*m6.*t2.*t5.*t7.*t9.*t36.*4.0-Lxcm6.*Lycm6.*dQ2.*dQ3.*m6.*t2.*t4.*t8.*t10.*t36.*4.0-Lxcm6.*Lycm6.*dQ2.*dQ3.*m6.*t3.*t4.*t7.*t10.*t36.*4.0;
et264 = Lxcm6.*Lycm6.*dQ1.*dQ2.*m6.*t3.*t6.*t8.*t11.*t35.*-4.0-Lxcm6.*Lycm6.*dQ1.*dQ3.*m6.*t3.*t6.*t8.*t11.*t34.*4.0-Lxcm6.*Lycm6.*dQ1.*dQ4.*m6.*t3.*t4.*t8.*t10.*t36.*4.0-Lxcm6.*Lycm6.*dQ1.*dQ3.*m6.*t3.*t6.*t8.*t11.*t35.*4.0-Lxcm6.*Lycm6.*dQ1.*dQ4.*m6.*t4.*t6.*t9.*t11.*t32.*4.0-Lxcm6.*Lycm6.*dQ1.*dQ5.*m6.*t3.*t5.*t8.*t9.*t36.*4.0-Lxcm6.*Lycm6.*dQ2.*dQ4.*m6.*t2.*t6.*t8.*t11.*t34.*4.0-Lxcm6.*Lycm6.*dQ2.*dQ4.*m6.*t3.*t6.*t7.*t11.*t34.*4.0-Lxcm6.*Lycm6.*dQ2.*dQ5.*m6.*t4.*t5.*t7.*t8.*t36.*4.0-Lxcm6.*Lycm6.*dQ2.*dQ6.*m6.*t2.*t4.*t8.*t9.*t36.*4.0-Lxcm6.*Lycm6.*dQ2.*dQ6.*m6.*t3.*t4.*t7.*t9.*t36.*4.0-Lxcm6.*Lycm6.*dQ1.*dQ4.*m6.*t4.*t6.*t9.*t11.*t33.*4.0+Lxcm6.*Lycm6.*dQ2.*dQ4.*m6.*t2.*t6.*t8.*t11.*t35.*4.0+Lxcm6.*Lycm6.*dQ2.*dQ4.*m6.*t3.*t6.*t7.*t11.*t35.*4.0-Lxcm6.*Lycm6.*dQ3.*dQ4.*m6.*t2.*t6.*t8.*t11.*t34.*4.0;
et265 = Lxcm6.*Lycm6.*dQ3.*dQ4.*m6.*t3.*t6.*t7.*t11.*t34.*-4.0-Lxcm6.*Lycm6.*dQ3.*dQ5.*m6.*t4.*t5.*t7.*t8.*t36.*4.0-Lxcm6.*Lycm6.*dQ3.*dQ6.*m6.*t2.*t4.*t8.*t9.*t36.*4.0-Lxcm6.*Lycm6.*dQ3.*dQ6.*m6.*t3.*t4.*t7.*t9.*t36.*4.0+Lxcm6.*Lycm6.*dQ3.*dQ4.*m6.*t2.*t6.*t8.*t11.*t35.*4.0+Lxcm6.*Lycm6.*dQ3.*dQ4.*m6.*t3.*t6.*t7.*t11.*t35.*4.0-Lxcm6.*Lycm6.*dQ1.*dQ5.*m6.*t5.*t6.*t10.*t11.*t32.*4.0-Lxcm6.*Lycm6.*dQ1.*dQ5.*m6.*t5.*t6.*t10.*t11.*t33.*4.0+Lxcm6.*Lycm6.*dQ2.*dQ3.*m6.*t2.*t3.*t5.*t34.*t36.*8.0+Lxcm5.*Lycm5.*dQ1.*dQ5.*m5.*t4.*t9.*t10.*t32.*t33.*4.0-Lxcm6.*Lycm6.*dQ1.*dQ5.*m6.*t4.*t9.*t10.*t32.*t33.*4.0-Lxcm6.*Lycm6.*dQ2.*dQ3.*m6.*t5.*t7.*t8.*t34.*t36.*8.0-Lxcm6.*Lycm6.*dQ1.*dQ5.*m6.*t4.*t9.*t10.*t32.*t36.*4.0-Lxcm6.*Lycm6.*dQ2.*dQ5.*m6.*t2.*t8.*t10.*t34.*t36.*4.0-Lxcm6.*Lycm6.*dQ2.*dQ5.*m6.*t3.*t7.*t10.*t34.*t36.*4.0;
et266 = Lxcm6.*Lycm6.*dQ1.*dQ5.*m6.*t4.*t9.*t10.*t33.*t36.*-4.0-Lxcm6.*Lycm6.*dQ3.*dQ5.*m6.*t2.*t8.*t10.*t34.*t36.*4.0-Lxcm6.*Lycm6.*dQ3.*dQ5.*m6.*t3.*t7.*t10.*t34.*t36.*4.0+Lxcm6.*Lycm6.*dQ1.*dQ2.*m6.*t9.*t10.*t32.*t33.*t36.*1.6e+1+Lxcm6.*Lycm6.*dQ1.*dQ3.*m6.*t9.*t10.*t32.*t33.*t36.*1.6e+1-Lxcm6.*Lycm6.*dQ1.*dQ4.*m6.*t5.*t32.*t33.*t34.*t36.*1.6e+1-Lxcm6.*Lycm6.*dQ1.*dQ6.*m6.*t32.*t33.*t34.*t35.*t36.*8.0-Lx2.*Lz5.*dQ1.*dQ2.*m6.*t2.*t3.*t4.*t7.*t10.*4.0-Lx3.*Lz5.*dQ1.*dQ2.*m6.*t2.*t3.*t5.*t7.*t8.*8.0-Lx2.*Lz5.*dQ1.*dQ3.*m6.*t2.*t3.*t4.*t7.*t10.*2.0-Lx3.*Lz5.*dQ1.*dQ3.*m6.*t2.*t3.*t5.*t7.*t8.*8.0-Lx2.*Lz5.*dQ1.*dQ5.*m6.*t2.*t4.*t5.*t7.*t8.*2.0+Lx2.*Lz5.*dQ1.*dQ4.*m6.*t2.*t7.*t8.*t9.*t10.*2.0-Lx3.*Lz5.*dQ1.*dQ2.*m6.*t2.*t4.*t7.*t10.*t33.*8.0-Lx3.*Lz5.*dQ1.*dQ2.*m6.*t3.*t4.*t8.*t10.*t32.*8.0;
et267 = Lx3.*Lz5.*dQ1.*dQ3.*m6.*t2.*t4.*t7.*t10.*t33.*-8.0-Lx3.*Lz5.*dQ1.*dQ3.*m6.*t3.*t4.*t8.*t10.*t32.*8.0-Lx2.*Lzcm5.*dQ1.*dQ2.*m5.*t2.*t3.*t4.*t7.*t10.*4.0-Lx3.*Lzcm5.*dQ1.*dQ2.*m5.*t2.*t3.*t5.*t7.*t8.*8.0-Lx2.*Lzcm5.*dQ1.*dQ3.*m5.*t2.*t3.*t4.*t7.*t10.*2.0-Lx3.*Lzcm5.*dQ1.*dQ3.*m5.*t2.*t3.*t5.*t7.*t8.*8.0-Lx2.*Lzcm6.*dQ1.*dQ2.*m6.*t2.*t3.*t4.*t7.*t10.*4.0-Lx3.*Lzcm6.*dQ1.*dQ2.*m6.*t2.*t3.*t5.*t7.*t8.*8.0-Lx2.*Lzcm5.*dQ1.*dQ5.*m5.*t2.*t4.*t5.*t7.*t8.*2.0-Lx2.*Lzcm6.*dQ1.*dQ3.*m6.*t2.*t3.*t4.*t7.*t10.*2.0-Lx3.*Lzcm6.*dQ1.*dQ3.*m6.*t2.*t3.*t5.*t7.*t8.*8.0-Lxcm5.*Lz4.*dQ1.*dQ5.*m5.*t2.*t3.*t5.*t7.*t8.*4.0-Lx2.*Lzcm6.*dQ1.*dQ5.*m6.*t2.*t4.*t5.*t7.*t8.*2.0+Lxcm6.*Lz5.*dQ1.*dQ5.*m6.*t2.*t3.*t6.*t7.*t8.*4.0+Lxcm6.*Lz4.*dQ1.*dQ4.*m6.*t2.*t5.*t6.*t7.*t9.*2.0;
et268 = Lxcm6.*Lz5.*dQ1.*dQ2.*m6.*t2.*t5.*t6.*t7.*t10.*4.0+Lxcm6.*Lz4.*dQ1.*dQ5.*m6.*t2.*t4.*t6.*t7.*t10.*2.0+Lxcm6.*Lz4.*dQ2.*dQ3.*m6.*t2.*t5.*t6.*t8.*t9.*2.0+Lxcm6.*Lz4.*dQ2.*dQ3.*m6.*t3.*t5.*t6.*t7.*t9.*2.0+Lxcm6.*Lz5.*dQ1.*dQ3.*m6.*t2.*t5.*t6.*t7.*t10.*4.0+Lxcm6.*Lz5.*dQ1.*dQ4.*m6.*t2.*t4.*t5.*t7.*t11.*2.0+Lxcm6.*Lz4.*dQ1.*dQ4.*m6.*t3.*t5.*t6.*t8.*t9.*2.0+Lxcm6.*Lz4.*dQ1.*dQ6.*m6.*t2.*t4.*t5.*t7.*t11.*2.0+Lxcm6.*Lz5.*dQ1.*dQ2.*m6.*t3.*t5.*t6.*t8.*t10.*4.0+Lxcm6.*Lz5.*dQ2.*dQ3.*m6.*t2.*t4.*t5.*t8.*t11.*2.0+Lxcm6.*Lz5.*dQ2.*dQ3.*m6.*t3.*t4.*t5.*t7.*t11.*2.0+Lx2.*Lzcm5.*dQ1.*dQ4.*m5.*t2.*t7.*t8.*t9.*t10.*2.0+Lxcm6.*Lz4.*dQ1.*dQ5.*m6.*t3.*t4.*t6.*t8.*t10.*2.0+Lxcm6.*Lz5.*dQ1.*dQ3.*m6.*t3.*t5.*t6.*t8.*t10.*4.0+Lxcm6.*Lz5.*dQ1.*dQ4.*m6.*t3.*t4.*t5.*t8.*t11.*2.0+Lxcm6.*Lz5.*dQ1.*dQ6.*m6.*t2.*t5.*t6.*t7.*t9.*2.0;
et269 = Lxcm6.*Lz5.*dQ2.*dQ5.*m6.*t2.*t4.*t6.*t8.*t9.*-2.0-Lxcm6.*Lz5.*dQ2.*dQ5.*m6.*t3.*t4.*t6.*t7.*t9.*2.0+Lxcm6.*Lz4.*dQ1.*dQ6.*m6.*t3.*t4.*t5.*t8.*t11.*2.0-Lxcm6.*Lz5.*dQ2.*dQ4.*m6.*t2.*t5.*t6.*t8.*t10.*4.0-Lxcm6.*Lz5.*dQ2.*dQ4.*m6.*t3.*t5.*t6.*t7.*t10.*4.0+Lxcm6.*Lz5.*dQ2.*dQ5.*m6.*t2.*t3.*t4.*t10.*t11.*2.0-Lxcm6.*Lz5.*dQ3.*dQ5.*m6.*t2.*t4.*t6.*t8.*t9.*2.0-Lxcm6.*Lz5.*dQ3.*dQ5.*m6.*t3.*t4.*t6.*t7.*t9.*2.0+Lx2.*Lzcm6.*dQ1.*dQ4.*m6.*t2.*t7.*t8.*t9.*t10.*2.0-Lxcm6.*Lz4.*dQ4.*dQ5.*m6.*t2.*t4.*t6.*t8.*t10.*2.0-Lxcm6.*Lz4.*dQ4.*dQ5.*m6.*t3.*t4.*t6.*t7.*t10.*2.0+Lxcm6.*Lz5.*dQ1.*dQ6.*m6.*t3.*t5.*t6.*t8.*t9.*2.0-Lxcm6.*Lz5.*dQ3.*dQ4.*m6.*t2.*t5.*t6.*t8.*t10.*4.0-Lxcm6.*Lz5.*dQ3.*dQ4.*m6.*t3.*t5.*t6.*t7.*t10.*4.0+Lxcm6.*Lz5.*dQ3.*dQ5.*m6.*t2.*t3.*t4.*t10.*t11.*2.0;
et270 = Lxcm6.*Lz4.*dQ4.*dQ6.*m6.*t2.*t4.*t5.*t8.*t11.*-2.0-Lxcm6.*Lz4.*dQ4.*dQ6.*m6.*t3.*t4.*t5.*t7.*t11.*2.0-Lxcm6.*Lz5.*dQ4.*dQ6.*m6.*t2.*t5.*t6.*t8.*t9.*2.0-Lxcm6.*Lz5.*dQ4.*dQ6.*m6.*t3.*t5.*t6.*t7.*t9.*2.0-Lxcm6.*Lz5.*dQ4.*dQ6.*m6.*t2.*t3.*t5.*t10.*t11.*2.0-Lxcm6.*Lz5.*dQ1.*dQ5.*m6.*t2.*t7.*t9.*t10.*t11.*2.0-Lxcm6.*Lz5.*dQ1.*dQ5.*m6.*t3.*t8.*t9.*t10.*t11.*2.0-Lxcm6.*Lz5.*dQ2.*dQ5.*m6.*t4.*t7.*t8.*t10.*t11.*2.0-Lxcm6.*Lz5.*dQ3.*dQ5.*m6.*t4.*t7.*t8.*t10.*t11.*2.0+Lxcm6.*Lz4.*dQ5.*dQ6.*m6.*t2.*t8.*t9.*t10.*t11.*2.0+Lxcm6.*Lz4.*dQ5.*dQ6.*m6.*t3.*t7.*t9.*t10.*t11.*2.0+Lxcm6.*Lz5.*dQ4.*dQ6.*m6.*t5.*t7.*t8.*t10.*t11.*2.0-Lx3.*Lzcm5.*dQ1.*dQ2.*m5.*t2.*t4.*t7.*t10.*t33.*8.0-Lx3.*Lzcm5.*dQ1.*dQ2.*m5.*t3.*t4.*t8.*t10.*t32.*8.0-Lx3.*Lzcm5.*dQ1.*dQ3.*m5.*t2.*t4.*t7.*t10.*t33.*8.0;
et271 = Lx3.*Lzcm5.*dQ1.*dQ3.*m5.*t3.*t4.*t8.*t10.*t32.*-8.0-Lx3.*Lzcm6.*dQ1.*dQ2.*m6.*t2.*t4.*t7.*t10.*t33.*8.0-Lx3.*Lzcm6.*dQ1.*dQ2.*m6.*t3.*t4.*t8.*t10.*t32.*8.0-Lx3.*Lzcm6.*dQ1.*dQ3.*m6.*t2.*t4.*t7.*t10.*t33.*8.0-Lxcm5.*Lz4.*dQ1.*dQ4.*m5.*t2.*t5.*t7.*t9.*t33.*4.0-Lx3.*Lzcm6.*dQ1.*dQ3.*m6.*t3.*t4.*t8.*t10.*t32.*8.0-Lxcm5.*Lz4.*dQ1.*dQ4.*m5.*t3.*t5.*t8.*t9.*t32.*4.0-Lxcm5.*Lz4.*dQ1.*dQ5.*m5.*t2.*t4.*t7.*t10.*t33.*4.0-Lxcm5.*Lz4.*dQ1.*dQ5.*m5.*t3.*t4.*t8.*t10.*t32.*4.0-Lxcm6.*Lz4.*dQ1.*dQ2.*m6.*t2.*t6.*t7.*t10.*t33.*8.0-Lxcm6.*Lz4.*dQ1.*dQ2.*m6.*t3.*t6.*t8.*t10.*t32.*8.0-Lxcm6.*Lz4.*dQ1.*dQ3.*m6.*t2.*t6.*t7.*t10.*t33.*8.0-Lxcm6.*Lz4.*dQ1.*dQ4.*m6.*t2.*t4.*t7.*t11.*t33.*4.0-Lxcm6.*Lz4.*dQ1.*dQ3.*m6.*t3.*t6.*t8.*t10.*t32.*8.0;
et272 = Lxcm6.*Lz4.*dQ1.*dQ4.*m6.*t3.*t4.*t8.*t11.*t32.*-4.0+Lxcm6.*Lz5.*dQ1.*dQ4.*m6.*t2.*t6.*t7.*t9.*t33.*4.0-Lxcm6.*Lz4.*dQ1.*dQ6.*m6.*t2.*t6.*t7.*t9.*t33.*4.0+Lxcm6.*Lz5.*dQ1.*dQ4.*m6.*t3.*t6.*t8.*t9.*t32.*4.0-Lxcm6.*Lz4.*dQ1.*dQ6.*m6.*t3.*t6.*t8.*t9.*t32.*4.0+Lxcm6.*Lz5.*dQ1.*dQ4.*m6.*t2.*t6.*t7.*t9.*t35.*4.0+Lxcm6.*Lz5.*dQ1.*dQ6.*m6.*t2.*t4.*t7.*t11.*t33.*4.0+Lxcm6.*Lz5.*dQ1.*dQ6.*m6.*t3.*t4.*t8.*t11.*t32.*4.0+Lxcm6.*Lz5.*dQ2.*dQ3.*m6.*t2.*t3.*t10.*t11.*t34.*4.0+Lxcm6.*Lz5.*dQ2.*dQ3.*m6.*t2.*t6.*t8.*t9.*t35.*4.0+Lxcm6.*Lz5.*dQ2.*dQ3.*m6.*t3.*t6.*t7.*t9.*t35.*4.0+Lxcm6.*Lz5.*dQ1.*dQ4.*m6.*t3.*t6.*t8.*t9.*t35.*4.0+Lxcm6.*Lz5.*dQ1.*dQ6.*m6.*t2.*t4.*t7.*t11.*t35.*4.0+Lxcm6.*Lz5.*dQ1.*dQ5.*m6.*t4.*t5.*t9.*t11.*t32.*2.0+Lxcm6.*Lz5.*dQ2.*dQ5.*m6.*t2.*t5.*t8.*t11.*t34.*2.0+Lxcm6.*Lz5.*dQ2.*dQ5.*m6.*t3.*t5.*t7.*t11.*t34.*2.0;
et273 = Lxcm6.*Lz5.*dQ1.*dQ5.*m6.*t4.*t5.*t9.*t11.*t33.*2.0+Lxcm6.*Lz5.*dQ1.*dQ6.*m6.*t3.*t4.*t8.*t11.*t35.*4.0+Lxcm6.*Lz5.*dQ1.*dQ6.*m6.*t4.*t6.*t9.*t10.*t32.*2.0+Lxcm6.*Lz5.*dQ2.*dQ6.*m6.*t2.*t3.*t9.*t11.*t35.*2.0+Lxcm6.*Lz5.*dQ2.*dQ6.*m6.*t2.*t6.*t8.*t10.*t34.*2.0+Lxcm6.*Lz5.*dQ2.*dQ6.*m6.*t3.*t6.*t7.*t10.*t34.*2.0+Lxcm6.*Lz5.*dQ3.*dQ5.*m6.*t2.*t5.*t8.*t11.*t34.*2.0+Lxcm6.*Lz5.*dQ3.*dQ5.*m6.*t3.*t5.*t7.*t11.*t34.*2.0+Lxcm6.*Lz5.*dQ1.*dQ6.*m6.*t4.*t6.*t9.*t10.*t33.*2.0+Lxcm6.*Lz5.*dQ3.*dQ6.*m6.*t2.*t3.*t9.*t11.*t35.*2.0+Lxcm6.*Lz5.*dQ3.*dQ6.*m6.*t2.*t6.*t8.*t10.*t34.*2.0+Lxcm6.*Lz5.*dQ3.*dQ6.*m6.*t3.*t6.*t7.*t10.*t34.*2.0-Lxcm6.*Lz5.*dQ4.*dQ6.*m6.*t2.*t4.*t8.*t11.*t35.*2.0-Lxcm6.*Lz5.*dQ4.*dQ6.*m6.*t3.*t4.*t7.*t11.*t35.*2.0-Lxcm6.*Lz5.*dQ2.*dQ3.*m6.*t7.*t8.*t10.*t11.*t34.*4.0-Lxcm6.*Lz5.*dQ2.*dQ6.*m6.*t7.*t8.*t9.*t11.*t35.*2.0;
et274 = Lxcm6.*Lz5.*dQ3.*dQ6.*m6.*t7.*t8.*t9.*t11.*t35.*-2.0+Lxcm6.*Lz4.*dQ1.*dQ2.*m6.*t4.*t5.*t6.*t32.*t33.*8.0+Lxcm6.*Lz4.*dQ1.*dQ3.*m6.*t4.*t5.*t6.*t32.*t33.*8.0-Lxcm6.*Lz5.*dQ1.*dQ2.*m6.*t5.*t9.*t11.*t32.*t33.*8.0-Lxcm6.*Lz5.*dQ1.*dQ3.*m6.*t5.*t9.*t11.*t32.*t33.*8.0-Lxcm6.*Lz5.*dQ1.*dQ6.*m6.*t5.*t10.*t11.*t32.*t33.*4.0+Lxcm6.*Lz5.*dQ1.*dQ6.*m6.*t5.*t10.*t11.*t32.*t34.*2.0+Lxcm6.*Lz5.*dQ1.*dQ6.*m6.*t5.*t10.*t11.*t33.*t34.*2.0+Lxcm6.*Lz5.*dQ1.*dQ2.*m6.*t4.*t6.*t32.*t33.*t35.*1.6e+1+Lxcm6.*Lz5.*dQ1.*dQ3.*m6.*t4.*t6.*t32.*t33.*t35.*1.6e+1-Lxcm6.*Lz5.*dQ1.*dQ4.*m6.*t10.*t11.*t32.*t33.*t34.*8.0+Lxcm6.*Lz5.*dQ1.*dQ5.*m6.*t6.*t32.*t33.*t34.*t35.*8.0-Lxcm4.*Lzcm4.*dQ1.*dQ2.*m4.*t2.*t3.*t4.*t7.*t8.*8.0-Lxcm4.*Lzcm4.*dQ1.*dQ3.*m4.*t2.*t3.*t4.*t7.*t8.*8.0+Lxcm5.*Lzcm5.*dQ1.*dQ2.*m5.*t2.*t3.*t4.*t7.*t8.*8.0;
et275 = Lxcm5.*Lzcm5.*dQ1.*dQ3.*m5.*t2.*t3.*t4.*t7.*t8.*8.0+Lxcm5.*Lzcm5.*dQ1.*dQ5.*m5.*t2.*t4.*t5.*t7.*t10.*8.0+Lxcm6.*Lzcm6.*dQ1.*dQ5.*m6.*t2.*t3.*t6.*t7.*t8.*4.0+Lxcm5.*Lzcm5.*dQ1.*dQ5.*m5.*t3.*t4.*t5.*t8.*t10.*8.0+Lxcm5.*Lzcm5.*dQ2.*dQ5.*m5.*t2.*t3.*t5.*t9.*t10.*4.0+Lxcm6.*Lzcm6.*dQ1.*dQ2.*m6.*t2.*t5.*t6.*t7.*t10.*4.0+Lxcm5.*Lzcm5.*dQ3.*dQ5.*m5.*t2.*t3.*t5.*t9.*t10.*4.0+Lxcm6.*Lzcm6.*dQ1.*dQ3.*m6.*t2.*t5.*t6.*t7.*t10.*4.0+Lxcm6.*Lzcm6.*dQ1.*dQ4.*m6.*t2.*t4.*t5.*t7.*t11.*2.0-Lxcm5.*Lzcm5.*dQ4.*dQ5.*m5.*t2.*t4.*t5.*t8.*t10.*4.0-Lxcm5.*Lzcm5.*dQ4.*dQ5.*m5.*t3.*t4.*t5.*t7.*t10.*4.0+Lxcm6.*Lzcm6.*dQ1.*dQ2.*m6.*t3.*t5.*t6.*t8.*t10.*4.0+Lxcm6.*Lzcm6.*dQ2.*dQ3.*m6.*t2.*t4.*t5.*t8.*t11.*2.0+Lxcm6.*Lzcm6.*dQ2.*dQ3.*m6.*t3.*t4.*t5.*t7.*t11.*2.0+Lxcm6.*Lzcm6.*dQ1.*dQ3.*m6.*t3.*t5.*t6.*t8.*t10.*4.0+Lxcm6.*Lzcm6.*dQ1.*dQ4.*m6.*t3.*t4.*t5.*t8.*t11.*2.0;
et276 = Lxcm6.*Lzcm6.*dQ1.*dQ6.*m6.*t2.*t5.*t6.*t7.*t9.*2.0-Lxcm6.*Lzcm6.*dQ2.*dQ5.*m6.*t2.*t4.*t6.*t8.*t9.*2.0-Lxcm6.*Lzcm6.*dQ2.*dQ5.*m6.*t3.*t4.*t6.*t7.*t9.*2.0-Lxcm6.*Lzcm6.*dQ2.*dQ4.*m6.*t2.*t5.*t6.*t8.*t10.*4.0-Lxcm6.*Lzcm6.*dQ2.*dQ4.*m6.*t3.*t5.*t6.*t7.*t10.*4.0+Lxcm6.*Lzcm6.*dQ2.*dQ5.*m6.*t2.*t3.*t4.*t10.*t11.*2.0-Lxcm6.*Lzcm6.*dQ3.*dQ5.*m6.*t2.*t4.*t6.*t8.*t9.*2.0-Lxcm6.*Lzcm6.*dQ3.*dQ5.*m6.*t3.*t4.*t6.*t7.*t9.*2.0+Lxcm6.*Lzcm6.*dQ1.*dQ6.*m6.*t3.*t5.*t6.*t8.*t9.*2.0-Lxcm6.*Lzcm6.*dQ3.*dQ4.*m6.*t2.*t5.*t6.*t8.*t10.*4.0-Lxcm6.*Lzcm6.*dQ3.*dQ4.*m6.*t3.*t5.*t6.*t7.*t10.*4.0+Lxcm6.*Lzcm6.*dQ3.*dQ5.*m6.*t2.*t3.*t4.*t10.*t11.*2.0-Lxcm6.*Lzcm6.*dQ4.*dQ6.*m6.*t2.*t5.*t6.*t8.*t9.*2.0-Lxcm6.*Lzcm6.*dQ4.*dQ6.*m6.*t3.*t5.*t6.*t7.*t9.*2.0-Lxcm6.*Lzcm6.*dQ4.*dQ6.*m6.*t2.*t3.*t5.*t10.*t11.*2.0;
et277 = Lxcm5.*Lzcm5.*dQ2.*dQ5.*m5.*t5.*t7.*t8.*t9.*t10.*-4.0-Lxcm5.*Lzcm5.*dQ3.*dQ5.*m5.*t5.*t7.*t8.*t9.*t10.*4.0-Lxcm6.*Lzcm6.*dQ1.*dQ5.*m6.*t2.*t7.*t9.*t10.*t11.*2.0-Lxcm6.*Lzcm6.*dQ1.*dQ5.*m6.*t3.*t8.*t9.*t10.*t11.*2.0-Lxcm6.*Lzcm6.*dQ2.*dQ5.*m6.*t4.*t7.*t8.*t10.*t11.*2.0-Lxcm6.*Lzcm6.*dQ3.*dQ5.*m6.*t4.*t7.*t8.*t10.*t11.*2.0+Lxcm6.*Lzcm6.*dQ4.*dQ6.*m6.*t5.*t7.*t8.*t10.*t11.*2.0-Lxcm5.*Lzcm5.*dQ1.*dQ2.*m5.*t2.*t5.*t7.*t10.*t33.*8.0+Lxcm5.*Lzcm5.*dQ1.*dQ5.*m5.*t2.*t3.*t7.*t8.*t34.*4.0+Lxcm5.*Lzcm5.*dQ1.*dQ2.*m5.*t2.*t5.*t7.*t10.*t34.*4.0-Lxcm5.*Lzcm5.*dQ1.*dQ2.*m5.*t3.*t5.*t8.*t10.*t32.*8.0-Lxcm5.*Lzcm5.*dQ1.*dQ3.*m5.*t2.*t5.*t7.*t10.*t33.*8.0-Lxcm5.*Lzcm5.*dQ1.*dQ5.*m5.*t2.*t3.*t7.*t8.*t35.*8.0+Lxcm5.*Lzcm5.*dQ1.*dQ3.*m5.*t2.*t5.*t7.*t10.*t34.*4.0-Lxcm5.*Lzcm5.*dQ1.*dQ3.*m5.*t3.*t5.*t8.*t10.*t32.*8.0;
et278 = Lxcm5.*Lzcm5.*dQ1.*dQ2.*m5.*t3.*t5.*t8.*t10.*t34.*4.0+Lxcm5.*Lzcm5.*dQ1.*dQ3.*m5.*t3.*t5.*t8.*t10.*t34.*4.0+Lxcm5.*Lzcm5.*dQ1.*dQ4.*m5.*t4.*t5.*t9.*t10.*t32.*4.0+Lxcm5.*Lzcm5.*dQ2.*dQ4.*m5.*t2.*t5.*t8.*t10.*t34.*4.0+Lxcm5.*Lzcm5.*dQ2.*dQ4.*m5.*t3.*t5.*t7.*t10.*t34.*4.0+Lxcm6.*Lzcm6.*dQ1.*dQ4.*m6.*t2.*t6.*t7.*t9.*t33.*4.0+Lxcm5.*Lzcm5.*dQ1.*dQ4.*m5.*t4.*t5.*t9.*t10.*t33.*4.0+Lxcm5.*Lzcm5.*dQ3.*dQ4.*m5.*t2.*t5.*t8.*t10.*t34.*4.0+Lxcm5.*Lzcm5.*dQ3.*dQ4.*m5.*t3.*t5.*t7.*t10.*t34.*4.0+Lxcm6.*Lzcm6.*dQ1.*dQ4.*m6.*t3.*t6.*t8.*t9.*t32.*4.0+Lxcm6.*Lzcm6.*dQ1.*dQ4.*m6.*t2.*t6.*t7.*t9.*t35.*4.0+Lxcm6.*Lzcm6.*dQ1.*dQ6.*m6.*t2.*t4.*t7.*t11.*t33.*4.0+Lxcm6.*Lzcm6.*dQ1.*dQ6.*m6.*t3.*t4.*t8.*t11.*t32.*4.0+Lxcm6.*Lzcm6.*dQ2.*dQ3.*m6.*t2.*t3.*t10.*t11.*t34.*4.0+Lxcm6.*Lzcm6.*dQ2.*dQ3.*m6.*t2.*t6.*t8.*t9.*t35.*4.0+Lxcm6.*Lzcm6.*dQ2.*dQ3.*m6.*t3.*t6.*t7.*t9.*t35.*4.0;
et279 = Lxcm6.*Lzcm6.*dQ1.*dQ4.*m6.*t3.*t6.*t8.*t9.*t35.*4.0+Lxcm6.*Lzcm6.*dQ1.*dQ6.*m6.*t2.*t4.*t7.*t11.*t35.*4.0+Lxcm6.*Lzcm6.*dQ1.*dQ5.*m6.*t4.*t5.*t9.*t11.*t32.*2.0+Lxcm6.*Lzcm6.*dQ2.*dQ5.*m6.*t2.*t5.*t8.*t11.*t34.*2.0+Lxcm6.*Lzcm6.*dQ2.*dQ5.*m6.*t3.*t5.*t7.*t11.*t34.*2.0+Lxcm6.*Lzcm6.*dQ1.*dQ5.*m6.*t4.*t5.*t9.*t11.*t33.*2.0+Lxcm6.*Lzcm6.*dQ1.*dQ6.*m6.*t3.*t4.*t8.*t11.*t35.*4.0+Lxcm6.*Lzcm6.*dQ1.*dQ6.*m6.*t4.*t6.*t9.*t10.*t32.*2.0+Lxcm6.*Lzcm6.*dQ2.*dQ6.*m6.*t2.*t3.*t9.*t11.*t35.*2.0+Lxcm6.*Lzcm6.*dQ2.*dQ6.*m6.*t2.*t6.*t8.*t10.*t34.*2.0+Lxcm6.*Lzcm6.*dQ2.*dQ6.*m6.*t3.*t6.*t7.*t10.*t34.*2.0+Lxcm6.*Lzcm6.*dQ3.*dQ5.*m6.*t2.*t5.*t8.*t11.*t34.*2.0+Lxcm6.*Lzcm6.*dQ3.*dQ5.*m6.*t3.*t5.*t7.*t11.*t34.*2.0+Lxcm6.*Lzcm6.*dQ1.*dQ6.*m6.*t4.*t6.*t9.*t10.*t33.*2.0+Lxcm6.*Lzcm6.*dQ3.*dQ6.*m6.*t2.*t3.*t9.*t11.*t35.*2.0+Lxcm6.*Lzcm6.*dQ3.*dQ6.*m6.*t2.*t6.*t8.*t10.*t34.*2.0;
et280 = Lxcm6.*Lzcm6.*dQ3.*dQ6.*m6.*t3.*t6.*t7.*t10.*t34.*2.0-Lxcm6.*Lzcm6.*dQ4.*dQ6.*m6.*t2.*t4.*t8.*t11.*t35.*2.0-Lxcm6.*Lzcm6.*dQ4.*dQ6.*m6.*t3.*t4.*t7.*t11.*t35.*2.0-Lxcm6.*Lzcm6.*dQ2.*dQ3.*m6.*t7.*t8.*t10.*t11.*t34.*4.0-Lxcm6.*Lzcm6.*dQ2.*dQ6.*m6.*t7.*t8.*t9.*t11.*t35.*2.0-Lxcm6.*Lzcm6.*dQ3.*dQ6.*m6.*t7.*t8.*t9.*t11.*t35.*2.0-Lxcm5.*Lzcm5.*dQ1.*dQ4.*m5.*t2.*t7.*t9.*t33.*t35.*8.0-Lxcm5.*Lzcm5.*dQ1.*dQ4.*m5.*t3.*t8.*t9.*t32.*t35.*8.0-Lxcm6.*Lzcm6.*dQ1.*dQ2.*m6.*t5.*t9.*t11.*t32.*t33.*8.0-Lxcm6.*Lzcm6.*dQ1.*dQ3.*m6.*t5.*t9.*t11.*t32.*t33.*8.0-Lxcm6.*Lzcm6.*dQ1.*dQ6.*m6.*t5.*t10.*t11.*t32.*t33.*4.0+Lxcm6.*Lzcm6.*dQ1.*dQ6.*m6.*t5.*t10.*t11.*t32.*t34.*2.0+Lxcm6.*Lzcm6.*dQ1.*dQ6.*m6.*t5.*t10.*t11.*t33.*t34.*2.0+Lxcm6.*Lzcm6.*dQ1.*dQ2.*m6.*t4.*t6.*t32.*t33.*t35.*1.6e+1+Lxcm6.*Lzcm6.*dQ1.*dQ3.*m6.*t4.*t6.*t32.*t33.*t35.*1.6e+1;
et281 = Lxcm6.*Lzcm6.*dQ1.*dQ4.*m6.*t10.*t11.*t32.*t33.*t34.*-8.0+Lxcm6.*Lzcm6.*dQ1.*dQ5.*m6.*t6.*t32.*t33.*t34.*t35.*8.0+Lycm5.*Lz4.*dQ1.*dQ2.*m5.*t2.*t3.*t7.*t8.*t9.*8.0+Lycm6.*Lz5.*dQ1.*dQ4.*m6.*t2.*t4.*t5.*t6.*t7.*2.0+Lycm5.*Lz4.*dQ1.*dQ3.*m5.*t2.*t3.*t7.*t8.*t9.*8.0+Lycm6.*Lz4.*dQ1.*dQ6.*m6.*t2.*t4.*t5.*t6.*t7.*2.0+Lycm6.*Lz5.*dQ2.*dQ3.*m6.*t2.*t4.*t5.*t6.*t8.*2.0+Lycm6.*Lz5.*dQ2.*dQ3.*m6.*t3.*t4.*t5.*t6.*t7.*2.0+Lycm6.*Lz5.*dQ1.*dQ4.*m6.*t3.*t4.*t5.*t6.*t8.*2.0+Lycm6.*Lz4.*dQ1.*dQ6.*m6.*t3.*t4.*t5.*t6.*t8.*2.0+Lycm6.*Lz5.*dQ2.*dQ5.*m6.*t2.*t3.*t4.*t6.*t10.*2.0+Lycm6.*Lz5.*dQ3.*dQ5.*m6.*t2.*t3.*t4.*t6.*t10.*2.0-Lycm6.*Lz4.*dQ4.*dQ6.*m6.*t2.*t4.*t5.*t6.*t8.*2.0-Lycm6.*Lz4.*dQ4.*dQ6.*m6.*t3.*t4.*t5.*t6.*t7.*2.0-Lycm6.*Lz5.*dQ4.*dQ6.*m6.*t2.*t3.*t5.*t6.*t10.*2.0;
et282 = Lycm6.*Lz5.*dQ1.*dQ5.*m6.*t2.*t3.*t7.*t8.*t11.*-4.0-Lycm6.*Lz4.*dQ1.*dQ4.*m6.*t2.*t5.*t7.*t9.*t11.*2.0-Lycm6.*Lz5.*dQ1.*dQ2.*m6.*t2.*t5.*t7.*t10.*t11.*4.0-Lycm6.*Lz4.*dQ1.*dQ5.*m6.*t2.*t4.*t7.*t10.*t11.*2.0-Lycm6.*Lz4.*dQ2.*dQ3.*m6.*t2.*t5.*t8.*t9.*t11.*2.0-Lycm6.*Lz4.*dQ2.*dQ3.*m6.*t3.*t5.*t7.*t9.*t11.*2.0-Lycm6.*Lz5.*dQ1.*dQ3.*m6.*t2.*t5.*t7.*t10.*t11.*4.0-Lycm6.*Lz4.*dQ1.*dQ4.*m6.*t3.*t5.*t8.*t9.*t11.*2.0-Lycm6.*Lz5.*dQ1.*dQ2.*m6.*t3.*t5.*t8.*t10.*t11.*4.0-Lycm6.*Lz5.*dQ1.*dQ5.*m6.*t2.*t6.*t7.*t9.*t10.*2.0-Lycm6.*Lz4.*dQ1.*dQ5.*m6.*t3.*t4.*t8.*t10.*t11.*2.0-Lycm6.*Lz5.*dQ1.*dQ3.*m6.*t3.*t5.*t8.*t10.*t11.*4.0-Lycm6.*Lz5.*dQ1.*dQ6.*m6.*t2.*t5.*t7.*t9.*t11.*2.0-Lycm6.*Lz5.*dQ1.*dQ5.*m6.*t3.*t6.*t8.*t9.*t10.*2.0+Lycm6.*Lz5.*dQ2.*dQ4.*m6.*t2.*t5.*t8.*t10.*t11.*4.0;
et283 = Lycm6.*Lz5.*dQ2.*dQ4.*m6.*t3.*t5.*t7.*t10.*t11.*4.0-Lycm6.*Lz5.*dQ2.*dQ5.*m6.*t4.*t6.*t7.*t8.*t10.*2.0+Lycm6.*Lz4.*dQ4.*dQ5.*m6.*t2.*t4.*t8.*t10.*t11.*2.0+Lycm6.*Lz4.*dQ4.*dQ5.*m6.*t3.*t4.*t7.*t10.*t11.*2.0-Lycm6.*Lz5.*dQ1.*dQ6.*m6.*t3.*t5.*t8.*t9.*t11.*2.0+Lycm6.*Lz5.*dQ3.*dQ4.*m6.*t2.*t5.*t8.*t10.*t11.*4.0+Lycm6.*Lz5.*dQ3.*dQ4.*m6.*t3.*t5.*t7.*t10.*t11.*4.0-Lycm6.*Lz5.*dQ3.*dQ5.*m6.*t4.*t6.*t7.*t8.*t10.*2.0+Lycm6.*Lz4.*dQ5.*dQ6.*m6.*t2.*t6.*t8.*t9.*t10.*2.0+Lycm6.*Lz4.*dQ5.*dQ6.*m6.*t3.*t6.*t7.*t9.*t10.*2.0+Lycm6.*Lz5.*dQ4.*dQ6.*m6.*t2.*t5.*t8.*t9.*t11.*2.0+Lycm6.*Lz5.*dQ4.*dQ6.*m6.*t3.*t5.*t7.*t9.*t11.*2.0+Lycm6.*Lz5.*dQ4.*dQ6.*m6.*t5.*t6.*t7.*t8.*t10.*2.0-Lycm6.*Lz4.*dQ1.*dQ4.*m6.*t2.*t4.*t6.*t7.*t33.*4.0-Lycm6.*Lz4.*dQ1.*dQ4.*m6.*t3.*t4.*t6.*t8.*t32.*4.0+Lycm6.*Lz5.*dQ1.*dQ6.*m6.*t2.*t4.*t6.*t7.*t33.*4.0;
et284 = Lycm6.*Lz5.*dQ1.*dQ6.*m6.*t3.*t4.*t6.*t8.*t32.*4.0+Lycm6.*Lz5.*dQ2.*dQ3.*m6.*t2.*t3.*t6.*t10.*t34.*4.0+Lycm6.*Lz5.*dQ1.*dQ6.*m6.*t2.*t4.*t6.*t7.*t35.*4.0+Lycm6.*Lz5.*dQ1.*dQ5.*m6.*t4.*t5.*t6.*t9.*t32.*2.0+Lycm6.*Lz5.*dQ2.*dQ5.*m6.*t2.*t5.*t6.*t8.*t34.*2.0+Lycm6.*Lz5.*dQ2.*dQ5.*m6.*t3.*t5.*t6.*t7.*t34.*2.0+Lycm6.*Lz5.*dQ1.*dQ5.*m6.*t4.*t5.*t6.*t9.*t33.*2.0+Lycm6.*Lz5.*dQ1.*dQ6.*m6.*t3.*t4.*t6.*t8.*t35.*4.0+Lycm6.*Lz5.*dQ2.*dQ6.*m6.*t2.*t3.*t6.*t9.*t35.*2.0+Lycm6.*Lz5.*dQ3.*dQ5.*m6.*t2.*t5.*t6.*t8.*t34.*2.0+Lycm6.*Lz5.*dQ3.*dQ5.*m6.*t3.*t5.*t6.*t7.*t34.*2.0+Lycm6.*Lz5.*dQ3.*dQ6.*m6.*t2.*t3.*t6.*t9.*t35.*2.0+Lycm6.*Lz4.*dQ1.*dQ2.*m6.*t2.*t7.*t10.*t11.*t33.*8.0-Lycm6.*Lz5.*dQ4.*dQ6.*m6.*t2.*t4.*t6.*t8.*t35.*2.0-Lycm6.*Lz5.*dQ4.*dQ6.*m6.*t3.*t4.*t6.*t7.*t35.*2.0+Lycm6.*Lz4.*dQ1.*dQ2.*m6.*t3.*t8.*t10.*t11.*t32.*8.0;
et285 = Lycm6.*Lz4.*dQ1.*dQ3.*m6.*t2.*t7.*t10.*t11.*t33.*8.0+Lycm6.*Lz4.*dQ1.*dQ3.*m6.*t3.*t8.*t10.*t11.*t32.*8.0-Lycm6.*Lz5.*dQ1.*dQ4.*m6.*t2.*t7.*t9.*t11.*t33.*4.0+Lycm6.*Lz4.*dQ1.*dQ6.*m6.*t2.*t7.*t9.*t11.*t33.*4.0-Lycm6.*Lz5.*dQ1.*dQ4.*m6.*t3.*t8.*t9.*t11.*t32.*4.0+Lycm6.*Lz4.*dQ1.*dQ6.*m6.*t3.*t8.*t9.*t11.*t32.*4.0-Lycm6.*Lz5.*dQ1.*dQ4.*m6.*t2.*t7.*t9.*t11.*t35.*4.0-Lycm6.*Lz5.*dQ2.*dQ3.*m6.*t2.*t8.*t9.*t11.*t35.*4.0-Lycm6.*Lz5.*dQ2.*dQ3.*m6.*t3.*t7.*t9.*t11.*t35.*4.0-Lycm6.*Lz5.*dQ2.*dQ3.*m6.*t6.*t7.*t8.*t10.*t34.*4.0-Lycm6.*Lz5.*dQ1.*dQ4.*m6.*t3.*t8.*t9.*t11.*t35.*4.0-Lycm6.*Lz5.*dQ1.*dQ6.*m6.*t4.*t9.*t10.*t11.*t32.*2.0-Lycm6.*Lz5.*dQ2.*dQ6.*m6.*t2.*t8.*t10.*t11.*t34.*2.0-Lycm6.*Lz5.*dQ2.*dQ6.*m6.*t3.*t7.*t10.*t11.*t34.*2.0-Lycm6.*Lz5.*dQ2.*dQ6.*m6.*t6.*t7.*t8.*t9.*t35.*2.0;
et286 = Lycm6.*Lz5.*dQ1.*dQ6.*m6.*t4.*t9.*t10.*t11.*t33.*-2.0-Lycm6.*Lz5.*dQ3.*dQ6.*m6.*t2.*t8.*t10.*t11.*t34.*2.0-Lycm6.*Lz5.*dQ3.*dQ6.*m6.*t3.*t7.*t10.*t11.*t34.*2.0-Lycm6.*Lz5.*dQ3.*dQ6.*m6.*t6.*t7.*t8.*t9.*t35.*2.0-Lycm6.*Lz4.*dQ1.*dQ2.*m6.*t4.*t5.*t11.*t32.*t33.*8.0-Lycm6.*Lz4.*dQ1.*dQ3.*m6.*t4.*t5.*t11.*t32.*t33.*8.0-Lycm6.*Lz5.*dQ1.*dQ2.*m6.*t5.*t6.*t9.*t32.*t33.*8.0-Lycm6.*Lz5.*dQ1.*dQ3.*m6.*t5.*t6.*t9.*t32.*t33.*8.0-Lycm6.*Lz5.*dQ1.*dQ6.*m6.*t5.*t6.*t10.*t32.*t33.*4.0+Lycm6.*Lz5.*dQ1.*dQ6.*m6.*t5.*t6.*t10.*t32.*t34.*2.0+Lycm6.*Lz5.*dQ1.*dQ6.*m6.*t5.*t6.*t10.*t33.*t34.*2.0-Lycm6.*Lz5.*dQ1.*dQ2.*m6.*t4.*t11.*t32.*t33.*t35.*1.6e+1-Lycm6.*Lz5.*dQ1.*dQ3.*m6.*t4.*t11.*t32.*t33.*t35.*1.6e+1-Lycm6.*Lz5.*dQ1.*dQ4.*m6.*t6.*t10.*t32.*t33.*t34.*8.0;
et287 = Lycm6.*Lz5.*dQ1.*dQ5.*m6.*t11.*t32.*t33.*t34.*t35.*-8.0+Lycm4.*Lzcm4.*dQ1.*dQ2.*m4.*t2.*t3.*t7.*t8.*t9.*8.0+Lycm4.*Lzcm4.*dQ1.*dQ3.*m4.*t2.*t3.*t7.*t8.*t9.*8.0+Lycm6.*Lzcm6.*dQ1.*dQ4.*m6.*t2.*t4.*t5.*t6.*t7.*2.0+Lycm6.*Lzcm6.*dQ2.*dQ3.*m6.*t2.*t4.*t5.*t6.*t8.*2.0+Lycm6.*Lzcm6.*dQ2.*dQ3.*m6.*t3.*t4.*t5.*t6.*t7.*2.0+Lycm6.*Lzcm6.*dQ1.*dQ4.*m6.*t3.*t4.*t5.*t6.*t8.*2.0-Lycm5.*Lzcm5.*dQ1.*dQ2.*m5.*t2.*t4.*t7.*t9.*t10.*4.0-Lycm5.*Lzcm5.*dQ1.*dQ4.*m5.*t2.*t3.*t7.*t8.*t10.*4.0+Lycm6.*Lzcm6.*dQ2.*dQ5.*m6.*t2.*t3.*t4.*t6.*t10.*2.0-Lycm5.*Lzcm5.*dQ1.*dQ3.*m5.*t2.*t4.*t7.*t9.*t10.*4.0+Lycm6.*Lzcm6.*dQ3.*dQ5.*m6.*t2.*t3.*t4.*t6.*t10.*2.0-Lycm5.*Lzcm5.*dQ1.*dQ2.*m5.*t3.*t4.*t8.*t9.*t10.*4.0-Lycm5.*Lzcm5.*dQ1.*dQ3.*m5.*t3.*t4.*t8.*t9.*t10.*4.0-Lycm5.*Lzcm5.*dQ2.*dQ4.*m5.*t2.*t4.*t8.*t9.*t10.*4.0;
et288 = Lycm5.*Lzcm5.*dQ2.*dQ4.*m5.*t3.*t4.*t7.*t9.*t10.*-4.0-Lycm6.*Lzcm6.*dQ4.*dQ6.*m6.*t2.*t3.*t5.*t6.*t10.*2.0-Lycm5.*Lzcm5.*dQ3.*dQ4.*m5.*t2.*t4.*t8.*t9.*t10.*4.0-Lycm5.*Lzcm5.*dQ3.*dQ4.*m5.*t3.*t4.*t7.*t9.*t10.*4.0-Lycm6.*Lzcm6.*dQ1.*dQ5.*m6.*t2.*t3.*t7.*t8.*t11.*4.0-Lycm6.*Lzcm6.*dQ1.*dQ2.*m6.*t2.*t5.*t7.*t10.*t11.*4.0-Lycm6.*Lzcm6.*dQ1.*dQ3.*m6.*t2.*t5.*t7.*t10.*t11.*4.0-Lycm6.*Lzcm6.*dQ1.*dQ2.*m6.*t3.*t5.*t8.*t10.*t11.*4.0-Lycm6.*Lzcm6.*dQ1.*dQ5.*m6.*t2.*t6.*t7.*t9.*t10.*2.0-Lycm6.*Lzcm6.*dQ1.*dQ3.*m6.*t3.*t5.*t8.*t10.*t11.*4.0-Lycm6.*Lzcm6.*dQ1.*dQ6.*m6.*t2.*t5.*t7.*t9.*t11.*2.0-Lycm6.*Lzcm6.*dQ1.*dQ5.*m6.*t3.*t6.*t8.*t9.*t10.*2.0+Lycm6.*Lzcm6.*dQ2.*dQ4.*m6.*t2.*t5.*t8.*t10.*t11.*4.0+Lycm6.*Lzcm6.*dQ2.*dQ4.*m6.*t3.*t5.*t7.*t10.*t11.*4.0-Lycm6.*Lzcm6.*dQ2.*dQ5.*m6.*t4.*t6.*t7.*t8.*t10.*2.0;
et289 = Lycm6.*Lzcm6.*dQ1.*dQ6.*m6.*t3.*t5.*t8.*t9.*t11.*-2.0+Lycm6.*Lzcm6.*dQ3.*dQ4.*m6.*t2.*t5.*t8.*t10.*t11.*4.0+Lycm6.*Lzcm6.*dQ3.*dQ4.*m6.*t3.*t5.*t7.*t10.*t11.*4.0-Lycm6.*Lzcm6.*dQ3.*dQ5.*m6.*t4.*t6.*t7.*t8.*t10.*2.0+Lycm6.*Lzcm6.*dQ4.*dQ6.*m6.*t2.*t5.*t8.*t9.*t11.*2.0+Lycm6.*Lzcm6.*dQ4.*dQ6.*m6.*t3.*t5.*t7.*t9.*t11.*2.0+Lycm6.*Lzcm6.*dQ4.*dQ6.*m6.*t5.*t6.*t7.*t8.*t10.*2.0-Lycm5.*Lzcm5.*dQ1.*dQ4.*m5.*t2.*t4.*t5.*t7.*t33.*4.0-Lycm5.*Lzcm5.*dQ1.*dQ4.*m5.*t3.*t4.*t5.*t8.*t32.*4.0+Lycm6.*Lzcm6.*dQ1.*dQ6.*m6.*t2.*t4.*t6.*t7.*t33.*4.0+Lycm6.*Lzcm6.*dQ1.*dQ6.*m6.*t3.*t4.*t6.*t8.*t32.*4.0+Lycm6.*Lzcm6.*dQ2.*dQ3.*m6.*t2.*t3.*t6.*t10.*t34.*4.0+Lycm6.*Lzcm6.*dQ1.*dQ6.*m6.*t2.*t4.*t6.*t7.*t35.*4.0+Lycm6.*Lzcm6.*dQ1.*dQ5.*m6.*t4.*t5.*t6.*t9.*t32.*2.0+Lycm6.*Lzcm6.*dQ2.*dQ5.*m6.*t2.*t5.*t6.*t8.*t34.*2.0+Lycm6.*Lzcm6.*dQ2.*dQ5.*m6.*t3.*t5.*t6.*t7.*t34.*2.0;
et290 = Lycm6.*Lzcm6.*dQ1.*dQ5.*m6.*t4.*t5.*t6.*t9.*t33.*2.0+Lycm6.*Lzcm6.*dQ1.*dQ6.*m6.*t3.*t4.*t6.*t8.*t35.*4.0+Lycm6.*Lzcm6.*dQ2.*dQ6.*m6.*t2.*t3.*t6.*t9.*t35.*2.0+Lycm6.*Lzcm6.*dQ3.*dQ5.*m6.*t2.*t5.*t6.*t8.*t34.*2.0+Lycm6.*Lzcm6.*dQ3.*dQ5.*m6.*t3.*t5.*t6.*t7.*t34.*2.0+Lycm5.*Lzcm5.*dQ1.*dQ5.*m5.*t2.*t7.*t9.*t10.*t33.*4.0+Lycm6.*Lzcm6.*dQ3.*dQ6.*m6.*t2.*t3.*t6.*t9.*t35.*2.0+Lycm5.*Lzcm5.*dQ1.*dQ5.*m5.*t3.*t8.*t9.*t10.*t32.*4.0-Lycm6.*Lzcm6.*dQ4.*dQ6.*m6.*t2.*t4.*t6.*t8.*t35.*2.0-Lycm6.*Lzcm6.*dQ4.*dQ6.*m6.*t3.*t4.*t6.*t7.*t35.*2.0-Lycm6.*Lzcm6.*dQ1.*dQ4.*m6.*t2.*t7.*t9.*t11.*t33.*4.0-Lycm6.*Lzcm6.*dQ1.*dQ4.*m6.*t3.*t8.*t9.*t11.*t32.*4.0-Lycm6.*Lzcm6.*dQ1.*dQ4.*m6.*t2.*t7.*t9.*t11.*t35.*4.0-Lycm6.*Lzcm6.*dQ2.*dQ3.*m6.*t2.*t8.*t9.*t11.*t35.*4.0-Lycm6.*Lzcm6.*dQ2.*dQ3.*m6.*t3.*t7.*t9.*t11.*t35.*4.0-Lycm6.*Lzcm6.*dQ2.*dQ3.*m6.*t6.*t7.*t8.*t10.*t34.*4.0;
et291 = Lycm6.*Lzcm6.*dQ1.*dQ4.*m6.*t3.*t8.*t9.*t11.*t35.*-4.0-Lycm6.*Lzcm6.*dQ1.*dQ6.*m6.*t4.*t9.*t10.*t11.*t32.*2.0-Lycm6.*Lzcm6.*dQ2.*dQ6.*m6.*t2.*t8.*t10.*t11.*t34.*2.0-Lycm6.*Lzcm6.*dQ2.*dQ6.*m6.*t3.*t7.*t10.*t11.*t34.*2.0-Lycm6.*Lzcm6.*dQ2.*dQ6.*m6.*t6.*t7.*t8.*t9.*t35.*2.0-Lycm6.*Lzcm6.*dQ1.*dQ6.*m6.*t4.*t9.*t10.*t11.*t33.*2.0-Lycm6.*Lzcm6.*dQ3.*dQ6.*m6.*t2.*t8.*t10.*t11.*t34.*2.0-Lycm6.*Lzcm6.*dQ3.*dQ6.*m6.*t3.*t7.*t10.*t11.*t34.*2.0-Lycm6.*Lzcm6.*dQ3.*dQ6.*m6.*t6.*t7.*t8.*t9.*t35.*2.0-Lycm5.*Lzcm5.*dQ1.*dQ5.*m5.*t4.*t5.*t9.*t32.*t33.*4.0-Lycm6.*Lzcm6.*dQ1.*dQ2.*m6.*t5.*t6.*t9.*t32.*t33.*8.0-Lycm6.*Lzcm6.*dQ1.*dQ3.*m6.*t5.*t6.*t9.*t32.*t33.*8.0-Lycm6.*Lzcm6.*dQ1.*dQ6.*m6.*t5.*t6.*t10.*t32.*t33.*4.0+Lycm6.*Lzcm6.*dQ1.*dQ6.*m6.*t5.*t6.*t10.*t32.*t34.*2.0+Lycm6.*Lzcm6.*dQ1.*dQ6.*m6.*t5.*t6.*t10.*t33.*t34.*2.0;
et292 = Lycm6.*Lzcm6.*dQ1.*dQ2.*m6.*t4.*t11.*t32.*t33.*t35.*-1.6e+1-Lycm6.*Lzcm6.*dQ1.*dQ3.*m6.*t4.*t11.*t32.*t33.*t35.*1.6e+1-Lycm6.*Lzcm6.*dQ1.*dQ4.*m6.*t6.*t10.*t32.*t33.*t34.*8.0-Lycm6.*Lzcm6.*dQ1.*dQ5.*m6.*t11.*t32.*t33.*t34.*t35.*8.0-Lz4.*Lz5.*dQ1.*dQ5.*m6.*t2.*t3.*t7.*t8.*t10.*4.0+Lz4.*Lz5.*dQ1.*dQ5.*m6.*t2.*t4.*t5.*t7.*t33.*4.0+Lz4.*Lz5.*dQ1.*dQ5.*m6.*t3.*t4.*t5.*t8.*t32.*4.0-Lz4.*Lz5.*dQ1.*dQ4.*m6.*t2.*t7.*t9.*t10.*t33.*4.0-Lz4.*Lz5.*dQ1.*dQ4.*m6.*t3.*t8.*t9.*t10.*t32.*4.0-Lz4.*Lzcm5.*dQ1.*dQ5.*m5.*t2.*t3.*t7.*t8.*t10.*4.0-Lz4.*Lzcm6.*dQ1.*dQ5.*m6.*t2.*t3.*t7.*t8.*t10.*4.0+Lz5.*Lzcm6.*dQ1.*dQ4.*m6.*t2.*t5.*t7.*t9.*t10.*4.0+Lz5.*Lzcm6.*dQ2.*dQ3.*m6.*t2.*t5.*t8.*t9.*t10.*4.0+Lz5.*Lzcm6.*dQ2.*dQ3.*m6.*t3.*t5.*t7.*t9.*t10.*4.0+Lz5.*Lzcm6.*dQ1.*dQ4.*m6.*t3.*t5.*t8.*t9.*t10.*4.0;
et293 = Lz4.*Lzcm5.*dQ1.*dQ5.*m5.*t2.*t4.*t5.*t7.*t33.*4.0+Lz4.*Lzcm5.*dQ1.*dQ5.*m5.*t3.*t4.*t5.*t8.*t32.*4.0+Lz4.*Lzcm6.*dQ1.*dQ5.*m6.*t2.*t4.*t5.*t7.*t33.*4.0+Lz4.*Lzcm6.*dQ1.*dQ5.*m6.*t3.*t4.*t5.*t8.*t32.*4.0-Lz5.*Lzcm6.*dQ2.*dQ3.*m6.*t2.*t3.*t4.*t9.*t35.*4.0-Lz4.*Lzcm5.*dQ1.*dQ4.*m5.*t2.*t7.*t9.*t10.*t33.*4.0-Lz4.*Lzcm5.*dQ1.*dQ4.*m5.*t3.*t8.*t9.*t10.*t32.*4.0-Lz4.*Lzcm6.*dQ1.*dQ4.*m6.*t2.*t7.*t9.*t10.*t33.*4.0-Lz4.*Lzcm6.*dQ1.*dQ4.*m6.*t3.*t8.*t9.*t10.*t32.*4.0+Lz5.*Lzcm6.*dQ2.*dQ3.*m6.*t4.*t7.*t8.*t9.*t35.*4.0+Lz5.*Lzcm6.*dQ1.*dQ2.*m6.*t4.*t5.*t10.*t32.*t33.*1.6e+1+Lz5.*Lzcm6.*dQ1.*dQ5.*m6.*t2.*t4.*t7.*t33.*t35.*1.6e+1+Lz5.*Lzcm6.*dQ1.*dQ3.*m6.*t4.*t5.*t10.*t32.*t33.*1.6e+1+Lz5.*Lzcm6.*dQ1.*dQ5.*m6.*t3.*t4.*t8.*t32.*t35.*1.6e+1+Lz5.*Lzcm6.*dQ1.*dQ2.*m6.*t2.*t7.*t33.*t34.*t35.*8.0;
et294 = Lz5.*Lzcm6.*dQ1.*dQ2.*m6.*t3.*t8.*t32.*t34.*t35.*8.0+Lz5.*Lzcm6.*dQ1.*dQ3.*m6.*t2.*t7.*t33.*t34.*t35.*8.0+Lz5.*Lzcm6.*dQ1.*dQ3.*m6.*t3.*t8.*t32.*t34.*t35.*8.0+Lz5.*Lzcm6.*dQ1.*dQ4.*m6.*t4.*t9.*t32.*t33.*t35.*8.0+Lz5.*Lzcm6.*dQ1.*dQ5.*m6.*t5.*t10.*t32.*t33.*t34.*8.0-Ixx5.*dQ1.*dQ2.*t2.*t3.*t4.*t5.*t7.*t8.*t10.*8.0-Ixx5.*dQ1.*dQ3.*t2.*t3.*t4.*t5.*t7.*t8.*t10.*8.0+Ixx6.*dQ1.*dQ2.*t2.*t4.*t5.*t6.*t7.*t9.*t11.*4.0+Ixx6.*dQ1.*dQ3.*t2.*t4.*t5.*t6.*t7.*t9.*t11.*4.0+Ixx6.*dQ1.*dQ2.*t3.*t4.*t5.*t6.*t8.*t9.*t11.*4.0+Ixx6.*dQ1.*dQ3.*t3.*t4.*t5.*t6.*t8.*t9.*t11.*4.0+Ixx6.*dQ2.*dQ4.*t2.*t4.*t5.*t6.*t8.*t9.*t11.*4.0+Ixx6.*dQ2.*dQ4.*t3.*t4.*t5.*t6.*t7.*t9.*t11.*4.0+Ixx6.*dQ1.*dQ6.*t2.*t4.*t5.*t6.*t7.*t10.*t11.*4.0+Ixx6.*dQ3.*dQ4.*t2.*t4.*t5.*t6.*t8.*t9.*t11.*4.0;
et295 = Ixx6.*dQ3.*dQ4.*t3.*t4.*t5.*t6.*t7.*t9.*t11.*4.0+Ixx6.*dQ1.*dQ6.*t3.*t4.*t5.*t6.*t8.*t10.*t11.*4.0+Ixx6.*dQ2.*dQ6.*t2.*t3.*t5.*t6.*t9.*t10.*t11.*2.0+Ixx6.*dQ3.*dQ6.*t2.*t3.*t5.*t6.*t9.*t10.*t11.*2.0-Ixx6.*dQ2.*dQ6.*t5.*t6.*t7.*t8.*t9.*t10.*t11.*2.0-Ixx6.*dQ3.*dQ6.*t5.*t6.*t7.*t8.*t9.*t10.*t11.*2.0-Ixx5.*dQ1.*dQ5.*t2.*t3.*t5.*t7.*t8.*t10.*t34.*4.0-Ixx6.*dQ1.*dQ5.*t2.*t3.*t5.*t7.*t8.*t10.*t36.*4.0-Ixx6.*dQ1.*dQ4.*t2.*t4.*t6.*t7.*t10.*t11.*t33.*4.0-Ixx6.*dQ1.*dQ6.*t2.*t3.*t6.*t7.*t8.*t11.*t34.*4.0-Ixx6.*dQ1.*dQ4.*t3.*t4.*t6.*t8.*t10.*t11.*t32.*4.0-Ixx6.*dQ1.*dQ5.*t2.*t5.*t6.*t7.*t9.*t11.*t33.*4.0-Ixx6.*dQ1.*dQ6.*t2.*t3.*t6.*t7.*t8.*t11.*t35.*4.0-Ixx6.*dQ1.*dQ5.*t3.*t5.*t6.*t8.*t9.*t11.*t32.*4.0-Ixx6.*dQ1.*dQ4.*t2.*t5.*t7.*t9.*t10.*t33.*t36.*4.0;
et296 = Ixx6.*dQ1.*dQ4.*t3.*t5.*t8.*t9.*t10.*t32.*t36.*-4.0-Ixx6.*dQ1.*dQ5.*t4.*t6.*t9.*t10.*t11.*t32.*t33.*4.0+Ixy6.*dQ1.*dQ4.*t2.*t5.*t6.*t7.*t9.*t10.*t11.*2.0+Ixy6.*dQ2.*dQ3.*t2.*t5.*t6.*t8.*t9.*t10.*t11.*2.0+Ixy6.*dQ2.*dQ3.*t3.*t5.*t6.*t7.*t9.*t10.*t11.*2.0+Ixy6.*dQ1.*dQ4.*t3.*t5.*t6.*t8.*t9.*t10.*t11.*2.0-Ixy6.*dQ2.*dQ3.*t2.*t3.*t4.*t6.*t9.*t11.*t35.*2.0-Ixy6.*dQ1.*dQ2.*t2.*t3.*t7.*t8.*t9.*t10.*t36.*8.0-Ixy6.*dQ1.*dQ3.*t2.*t3.*t7.*t8.*t9.*t10.*t36.*8.0-Ixy6.*dQ1.*dQ6.*t2.*t6.*t7.*t9.*t10.*t11.*t33.*8.0+Ixy6.*dQ2.*dQ3.*t4.*t6.*t7.*t8.*t9.*t11.*t35.*2.0-Ixy6.*dQ1.*dQ6.*t3.*t6.*t8.*t9.*t10.*t11.*t32.*8.0+Ixy6.*dQ1.*dQ2.*t2.*t4.*t5.*t7.*t9.*t33.*t36.*8.0+Ixy6.*dQ1.*dQ2.*t3.*t4.*t5.*t8.*t9.*t32.*t36.*8.0+Ixy6.*dQ1.*dQ3.*t2.*t4.*t5.*t7.*t9.*t33.*t36.*8.0;
et297 = Ixy6.*dQ1.*dQ4.*t2.*t3.*t5.*t7.*t8.*t34.*t36.*8.0+Ixy6.*dQ1.*dQ3.*t3.*t4.*t5.*t8.*t9.*t32.*t36.*8.0+Ixy6.*dQ1.*dQ2.*t4.*t5.*t6.*t10.*t11.*t32.*t33.*8.0+Ixy6.*dQ1.*dQ5.*t2.*t4.*t6.*t7.*t11.*t33.*t35.*8.0+Ixy6.*dQ1.*dQ6.*t2.*t4.*t5.*t7.*t10.*t33.*t36.*8.0+Ixy6.*dQ1.*dQ3.*t4.*t5.*t6.*t10.*t11.*t32.*t33.*8.0+Ixy6.*dQ1.*dQ5.*t3.*t4.*t6.*t8.*t11.*t32.*t35.*8.0+Ixy6.*dQ1.*dQ6.*t3.*t4.*t5.*t8.*t10.*t32.*t36.*8.0+Ixy6.*dQ1.*dQ6.*t4.*t5.*t6.*t9.*t11.*t32.*t33.*8.0+Ixy6.*dQ1.*dQ2.*t2.*t6.*t7.*t11.*t33.*t34.*t35.*4.0+Ixy6.*dQ1.*dQ2.*t3.*t6.*t8.*t11.*t32.*t34.*t35.*4.0+Ixy6.*dQ1.*dQ3.*t2.*t6.*t7.*t11.*t33.*t34.*t35.*4.0+Ixy6.*dQ1.*dQ6.*t2.*t3.*t7.*t8.*t34.*t35.*t36.*4.0+Ixy6.*dQ1.*dQ3.*t3.*t6.*t8.*t11.*t32.*t34.*t35.*4.0+Ixy6.*dQ1.*dQ4.*t4.*t6.*t9.*t11.*t32.*t33.*t35.*4.0;
et298 = Ixy6.*dQ1.*dQ5.*t5.*t6.*t10.*t11.*t32.*t33.*t34.*4.0+Ixz6.*dQ2.*dQ3.*t2.*t3.*t4.*t5.*t6.*t9.*t10.*2.0+Ixz6.*dQ1.*dQ2.*t2.*t3.*t5.*t7.*t8.*t9.*t11.*4.0+Ixz6.*dQ1.*dQ3.*t2.*t3.*t5.*t7.*t8.*t9.*t11.*4.0+Ixz6.*dQ1.*dQ6.*t2.*t3.*t5.*t7.*t8.*t10.*t11.*2.0-Ixz6.*dQ2.*dQ3.*t4.*t5.*t6.*t7.*t8.*t9.*t10.*2.0-Ixz6.*dQ1.*dQ2.*t2.*t3.*t4.*t6.*t7.*t8.*t35.*8.0-Ixz6.*dQ1.*dQ3.*t2.*t3.*t4.*t6.*t7.*t8.*t35.*8.0-Ixz6.*dQ1.*dQ5.*t2.*t4.*t5.*t6.*t7.*t10.*t33.*8.0-Ixz6.*dQ1.*dQ5.*t3.*t4.*t5.*t6.*t8.*t10.*t32.*8.0+Ixz6.*dQ1.*dQ2.*t2.*t4.*t7.*t9.*t10.*t11.*t33.*4.0+Ixz6.*dQ1.*dQ2.*t3.*t4.*t8.*t9.*t10.*t11.*t32.*4.0+Ixz6.*dQ1.*dQ3.*t2.*t4.*t7.*t9.*t10.*t11.*t33.*4.0+Ixz6.*dQ1.*dQ4.*t2.*t3.*t7.*t8.*t10.*t11.*t34.*4.0+Ixz6.*dQ1.*dQ3.*t3.*t4.*t8.*t9.*t10.*t11.*t32.*4.0;
et299 = Ixz6.*dQ1.*dQ2.*t2.*t5.*t6.*t7.*t10.*t33.*t34.*-4.0-Ixz6.*dQ1.*dQ2.*t3.*t5.*t6.*t8.*t10.*t32.*t34.*4.0-Ixz6.*dQ1.*dQ3.*t2.*t5.*t6.*t7.*t10.*t33.*t34.*4.0-Ixz6.*dQ1.*dQ5.*t2.*t3.*t6.*t7.*t8.*t34.*t35.*4.0-Ixz6.*dQ1.*dQ3.*t3.*t5.*t6.*t8.*t10.*t32.*t34.*4.0-Ixz6.*dQ1.*dQ4.*t4.*t5.*t6.*t9.*t10.*t32.*t33.*4.0+Iyx6.*dQ1.*dQ4.*t2.*t5.*t6.*t7.*t9.*t10.*t11.*2.0+Iyx6.*dQ2.*dQ3.*t2.*t5.*t6.*t8.*t9.*t10.*t11.*2.0+Iyx6.*dQ2.*dQ3.*t3.*t5.*t6.*t7.*t9.*t10.*t11.*2.0+Iyx6.*dQ1.*dQ4.*t3.*t5.*t6.*t8.*t9.*t10.*t11.*2.0-Iyx6.*dQ2.*dQ3.*t2.*t3.*t4.*t6.*t9.*t11.*t35.*2.0-Iyx6.*dQ1.*dQ2.*t2.*t3.*t7.*t8.*t9.*t10.*t36.*8.0-Iyx6.*dQ1.*dQ3.*t2.*t3.*t7.*t8.*t9.*t10.*t36.*8.0-Iyx6.*dQ1.*dQ6.*t2.*t6.*t7.*t9.*t10.*t11.*t33.*8.0+Iyx6.*dQ2.*dQ3.*t4.*t6.*t7.*t8.*t9.*t11.*t35.*2.0;
et300 = Iyx6.*dQ1.*dQ6.*t3.*t6.*t8.*t9.*t10.*t11.*t32.*-8.0+Iyx6.*dQ1.*dQ2.*t2.*t4.*t5.*t7.*t9.*t33.*t36.*8.0+Iyx6.*dQ1.*dQ2.*t3.*t4.*t5.*t8.*t9.*t32.*t36.*8.0+Iyx6.*dQ1.*dQ3.*t2.*t4.*t5.*t7.*t9.*t33.*t36.*8.0+Iyx6.*dQ1.*dQ4.*t2.*t3.*t5.*t7.*t8.*t34.*t36.*8.0+Iyx6.*dQ1.*dQ3.*t3.*t4.*t5.*t8.*t9.*t32.*t36.*8.0+Iyx6.*dQ1.*dQ2.*t4.*t5.*t6.*t10.*t11.*t32.*t33.*8.0+Iyx6.*dQ1.*dQ5.*t2.*t4.*t6.*t7.*t11.*t33.*t35.*8.0+Iyx6.*dQ1.*dQ6.*t2.*t4.*t5.*t7.*t10.*t33.*t36.*8.0+Iyx6.*dQ1.*dQ3.*t4.*t5.*t6.*t10.*t11.*t32.*t33.*8.0+Iyx6.*dQ1.*dQ5.*t3.*t4.*t6.*t8.*t11.*t32.*t35.*8.0+Iyx6.*dQ1.*dQ6.*t3.*t4.*t5.*t8.*t10.*t32.*t36.*8.0+Iyx6.*dQ1.*dQ6.*t4.*t5.*t6.*t9.*t11.*t32.*t33.*8.0+Iyx6.*dQ1.*dQ2.*t2.*t6.*t7.*t11.*t33.*t34.*t35.*4.0+Iyx6.*dQ1.*dQ2.*t3.*t6.*t8.*t11.*t32.*t34.*t35.*4.0;
et301 = Iyx6.*dQ1.*dQ3.*t2.*t6.*t7.*t11.*t33.*t34.*t35.*4.0+Iyx6.*dQ1.*dQ6.*t2.*t3.*t7.*t8.*t34.*t35.*t36.*4.0+Iyx6.*dQ1.*dQ3.*t3.*t6.*t8.*t11.*t32.*t34.*t35.*4.0+Iyx6.*dQ1.*dQ4.*t4.*t6.*t9.*t11.*t32.*t33.*t35.*4.0+Iyx6.*dQ1.*dQ5.*t5.*t6.*t10.*t11.*t32.*t33.*t34.*4.0-Iyy6.*dQ1.*dQ2.*t2.*t3.*t4.*t5.*t7.*t8.*t10.*8.0-Iyy6.*dQ1.*dQ3.*t2.*t3.*t4.*t5.*t7.*t8.*t10.*8.0-Iyy6.*dQ1.*dQ2.*t2.*t4.*t5.*t6.*t7.*t9.*t11.*4.0-Iyy6.*dQ1.*dQ3.*t2.*t4.*t5.*t6.*t7.*t9.*t11.*4.0-Iyy6.*dQ1.*dQ2.*t3.*t4.*t5.*t6.*t8.*t9.*t11.*4.0-Iyy6.*dQ1.*dQ3.*t3.*t4.*t5.*t6.*t8.*t9.*t11.*4.0-Iyy6.*dQ2.*dQ4.*t2.*t4.*t5.*t6.*t8.*t9.*t11.*4.0-Iyy6.*dQ2.*dQ4.*t3.*t4.*t5.*t6.*t7.*t9.*t11.*4.0-Iyy6.*dQ1.*dQ6.*t2.*t4.*t5.*t6.*t7.*t10.*t11.*4.0-Iyy6.*dQ3.*dQ4.*t2.*t4.*t5.*t6.*t8.*t9.*t11.*4.0;
et302 = Iyy6.*dQ3.*dQ4.*t3.*t4.*t5.*t6.*t7.*t9.*t11.*-4.0-Iyy6.*dQ1.*dQ6.*t3.*t4.*t5.*t6.*t8.*t10.*t11.*4.0-Iyy6.*dQ2.*dQ6.*t2.*t3.*t5.*t6.*t9.*t10.*t11.*2.0-Iyy6.*dQ3.*dQ6.*t2.*t3.*t5.*t6.*t9.*t10.*t11.*2.0+Iyy6.*dQ2.*dQ6.*t5.*t6.*t7.*t8.*t9.*t10.*t11.*2.0+Iyy6.*dQ3.*dQ6.*t5.*t6.*t7.*t8.*t9.*t10.*t11.*2.0-Iyy6.*dQ1.*dQ5.*t2.*t3.*t5.*t7.*t8.*t10.*t34.*4.0+Iyy6.*dQ1.*dQ5.*t2.*t3.*t5.*t7.*t8.*t10.*t36.*4.0+Iyy6.*dQ1.*dQ4.*t2.*t4.*t6.*t7.*t10.*t11.*t33.*4.0+Iyy6.*dQ1.*dQ6.*t2.*t3.*t6.*t7.*t8.*t11.*t34.*4.0+Iyy6.*dQ1.*dQ4.*t3.*t4.*t6.*t8.*t10.*t11.*t32.*4.0+Iyy6.*dQ1.*dQ5.*t2.*t5.*t6.*t7.*t9.*t11.*t33.*4.0+Iyy6.*dQ1.*dQ6.*t2.*t3.*t6.*t7.*t8.*t11.*t35.*4.0+Iyy6.*dQ1.*dQ5.*t3.*t5.*t6.*t8.*t9.*t11.*t32.*4.0-Iyy6.*dQ2.*dQ5.*t2.*t4.*t5.*t8.*t9.*t10.*t36.*2.0-Iyy6.*dQ2.*dQ5.*t3.*t4.*t5.*t7.*t9.*t10.*t36.*2.0;
et303 = Iyy6.*dQ3.*dQ5.*t2.*t4.*t5.*t8.*t9.*t10.*t36.*-2.0-Iyy6.*dQ3.*dQ5.*t3.*t4.*t5.*t7.*t9.*t10.*t36.*2.0-Iyy6.*dQ2.*dQ6.*t2.*t4.*t6.*t8.*t9.*t11.*t35.*2.0-Iyy6.*dQ2.*dQ6.*t3.*t4.*t6.*t7.*t9.*t11.*t35.*2.0-Iyy6.*dQ3.*dQ6.*t2.*t4.*t6.*t8.*t9.*t11.*t35.*2.0-Iyy6.*dQ3.*dQ6.*t3.*t4.*t6.*t7.*t9.*t11.*t35.*2.0+Iyy6.*dQ1.*dQ4.*t2.*t5.*t7.*t9.*t10.*t33.*t36.*4.0+Iyy6.*dQ1.*dQ4.*t3.*t5.*t8.*t9.*t10.*t32.*t36.*4.0+Iyy6.*dQ1.*dQ5.*t4.*t6.*t9.*t10.*t11.*t32.*t33.*4.0+Iyz6.*dQ1.*dQ2.*t2.*t3.*t5.*t6.*t7.*t8.*t9.*4.0+Iyz6.*dQ1.*dQ3.*t2.*t3.*t5.*t6.*t7.*t8.*t9.*4.0+Iyz6.*dQ1.*dQ6.*t2.*t3.*t5.*t6.*t7.*t8.*t10.*2.0-Iyz6.*dQ2.*dQ3.*t2.*t3.*t4.*t5.*t9.*t10.*t11.*2.0+Iyz6.*dQ2.*dQ3.*t4.*t5.*t7.*t8.*t9.*t10.*t11.*2.0+Iyz6.*dQ1.*dQ2.*t2.*t3.*t4.*t7.*t8.*t11.*t35.*8.0+Iyz6.*dQ1.*dQ2.*t2.*t4.*t6.*t7.*t9.*t10.*t33.*4.0;
et304 = Iyz6.*dQ1.*dQ3.*t2.*t3.*t4.*t7.*t8.*t11.*t35.*8.0+Iyz6.*dQ1.*dQ2.*t3.*t4.*t6.*t8.*t9.*t10.*t32.*4.0+Iyz6.*dQ1.*dQ3.*t2.*t4.*t6.*t7.*t9.*t10.*t33.*4.0+Iyz6.*dQ1.*dQ4.*t2.*t3.*t6.*t7.*t8.*t10.*t34.*4.0+Iyz6.*dQ1.*dQ3.*t3.*t4.*t6.*t8.*t9.*t10.*t32.*4.0+Iyz6.*dQ1.*dQ5.*t2.*t4.*t5.*t7.*t10.*t11.*t33.*8.0+Iyz6.*dQ1.*dQ5.*t3.*t4.*t5.*t8.*t10.*t11.*t32.*8.0+Iyz6.*dQ1.*dQ2.*t2.*t5.*t7.*t10.*t11.*t33.*t34.*4.0+Iyz6.*dQ1.*dQ2.*t3.*t5.*t8.*t10.*t11.*t32.*t34.*4.0+Iyz6.*dQ1.*dQ3.*t2.*t5.*t7.*t10.*t11.*t33.*t34.*4.0+Iyz6.*dQ1.*dQ5.*t2.*t3.*t7.*t8.*t11.*t34.*t35.*4.0+Iyz6.*dQ1.*dQ3.*t3.*t5.*t8.*t10.*t11.*t32.*t34.*4.0+Iyz6.*dQ1.*dQ4.*t4.*t5.*t9.*t10.*t11.*t32.*t33.*4.0+Izx6.*dQ2.*dQ3.*t2.*t3.*t4.*t5.*t6.*t9.*t10.*2.0+Izx6.*dQ1.*dQ2.*t2.*t3.*t5.*t7.*t8.*t9.*t11.*4.0+Izx6.*dQ1.*dQ3.*t2.*t3.*t5.*t7.*t8.*t9.*t11.*4.0;
et305 = Izx6.*dQ1.*dQ6.*t2.*t3.*t5.*t7.*t8.*t10.*t11.*2.0-Izx6.*dQ2.*dQ3.*t4.*t5.*t6.*t7.*t8.*t9.*t10.*2.0-Izx6.*dQ1.*dQ2.*t2.*t3.*t4.*t6.*t7.*t8.*t35.*8.0-Izx6.*dQ1.*dQ3.*t2.*t3.*t4.*t6.*t7.*t8.*t35.*8.0-Izx6.*dQ1.*dQ5.*t2.*t4.*t5.*t6.*t7.*t10.*t33.*8.0-Izx6.*dQ1.*dQ5.*t3.*t4.*t5.*t6.*t8.*t10.*t32.*8.0+Izx6.*dQ1.*dQ2.*t2.*t4.*t7.*t9.*t10.*t11.*t33.*4.0+Izx6.*dQ1.*dQ2.*t3.*t4.*t8.*t9.*t10.*t11.*t32.*4.0+Izx6.*dQ1.*dQ3.*t2.*t4.*t7.*t9.*t10.*t11.*t33.*4.0+Izx6.*dQ1.*dQ4.*t2.*t3.*t7.*t8.*t10.*t11.*t34.*4.0+Izx6.*dQ1.*dQ3.*t3.*t4.*t8.*t9.*t10.*t11.*t32.*4.0-Izx6.*dQ1.*dQ2.*t2.*t5.*t6.*t7.*t10.*t33.*t34.*4.0-Izx6.*dQ1.*dQ2.*t3.*t5.*t6.*t8.*t10.*t32.*t34.*4.0-Izx6.*dQ1.*dQ3.*t2.*t5.*t6.*t7.*t10.*t33.*t34.*4.0-Izx6.*dQ1.*dQ5.*t2.*t3.*t6.*t7.*t8.*t34.*t35.*4.0;
et306 = Izx6.*dQ1.*dQ3.*t3.*t5.*t6.*t8.*t10.*t32.*t34.*-4.0-Izx6.*dQ1.*dQ4.*t4.*t5.*t6.*t9.*t10.*t32.*t33.*4.0+Izy6.*dQ1.*dQ2.*t2.*t3.*t5.*t6.*t7.*t8.*t9.*4.0+Izy6.*dQ1.*dQ3.*t2.*t3.*t5.*t6.*t7.*t8.*t9.*4.0+Izy6.*dQ1.*dQ6.*t2.*t3.*t5.*t6.*t7.*t8.*t10.*2.0-Izy6.*dQ2.*dQ3.*t2.*t3.*t4.*t5.*t9.*t10.*t11.*2.0+Izy6.*dQ2.*dQ3.*t4.*t5.*t7.*t8.*t9.*t10.*t11.*2.0+Izy6.*dQ1.*dQ2.*t2.*t3.*t4.*t7.*t8.*t11.*t35.*8.0+Izy6.*dQ1.*dQ2.*t2.*t4.*t6.*t7.*t9.*t10.*t33.*4.0+Izy6.*dQ1.*dQ3.*t2.*t3.*t4.*t7.*t8.*t11.*t35.*8.0+Izy6.*dQ1.*dQ2.*t3.*t4.*t6.*t8.*t9.*t10.*t32.*4.0+Izy6.*dQ1.*dQ3.*t2.*t4.*t6.*t7.*t9.*t10.*t33.*4.0+Izy6.*dQ1.*dQ4.*t2.*t3.*t6.*t7.*t8.*t10.*t34.*4.0+Izy6.*dQ1.*dQ3.*t3.*t4.*t6.*t8.*t9.*t10.*t32.*4.0+Izy6.*dQ1.*dQ5.*t2.*t4.*t5.*t7.*t10.*t11.*t33.*8.0+Izy6.*dQ1.*dQ5.*t3.*t4.*t5.*t8.*t10.*t11.*t32.*8.0;
et307 = Izy6.*dQ1.*dQ2.*t2.*t5.*t7.*t10.*t11.*t33.*t34.*4.0+Izy6.*dQ1.*dQ2.*t3.*t5.*t8.*t10.*t11.*t32.*t34.*4.0+Izy6.*dQ1.*dQ3.*t2.*t5.*t7.*t10.*t11.*t33.*t34.*4.0+Izy6.*dQ1.*dQ5.*t2.*t3.*t7.*t8.*t11.*t34.*t35.*4.0+Izy6.*dQ1.*dQ3.*t3.*t5.*t8.*t10.*t11.*t32.*t34.*4.0+Izy6.*dQ1.*dQ4.*t4.*t5.*t9.*t10.*t11.*t32.*t33.*4.0+Izz5.*dQ1.*dQ2.*t2.*t3.*t4.*t5.*t7.*t8.*t10.*8.0+Izz5.*dQ1.*dQ3.*t2.*t3.*t4.*t5.*t7.*t8.*t10.*8.0+Izz6.*dQ1.*dQ2.*t2.*t3.*t4.*t5.*t7.*t8.*t10.*8.0+Izz6.*dQ1.*dQ3.*t2.*t3.*t4.*t5.*t7.*t8.*t10.*8.0+Izz5.*dQ1.*dQ5.*t2.*t3.*t5.*t7.*t8.*t10.*t34.*4.0+Izz6.*dQ1.*dQ5.*t2.*t3.*t5.*t7.*t8.*t10.*t34.*4.0+dQ1.*dQ4.*m4.*t2.*t3.*t4.*t7.*t8.*t9.*t15.*4.0-dQ1.*dQ4.*m4.*t2.*t3.*t4.*t7.*t8.*t9.*t18.*4.0-dQ1.*dQ4.*m6.*t2.*t3.*t4.*t7.*t8.*t9.*t17.*4.0+dQ2.*dQ5.*m6.*t2.*t3.*t4.*t5.*t6.*t11.*t17.*2.0;
et308 = dQ1.*dQ4.*m5.*t2.*t3.*t4.*t7.*t8.*t9.*t19.*-4.0+dQ1.*dQ5.*m5.*t2.*t3.*t5.*t7.*t8.*t10.*t16.*4.0+dQ3.*dQ5.*m6.*t2.*t3.*t4.*t5.*t6.*t11.*t17.*2.0-dQ2.*dQ5.*m6.*t2.*t3.*t4.*t5.*t6.*t11.*t20.*2.0-dQ3.*dQ5.*m6.*t2.*t3.*t4.*t5.*t6.*t11.*t20.*2.0+dQ1.*dQ4.*m6.*t2.*t3.*t4.*t7.*t8.*t9.*t22.*4.0-dQ2.*dQ5.*m5.*t2.*t4.*t5.*t8.*t9.*t10.*t16.*2.0-dQ2.*dQ5.*m5.*t3.*t4.*t5.*t7.*t9.*t10.*t16.*2.0+dQ1.*dQ5.*m6.*t2.*t3.*t5.*t7.*t8.*t10.*t20.*4.0-dQ1.*dQ6.*m6.*t2.*t3.*t6.*t7.*t8.*t11.*t17.*8.0-dQ3.*dQ5.*m5.*t2.*t4.*t5.*t8.*t9.*t10.*t16.*2.0-dQ3.*dQ5.*m5.*t3.*t4.*t5.*t7.*t9.*t10.*t16.*2.0+dQ1.*dQ4.*m5.*t2.*t3.*t4.*t7.*t8.*t9.*t25.*4.0-dQ1.*dQ4.*m6.*t2.*t4.*t6.*t7.*t10.*t11.*t17.*2.0-dQ1.*dQ5.*m6.*t2.*t3.*t5.*t7.*t8.*t10.*t22.*4.0;
et309 = dQ1.*dQ5.*m6.*t2.*t5.*t6.*t7.*t9.*t11.*t17.*-2.0-dQ2.*dQ3.*m6.*t2.*t4.*t6.*t8.*t10.*t11.*t17.*2.0-dQ2.*dQ3.*m6.*t3.*t4.*t6.*t7.*t10.*t11.*t17.*2.0+dQ1.*dQ4.*m6.*t2.*t3.*t4.*t7.*t8.*t9.*t26.*4.0-dQ1.*dQ4.*m6.*t3.*t4.*t6.*t8.*t10.*t11.*t17.*2.0+dQ1.*dQ6.*m6.*t2.*t3.*t6.*t7.*t8.*t11.*t20.*8.0+dQ1.*dQ4.*m6.*t2.*t4.*t6.*t7.*t10.*t11.*t20.*2.0-dQ1.*dQ5.*m5.*t2.*t3.*t5.*t7.*t8.*t10.*t25.*4.0-dQ1.*dQ5.*m6.*t3.*t5.*t6.*t8.*t9.*t11.*t17.*2.0-dQ2.*dQ5.*m6.*t2.*t4.*t5.*t8.*t9.*t10.*t20.*2.0-dQ2.*dQ5.*m6.*t3.*t4.*t5.*t7.*t9.*t10.*t20.*2.0-dQ2.*dQ5.*m6.*t4.*t5.*t6.*t7.*t8.*t11.*t17.*2.0-dQ2.*dQ6.*m6.*t2.*t4.*t6.*t8.*t9.*t11.*t17.*2.0-dQ2.*dQ6.*m6.*t3.*t4.*t6.*t7.*t9.*t11.*t17.*2.0+dQ1.*dQ5.*m6.*t2.*t5.*t6.*t7.*t9.*t11.*t20.*2.0;
et310 = dQ2.*dQ3.*m6.*t2.*t4.*t6.*t8.*t10.*t11.*t20.*2.0+dQ2.*dQ3.*m6.*t3.*t4.*t6.*t7.*t10.*t11.*t20.*2.0-dQ3.*dQ5.*m6.*t2.*t4.*t5.*t8.*t9.*t10.*t20.*2.0-dQ3.*dQ5.*m6.*t3.*t4.*t5.*t7.*t9.*t10.*t20.*2.0-dQ3.*dQ5.*m6.*t4.*t5.*t6.*t7.*t8.*t11.*t17.*2.0-dQ3.*dQ6.*m6.*t2.*t4.*t6.*t8.*t9.*t11.*t17.*2.0-dQ3.*dQ6.*m6.*t3.*t4.*t6.*t7.*t9.*t11.*t17.*2.0+dQ1.*dQ4.*m6.*t3.*t4.*t6.*t8.*t10.*t11.*t20.*2.0-dQ1.*dQ5.*m6.*t2.*t3.*t5.*t7.*t8.*t10.*t26.*4.0+dQ2.*dQ5.*m6.*t2.*t4.*t5.*t8.*t9.*t10.*t22.*2.0+dQ2.*dQ5.*m6.*t3.*t4.*t5.*t7.*t9.*t10.*t22.*2.0+dQ1.*dQ5.*m6.*t3.*t5.*t6.*t8.*t9.*t11.*t20.*2.0+dQ2.*dQ5.*m6.*t4.*t5.*t6.*t7.*t8.*t11.*t20.*2.0+dQ2.*dQ6.*m6.*t2.*t4.*t6.*t8.*t9.*t11.*t20.*2.0+dQ2.*dQ6.*m6.*t3.*t4.*t6.*t7.*t9.*t11.*t20.*2.0+dQ3.*dQ5.*m6.*t2.*t4.*t5.*t8.*t9.*t10.*t22.*2.0;
et311 = dQ3.*dQ5.*m6.*t3.*t4.*t5.*t7.*t9.*t10.*t22.*2.0+dQ2.*dQ5.*m5.*t2.*t4.*t5.*t8.*t9.*t10.*t25.*2.0+dQ2.*dQ5.*m5.*t3.*t4.*t5.*t7.*t9.*t10.*t25.*2.0+dQ3.*dQ5.*m6.*t4.*t5.*t6.*t7.*t8.*t11.*t20.*2.0+dQ3.*dQ6.*m6.*t2.*t4.*t6.*t8.*t9.*t11.*t20.*2.0+dQ3.*dQ6.*m6.*t3.*t4.*t6.*t7.*t9.*t11.*t20.*2.0+dQ3.*dQ5.*m5.*t2.*t4.*t5.*t8.*t9.*t10.*t25.*2.0+dQ3.*dQ5.*m5.*t3.*t4.*t5.*t7.*t9.*t10.*t25.*2.0+dQ2.*dQ5.*m6.*t2.*t4.*t5.*t8.*t9.*t10.*t26.*2.0+dQ2.*dQ5.*m6.*t3.*t4.*t5.*t7.*t9.*t10.*t26.*2.0+dQ3.*dQ5.*m6.*t2.*t4.*t5.*t8.*t9.*t10.*t26.*2.0+dQ3.*dQ5.*m6.*t3.*t4.*t5.*t7.*t9.*t10.*t26.*2.0+dQ2.*dQ3.*m6.*t2.*t3.*t5.*t6.*t11.*t17.*t34.*4.0+dQ1.*dQ4.*m5.*t2.*t5.*t7.*t9.*t10.*t16.*t33.*4.0-dQ2.*dQ3.*m6.*t2.*t3.*t5.*t6.*t11.*t20.*t34.*4.0+dQ1.*dQ4.*m5.*t3.*t5.*t8.*t9.*t10.*t16.*t32.*4.0;
et312 = dQ1.*dQ4.*m6.*t2.*t5.*t7.*t9.*t10.*t17.*t36.*-2.0+dQ1.*dQ4.*m6.*t2.*t5.*t7.*t9.*t10.*t20.*t33.*4.0+dQ1.*dQ4.*m6.*t3.*t5.*t8.*t9.*t10.*t20.*t32.*4.0-dQ2.*dQ3.*m6.*t2.*t5.*t8.*t9.*t10.*t17.*t36.*2.0-dQ2.*dQ3.*m6.*t3.*t5.*t7.*t9.*t10.*t17.*t36.*2.0-dQ1.*dQ4.*m6.*t2.*t5.*t7.*t9.*t10.*t22.*t33.*4.0-dQ1.*dQ4.*m6.*t3.*t5.*t8.*t9.*t10.*t17.*t36.*2.0-dQ2.*dQ3.*m6.*t5.*t6.*t7.*t8.*t11.*t17.*t34.*4.0+dQ1.*dQ4.*m6.*t2.*t5.*t7.*t9.*t10.*t20.*t36.*2.0-dQ1.*dQ4.*m6.*t3.*t5.*t8.*t9.*t10.*t22.*t32.*4.0-dQ1.*dQ4.*m5.*t2.*t5.*t7.*t9.*t10.*t25.*t33.*4.0-dQ1.*dQ5.*m6.*t4.*t6.*t9.*t10.*t11.*t17.*t32.*2.0+dQ2.*dQ3.*m6.*t2.*t5.*t8.*t9.*t10.*t20.*t36.*2.0+dQ2.*dQ3.*m6.*t3.*t5.*t7.*t9.*t10.*t20.*t36.*2.0-dQ2.*dQ5.*m6.*t2.*t6.*t8.*t10.*t11.*t17.*t34.*2.0;
et313 = dQ2.*dQ5.*m6.*t3.*t6.*t7.*t10.*t11.*t17.*t34.*-2.0-dQ1.*dQ4.*m5.*t3.*t5.*t8.*t9.*t10.*t25.*t32.*4.0+dQ1.*dQ4.*m6.*t3.*t5.*t8.*t9.*t10.*t20.*t36.*2.0-dQ1.*dQ5.*m6.*t4.*t6.*t9.*t10.*t11.*t17.*t33.*2.0+dQ2.*dQ3.*m6.*t5.*t6.*t7.*t8.*t11.*t20.*t34.*4.0-dQ3.*dQ5.*m6.*t2.*t6.*t8.*t10.*t11.*t17.*t34.*2.0-dQ3.*dQ5.*m6.*t3.*t6.*t7.*t10.*t11.*t17.*t34.*2.0-dQ1.*dQ4.*m6.*t2.*t5.*t7.*t9.*t10.*t26.*t33.*4.0-dQ1.*dQ4.*m6.*t3.*t5.*t8.*t9.*t10.*t26.*t32.*4.0+dQ1.*dQ5.*m6.*t4.*t6.*t9.*t10.*t11.*t20.*t32.*2.0+dQ2.*dQ5.*m6.*t2.*t6.*t8.*t10.*t11.*t20.*t34.*2.0+dQ2.*dQ5.*m6.*t3.*t6.*t7.*t10.*t11.*t20.*t34.*2.0+dQ1.*dQ5.*m6.*t4.*t6.*t9.*t10.*t11.*t20.*t33.*2.0+dQ3.*dQ5.*m6.*t2.*t6.*t8.*t10.*t11.*t20.*t34.*2.0+dQ3.*dQ5.*m6.*t3.*t6.*t7.*t10.*t11.*t20.*t34.*2.0+dQ2.*dQ3.*m6.*t2.*t3.*t4.*t9.*t17.*t35.*t36.*2.0;
et314 = dQ2.*dQ3.*m6.*t2.*t3.*t4.*t9.*t20.*t35.*t36.*-2.0+dQ1.*dQ2.*m6.*t6.*t9.*t10.*t11.*t17.*t32.*t33.*8.0+dQ1.*dQ6.*m6.*t2.*t7.*t9.*t10.*t17.*t33.*t36.*8.0-dQ2.*dQ3.*m6.*t4.*t7.*t8.*t9.*t17.*t35.*t36.*2.0+dQ1.*dQ3.*m6.*t6.*t9.*t10.*t11.*t17.*t32.*t33.*8.0+dQ1.*dQ6.*m6.*t3.*t8.*t9.*t10.*t17.*t32.*t36.*8.0-dQ1.*dQ2.*m6.*t6.*t9.*t10.*t11.*t20.*t32.*t33.*8.0-dQ1.*dQ6.*m6.*t2.*t7.*t9.*t10.*t20.*t33.*t36.*8.0+dQ2.*dQ3.*m6.*t4.*t7.*t8.*t9.*t20.*t35.*t36.*2.0-dQ1.*dQ3.*m6.*t6.*t9.*t10.*t11.*t20.*t32.*t33.*8.0-dQ1.*dQ6.*m6.*t3.*t8.*t9.*t10.*t20.*t32.*t36.*8.0-dQ1.*dQ2.*m6.*t4.*t5.*t10.*t17.*t32.*t33.*t36.*8.0-dQ1.*dQ5.*m6.*t2.*t4.*t7.*t17.*t33.*t35.*t36.*8.0-dQ1.*dQ3.*m6.*t4.*t5.*t10.*t17.*t32.*t33.*t36.*8.0;
et315 = dQ1.*dQ5.*m6.*t3.*t4.*t8.*t17.*t32.*t35.*t36.*-8.0+dQ1.*dQ2.*m6.*t4.*t5.*t10.*t20.*t32.*t33.*t36.*8.0-dQ1.*dQ4.*m6.*t5.*t6.*t11.*t17.*t32.*t33.*t34.*8.0+dQ1.*dQ5.*m6.*t2.*t4.*t7.*t20.*t33.*t35.*t36.*8.0-dQ1.*dQ6.*m6.*t4.*t5.*t9.*t17.*t32.*t33.*t36.*8.0+dQ1.*dQ3.*m6.*t4.*t5.*t10.*t20.*t32.*t33.*t36.*8.0+dQ1.*dQ5.*m6.*t3.*t4.*t8.*t20.*t32.*t35.*t36.*8.0+dQ1.*dQ4.*m6.*t5.*t6.*t11.*t20.*t32.*t33.*t34.*8.0+dQ1.*dQ6.*m6.*t4.*t5.*t9.*t20.*t32.*t33.*t36.*8.0-dQ1.*dQ2.*m6.*t2.*t7.*t17.*t33.*t34.*t35.*t36.*4.0-dQ1.*dQ2.*m6.*t3.*t8.*t17.*t32.*t34.*t35.*t36.*4.0-dQ1.*dQ3.*m6.*t2.*t7.*t17.*t33.*t34.*t35.*t36.*4.0-dQ1.*dQ3.*m6.*t3.*t8.*t17.*t32.*t34.*t35.*t36.*4.0+dQ1.*dQ2.*m6.*t2.*t7.*t20.*t33.*t34.*t35.*t36.*4.0+dQ1.*dQ2.*m6.*t3.*t8.*t20.*t32.*t34.*t35.*t36.*4.0;
et316 = dQ1.*dQ3.*m6.*t2.*t7.*t20.*t33.*t34.*t35.*t36.*4.0-dQ1.*dQ4.*m6.*t4.*t9.*t17.*t32.*t33.*t35.*t36.*4.0+dQ1.*dQ3.*m6.*t3.*t8.*t20.*t32.*t34.*t35.*t36.*4.0-dQ1.*dQ5.*m6.*t5.*t10.*t17.*t32.*t33.*t34.*t36.*4.0+dQ1.*dQ4.*m6.*t4.*t9.*t20.*t32.*t33.*t35.*t36.*4.0-dQ1.*dQ6.*m6.*t6.*t11.*t17.*t32.*t33.*t34.*t35.*4.0+dQ1.*dQ5.*m6.*t5.*t10.*t20.*t32.*t33.*t34.*t36.*4.0+dQ1.*dQ6.*m6.*t6.*t11.*t20.*t32.*t33.*t34.*t35.*4.0+Ixx6.*dQ1.*dQ2.*t2.*t3.*t6.*t7.*t8.*t9.*t10.*t11.*8.0+Ixx6.*dQ1.*dQ3.*t2.*t3.*t6.*t7.*t8.*t9.*t10.*t11.*8.0-Ixx6.*dQ1.*dQ2.*t2.*t3.*t4.*t5.*t7.*t8.*t10.*t36.*8.0-Ixx6.*dQ1.*dQ3.*t2.*t3.*t4.*t5.*t7.*t8.*t10.*t36.*8.0-Ixx6.*dQ1.*dQ2.*t2.*t4.*t5.*t6.*t7.*t9.*t11.*t33.*8.0-Ixx6.*dQ1.*dQ2.*t3.*t4.*t5.*t6.*t8.*t9.*t11.*t32.*8.0;
et317 = Ixx6.*dQ1.*dQ3.*t2.*t4.*t5.*t6.*t7.*t9.*t11.*t33.*-8.0-Ixx6.*dQ1.*dQ3.*t3.*t4.*t5.*t6.*t8.*t9.*t11.*t32.*8.0-Ixx6.*dQ1.*dQ6.*t2.*t4.*t5.*t6.*t7.*t10.*t11.*t33.*8.0-Ixx6.*dQ1.*dQ6.*t3.*t4.*t5.*t6.*t8.*t10.*t11.*t32.*8.0-Ixx6.*dQ1.*dQ5.*t2.*t3.*t5.*t7.*t8.*t10.*t34.*t36.*4.0-Ixx6.*dQ1.*dQ6.*t2.*t3.*t6.*t7.*t8.*t11.*t34.*t35.*4.0-Ixy6.*dQ1.*dQ4.*t2.*t3.*t4.*t6.*t7.*t8.*t9.*t11.*4.0-Ixy6.*dQ1.*dQ4.*t2.*t5.*t6.*t7.*t9.*t10.*t11.*t33.*4.0-Ixy6.*dQ1.*dQ4.*t3.*t5.*t6.*t8.*t9.*t10.*t11.*t32.*4.0+Ixz6.*dQ1.*dQ6.*t2.*t3.*t4.*t6.*t7.*t8.*t9.*t10.*2.0+Ixz6.*dQ1.*dQ6.*t2.*t3.*t5.*t7.*t8.*t10.*t11.*t34.*2.0-Iyx6.*dQ1.*dQ4.*t2.*t3.*t4.*t6.*t7.*t8.*t9.*t11.*4.0-Iyx6.*dQ1.*dQ4.*t2.*t5.*t6.*t7.*t9.*t10.*t11.*t33.*4.0-Iyx6.*dQ1.*dQ4.*t3.*t5.*t6.*t8.*t9.*t10.*t11.*t32.*4.0;
et318 = Iyy6.*dQ1.*dQ2.*t2.*t3.*t6.*t7.*t8.*t9.*t10.*t11.*-8.0-Iyy6.*dQ1.*dQ3.*t2.*t3.*t6.*t7.*t8.*t9.*t10.*t11.*8.0+Iyy6.*dQ1.*dQ2.*t2.*t3.*t4.*t5.*t7.*t8.*t10.*t36.*8.0+Iyy6.*dQ1.*dQ3.*t2.*t3.*t4.*t5.*t7.*t8.*t10.*t36.*8.0+Iyy6.*dQ1.*dQ2.*t2.*t4.*t5.*t6.*t7.*t9.*t11.*t33.*8.0+Iyy6.*dQ1.*dQ2.*t3.*t4.*t5.*t6.*t8.*t9.*t11.*t32.*8.0+Iyy6.*dQ1.*dQ3.*t2.*t4.*t5.*t6.*t7.*t9.*t11.*t33.*8.0+Iyy6.*dQ1.*dQ3.*t3.*t4.*t5.*t6.*t8.*t9.*t11.*t32.*8.0+Iyy6.*dQ1.*dQ6.*t2.*t4.*t5.*t6.*t7.*t10.*t11.*t33.*8.0+Iyy6.*dQ1.*dQ6.*t3.*t4.*t5.*t6.*t8.*t10.*t11.*t32.*8.0+Iyy6.*dQ1.*dQ5.*t2.*t3.*t5.*t7.*t8.*t10.*t34.*t36.*4.0+Iyy6.*dQ1.*dQ6.*t2.*t3.*t6.*t7.*t8.*t11.*t34.*t35.*4.0-Iyz6.*dQ1.*dQ6.*t2.*t3.*t4.*t7.*t8.*t9.*t10.*t11.*2.0+Iyz6.*dQ1.*dQ6.*t2.*t3.*t5.*t6.*t7.*t8.*t10.*t34.*2.0;
et319 = Izx6.*dQ1.*dQ6.*t2.*t3.*t4.*t6.*t7.*t8.*t9.*t10.*2.0+Izx6.*dQ1.*dQ6.*t2.*t3.*t5.*t7.*t8.*t10.*t11.*t34.*2.0-Izy6.*dQ1.*dQ6.*t2.*t3.*t4.*t7.*t8.*t9.*t10.*t11.*2.0+Izy6.*dQ1.*dQ6.*t2.*t3.*t5.*t6.*t7.*t8.*t10.*t34.*2.0+dQ1.*dQ2.*m5.*t2.*t3.*t4.*t5.*t7.*t8.*t10.*t16.*8.0+dQ1.*dQ3.*m5.*t2.*t3.*t4.*t5.*t7.*t8.*t10.*t16.*8.0+dQ1.*dQ2.*m6.*t2.*t3.*t4.*t5.*t7.*t8.*t10.*t20.*8.0-dQ1.*dQ6.*m6.*t2.*t3.*t4.*t5.*t7.*t8.*t9.*t17.*4.0+dQ1.*dQ3.*m6.*t2.*t3.*t4.*t5.*t7.*t8.*t10.*t20.*8.0-dQ1.*dQ2.*m6.*t2.*t3.*t4.*t5.*t7.*t8.*t10.*t22.*8.0-dQ1.*dQ2.*m6.*t2.*t4.*t5.*t6.*t7.*t9.*t11.*t17.*4.0-dQ1.*dQ4.*m6.*t2.*t3.*t5.*t6.*t7.*t8.*t11.*t17.*4.0-dQ1.*dQ3.*m6.*t2.*t3.*t4.*t5.*t7.*t8.*t10.*t22.*8.0-dQ1.*dQ3.*m6.*t2.*t4.*t5.*t6.*t7.*t9.*t11.*t17.*4.0;
et320 = dQ1.*dQ6.*m6.*t2.*t3.*t4.*t5.*t7.*t8.*t9.*t20.*4.0-dQ1.*dQ2.*m5.*t2.*t3.*t4.*t5.*t7.*t8.*t10.*t25.*8.0-dQ1.*dQ2.*m6.*t3.*t4.*t5.*t6.*t8.*t9.*t11.*t17.*4.0+dQ1.*dQ2.*m6.*t2.*t4.*t5.*t6.*t7.*t9.*t11.*t20.*4.0-dQ1.*dQ3.*m5.*t2.*t3.*t4.*t5.*t7.*t8.*t10.*t25.*8.0-dQ1.*dQ3.*m6.*t3.*t4.*t5.*t6.*t8.*t9.*t11.*t17.*4.0+dQ1.*dQ4.*m6.*t2.*t3.*t5.*t6.*t7.*t8.*t11.*t20.*4.0-dQ1.*dQ2.*m6.*t2.*t3.*t4.*t5.*t7.*t8.*t10.*t26.*8.0+dQ1.*dQ3.*m6.*t2.*t4.*t5.*t6.*t7.*t9.*t11.*t20.*4.0-dQ2.*dQ4.*m6.*t2.*t4.*t5.*t6.*t8.*t9.*t11.*t17.*4.0-dQ2.*dQ4.*m6.*t3.*t4.*t5.*t6.*t7.*t9.*t11.*t17.*4.0+dQ1.*dQ2.*m6.*t3.*t4.*t5.*t6.*t8.*t9.*t11.*t20.*4.0-dQ1.*dQ3.*m6.*t2.*t3.*t4.*t5.*t7.*t8.*t10.*t26.*8.0-dQ1.*dQ6.*m6.*t2.*t4.*t5.*t6.*t7.*t10.*t11.*t17.*4.0;
et321 = dQ3.*dQ4.*m6.*t2.*t4.*t5.*t6.*t8.*t9.*t11.*t17.*-4.0-dQ3.*dQ4.*m6.*t3.*t4.*t5.*t6.*t7.*t9.*t11.*t17.*4.0+dQ1.*dQ3.*m6.*t3.*t4.*t5.*t6.*t8.*t9.*t11.*t20.*4.0-dQ1.*dQ6.*m6.*t3.*t4.*t5.*t6.*t8.*t10.*t11.*t17.*4.0+dQ2.*dQ4.*m6.*t2.*t4.*t5.*t6.*t8.*t9.*t11.*t20.*4.0+dQ2.*dQ4.*m6.*t3.*t4.*t5.*t6.*t7.*t9.*t11.*t20.*4.0-dQ2.*dQ6.*m6.*t2.*t3.*t5.*t6.*t9.*t10.*t11.*t17.*2.0+dQ1.*dQ6.*m6.*t2.*t4.*t5.*t6.*t7.*t10.*t11.*t20.*4.0+dQ3.*dQ4.*m6.*t2.*t4.*t5.*t6.*t8.*t9.*t11.*t20.*4.0+dQ3.*dQ4.*m6.*t3.*t4.*t5.*t6.*t7.*t9.*t11.*t20.*4.0-dQ3.*dQ6.*m6.*t2.*t3.*t5.*t6.*t9.*t10.*t11.*t17.*2.0+dQ4.*dQ6.*m6.*t2.*t4.*t5.*t6.*t8.*t10.*t11.*t17.*2.0+dQ4.*dQ6.*m6.*t3.*t4.*t5.*t6.*t7.*t10.*t11.*t17.*2.0+dQ1.*dQ6.*m6.*t3.*t4.*t5.*t6.*t8.*t10.*t11.*t20.*4.0+dQ2.*dQ6.*m6.*t2.*t3.*t5.*t6.*t9.*t10.*t11.*t20.*2.0;
et322 = dQ3.*dQ6.*m6.*t2.*t3.*t5.*t6.*t9.*t10.*t11.*t20.*2.0-dQ4.*dQ6.*m6.*t2.*t4.*t5.*t6.*t8.*t10.*t11.*t20.*2.0-dQ4.*dQ6.*m6.*t3.*t4.*t5.*t6.*t7.*t10.*t11.*t20.*2.0+dQ2.*dQ6.*m6.*t5.*t6.*t7.*t8.*t9.*t10.*t11.*t17.*2.0+dQ3.*dQ6.*m6.*t5.*t6.*t7.*t8.*t9.*t10.*t11.*t17.*2.0-dQ2.*dQ6.*m6.*t5.*t6.*t7.*t8.*t9.*t10.*t11.*t20.*2.0-dQ3.*dQ6.*m6.*t5.*t6.*t7.*t8.*t9.*t10.*t11.*t20.*2.0+dQ1.*dQ4.*m5.*t2.*t3.*t4.*t7.*t8.*t9.*t16.*t35.*4.0+dQ1.*dQ5.*m5.*t2.*t3.*t5.*t7.*t8.*t10.*t16.*t34.*4.0+dQ1.*dQ4.*m6.*t2.*t3.*t4.*t7.*t8.*t9.*t17.*t36.*4.0+dQ1.*dQ4.*m6.*t2.*t3.*t4.*t7.*t8.*t9.*t20.*t35.*4.0-dQ1.*dQ4.*m6.*t2.*t3.*t4.*t7.*t8.*t9.*t20.*t36.*4.0+dQ1.*dQ5.*m6.*t2.*t3.*t5.*t7.*t8.*t10.*t17.*t36.*4.0-dQ1.*dQ4.*m6.*t2.*t3.*t4.*t7.*t8.*t9.*t22.*t35.*4.0;
et323 = dQ1.*dQ4.*m6.*t2.*t4.*t6.*t7.*t10.*t11.*t17.*t33.*4.0+dQ1.*dQ5.*m6.*t2.*t3.*t5.*t7.*t8.*t10.*t20.*t34.*4.0+dQ1.*dQ6.*m6.*t2.*t3.*t6.*t7.*t8.*t11.*t17.*t34.*4.0+dQ1.*dQ4.*m6.*t3.*t4.*t6.*t8.*t10.*t11.*t17.*t32.*4.0+dQ1.*dQ5.*m6.*t2.*t5.*t6.*t7.*t9.*t11.*t17.*t33.*4.0+dQ1.*dQ6.*m6.*t2.*t3.*t6.*t7.*t8.*t11.*t17.*t35.*4.0-dQ1.*dQ4.*m5.*t2.*t3.*t4.*t7.*t8.*t9.*t25.*t35.*4.0-dQ1.*dQ5.*m6.*t2.*t3.*t5.*t7.*t8.*t10.*t20.*t36.*4.0-dQ1.*dQ5.*m6.*t2.*t3.*t5.*t7.*t8.*t10.*t22.*t34.*4.0+dQ1.*dQ5.*m6.*t3.*t5.*t6.*t8.*t9.*t11.*t17.*t32.*4.0-dQ1.*dQ4.*m6.*t2.*t4.*t6.*t7.*t10.*t11.*t20.*t33.*4.0-dQ1.*dQ6.*m6.*t2.*t3.*t6.*t7.*t8.*t11.*t20.*t34.*4.0-dQ2.*dQ5.*m6.*t2.*t4.*t5.*t8.*t9.*t10.*t17.*t36.*2.0-dQ2.*dQ5.*m6.*t3.*t4.*t5.*t7.*t9.*t10.*t17.*t36.*2.0;
et324 = dQ1.*dQ4.*m6.*t2.*t3.*t4.*t7.*t8.*t9.*t26.*t35.*-4.0-dQ1.*dQ4.*m6.*t3.*t4.*t6.*t8.*t10.*t11.*t20.*t32.*4.0-dQ1.*dQ5.*m5.*t2.*t3.*t5.*t7.*t8.*t10.*t25.*t34.*4.0-dQ1.*dQ5.*m6.*t2.*t5.*t6.*t7.*t9.*t11.*t20.*t33.*4.0-dQ1.*dQ6.*m6.*t2.*t3.*t6.*t7.*t8.*t11.*t20.*t35.*4.0-dQ3.*dQ5.*m6.*t2.*t4.*t5.*t8.*t9.*t10.*t17.*t36.*2.0-dQ3.*dQ5.*m6.*t3.*t4.*t5.*t7.*t9.*t10.*t17.*t36.*2.0-dQ1.*dQ5.*m6.*t3.*t5.*t6.*t8.*t9.*t11.*t20.*t32.*4.0-dQ2.*dQ6.*m6.*t2.*t4.*t6.*t8.*t9.*t11.*t17.*t35.*2.0-dQ2.*dQ6.*m6.*t3.*t4.*t6.*t7.*t9.*t11.*t17.*t35.*2.0-dQ1.*dQ5.*m6.*t2.*t3.*t5.*t7.*t8.*t10.*t26.*t34.*4.0-dQ3.*dQ6.*m6.*t2.*t4.*t6.*t8.*t9.*t11.*t17.*t35.*2.0-dQ3.*dQ6.*m6.*t3.*t4.*t6.*t7.*t9.*t11.*t17.*t35.*2.0+dQ1.*dQ4.*m6.*t2.*t5.*t7.*t9.*t10.*t17.*t33.*t36.*4.0;
et325 = dQ1.*dQ4.*m6.*t3.*t5.*t8.*t9.*t10.*t17.*t32.*t36.*4.0-dQ1.*dQ4.*m6.*t2.*t5.*t7.*t9.*t10.*t20.*t33.*t36.*4.0-dQ1.*dQ4.*m6.*t3.*t5.*t8.*t9.*t10.*t20.*t32.*t36.*4.0+dQ1.*dQ5.*m6.*t4.*t6.*t9.*t10.*t11.*t17.*t32.*t33.*4.0-dQ1.*dQ5.*m6.*t4.*t6.*t9.*t10.*t11.*t20.*t32.*t33.*4.0-Lx2.*Lxcm6.*dQ1.*dQ2.*m6.*t2.*t3.*t4.*t5.*t6.*t7.*4.0-Lx2.*Lxcm6.*dQ1.*dQ3.*m6.*t2.*t3.*t4.*t5.*t6.*t7.*2.0+Lx3.*Lxcm5.*dQ1.*dQ4.*m5.*t2.*t3.*t5.*t7.*t8.*t9.*4.0+Lx3.*Lxcm5.*dQ1.*dQ5.*m5.*t2.*t3.*t4.*t7.*t8.*t10.*4.0+Lx3.*Lxcm6.*dQ1.*dQ2.*m6.*t2.*t3.*t6.*t7.*t8.*t10.*8.0+Lx3.*Lxcm6.*dQ1.*dQ3.*m6.*t2.*t3.*t6.*t7.*t8.*t10.*8.0+Lx3.*Lxcm6.*dQ1.*dQ4.*m6.*t2.*t3.*t4.*t7.*t8.*t11.*4.0+Lx2.*Lxcm6.*dQ1.*dQ4.*m6.*t2.*t5.*t6.*t7.*t8.*t9.*2.0+Lx2.*Lxcm6.*dQ1.*dQ5.*m6.*t2.*t4.*t6.*t7.*t8.*t10.*2.0;
et326 = Lx3.*Lxcm6.*dQ1.*dQ6.*m6.*t2.*t3.*t6.*t7.*t8.*t9.*4.0+Lx2.*Lxcm6.*dQ1.*dQ6.*m6.*t2.*t4.*t5.*t7.*t8.*t11.*2.0-Lx3.*Lxcm6.*dQ1.*dQ2.*m6.*t2.*t4.*t5.*t6.*t7.*t33.*8.0-Lx3.*Lxcm6.*dQ1.*dQ2.*m6.*t3.*t4.*t5.*t6.*t8.*t32.*8.0-Lx3.*Lxcm6.*dQ1.*dQ3.*m6.*t2.*t4.*t5.*t6.*t7.*t33.*8.0-Lx3.*Lxcm6.*dQ1.*dQ3.*m6.*t3.*t4.*t5.*t6.*t8.*t32.*8.0+Lx2.*Lycm6.*dQ1.*dQ2.*m6.*t2.*t3.*t4.*t5.*t7.*t11.*4.0+Lx2.*Lycm6.*dQ1.*dQ3.*m6.*t2.*t3.*t4.*t5.*t7.*t11.*2.0+Lx3.*Lycm6.*dQ1.*dQ4.*m6.*t2.*t3.*t4.*t6.*t7.*t8.*4.0+Lx2.*Lycm6.*dQ1.*dQ6.*m6.*t2.*t4.*t5.*t6.*t7.*t8.*2.0-Lx3.*Lycm6.*dQ1.*dQ2.*m6.*t2.*t3.*t7.*t8.*t10.*t11.*8.0-Lx3.*Lycm6.*dQ1.*dQ3.*m6.*t2.*t3.*t7.*t8.*t10.*t11.*8.0-Lx2.*Lycm6.*dQ1.*dQ4.*m6.*t2.*t5.*t7.*t8.*t9.*t11.*2.0-Lx2.*Lycm6.*dQ1.*dQ5.*m6.*t2.*t4.*t7.*t8.*t10.*t11.*2.0;
et327 = Lx3.*Lycm6.*dQ1.*dQ6.*m6.*t2.*t3.*t7.*t8.*t9.*t11.*-4.0+Lx3.*Lycm6.*dQ1.*dQ2.*m6.*t2.*t4.*t5.*t7.*t11.*t33.*8.0+Lx3.*Lycm6.*dQ1.*dQ2.*m6.*t3.*t4.*t5.*t8.*t11.*t32.*8.0+Lx3.*Lycm6.*dQ1.*dQ3.*m6.*t2.*t4.*t5.*t7.*t11.*t33.*8.0+Lx3.*Lycm6.*dQ1.*dQ3.*m6.*t3.*t4.*t5.*t8.*t11.*t32.*8.0-Lxcm5.*Lycm5.*dQ1.*dQ2.*m5.*t2.*t3.*t7.*t8.*t9.*t10.*8.0-Lxcm5.*Lycm5.*dQ1.*dQ3.*m5.*t2.*t3.*t7.*t8.*t9.*t10.*8.0-Lxcm6.*Lycm6.*dQ2.*dQ3.*m6.*t2.*t3.*t4.*t6.*t9.*t11.*4.0+Lxcm6.*Lycm6.*dQ1.*dQ2.*m6.*t2.*t3.*t7.*t8.*t9.*t10.*8.0+Lxcm6.*Lycm6.*dQ1.*dQ3.*m6.*t2.*t3.*t7.*t8.*t9.*t10.*8.0-Lxcm6.*Lycm6.*dQ2.*dQ6.*m6.*t2.*t3.*t4.*t6.*t10.*t11.*4.0-Lxcm6.*Lycm6.*dQ3.*dQ6.*m6.*t2.*t3.*t4.*t6.*t10.*t11.*4.0+Lxcm6.*Lycm6.*dQ4.*dQ5.*m6.*t2.*t3.*t5.*t6.*t10.*t11.*4.0-Lxcm6.*Lycm6.*dQ5.*dQ6.*m6.*t2.*t4.*t5.*t6.*t8.*t11.*4.0;
et328 = Lxcm6.*Lycm6.*dQ5.*dQ6.*m6.*t3.*t4.*t5.*t6.*t7.*t11.*-4.0+Lxcm6.*Lycm6.*dQ2.*dQ3.*m6.*t4.*t6.*t7.*t8.*t9.*t11.*4.0+Lxcm6.*Lycm6.*dQ1.*dQ6.*m6.*t2.*t6.*t7.*t9.*t10.*t11.*8.0+Lxcm6.*Lycm6.*dQ1.*dQ6.*m6.*t3.*t6.*t8.*t9.*t10.*t11.*8.0+Lxcm6.*Lycm6.*dQ2.*dQ6.*m6.*t4.*t6.*t7.*t8.*t10.*t11.*4.0+Lxcm6.*Lycm6.*dQ3.*dQ6.*m6.*t4.*t6.*t7.*t8.*t10.*t11.*4.0-Lxcm6.*Lycm6.*dQ4.*dQ5.*m6.*t5.*t6.*t7.*t8.*t10.*t11.*4.0-Lxcm6.*Lycm6.*dQ4.*dQ6.*m6.*t2.*t6.*t8.*t9.*t10.*t11.*4.0-Lxcm6.*Lycm6.*dQ4.*dQ6.*m6.*t3.*t6.*t7.*t9.*t10.*t11.*4.0+Lxcm5.*Lycm5.*dQ1.*dQ2.*m5.*t2.*t4.*t5.*t7.*t9.*t33.*8.0+Lxcm5.*Lycm5.*dQ1.*dQ2.*m5.*t3.*t4.*t5.*t8.*t9.*t32.*8.0+Lxcm5.*Lycm5.*dQ1.*dQ3.*m5.*t2.*t4.*t5.*t7.*t9.*t33.*8.0+Lxcm5.*Lycm5.*dQ1.*dQ4.*m5.*t2.*t3.*t5.*t7.*t8.*t34.*8.0+Lxcm5.*Lycm5.*dQ1.*dQ3.*m5.*t3.*t4.*t5.*t8.*t9.*t32.*8.0;
et329 = Lxcm6.*Lycm6.*dQ1.*dQ2.*m6.*t2.*t4.*t5.*t7.*t9.*t33.*-8.0-Lxcm6.*Lycm6.*dQ1.*dQ2.*m6.*t3.*t4.*t5.*t8.*t9.*t32.*8.0-Lxcm6.*Lycm6.*dQ1.*dQ3.*m6.*t2.*t4.*t5.*t7.*t9.*t33.*8.0-Lxcm6.*Lycm6.*dQ1.*dQ4.*m6.*t2.*t3.*t5.*t7.*t8.*t34.*8.0-Lxcm6.*Lycm6.*dQ1.*dQ3.*m6.*t3.*t4.*t5.*t8.*t9.*t32.*8.0-Lxcm6.*Lycm6.*dQ1.*dQ2.*m6.*t2.*t4.*t5.*t7.*t9.*t36.*8.0-Lxcm6.*Lycm6.*dQ1.*dQ4.*m6.*t2.*t3.*t5.*t7.*t8.*t36.*8.0-Lxcm6.*Lycm6.*dQ1.*dQ3.*m6.*t2.*t4.*t5.*t7.*t9.*t36.*8.0-Lxcm6.*Lycm6.*dQ1.*dQ2.*m6.*t3.*t4.*t5.*t8.*t9.*t36.*8.0-Lxcm6.*Lycm6.*dQ1.*dQ6.*m6.*t2.*t4.*t5.*t7.*t10.*t33.*8.0-Lxcm6.*Lycm6.*dQ1.*dQ3.*m6.*t3.*t4.*t5.*t8.*t9.*t36.*8.0-Lxcm6.*Lycm6.*dQ1.*dQ5.*m6.*t2.*t4.*t6.*t7.*t11.*t33.*8.0-Lxcm6.*Lycm6.*dQ1.*dQ6.*m6.*t3.*t4.*t5.*t8.*t10.*t32.*8.0;
et330 = Lxcm6.*Lycm6.*dQ1.*dQ5.*m6.*t3.*t4.*t6.*t8.*t11.*t32.*-8.0-Lxcm6.*Lycm6.*dQ2.*dQ4.*m6.*t2.*t4.*t5.*t8.*t9.*t36.*8.0-Lxcm6.*Lycm6.*dQ2.*dQ4.*m6.*t3.*t4.*t5.*t7.*t9.*t36.*8.0-Lxcm6.*Lycm6.*dQ1.*dQ2.*m6.*t4.*t5.*t6.*t10.*t11.*t32.*8.0-Lxcm6.*Lycm6.*dQ1.*dQ5.*m6.*t2.*t4.*t6.*t7.*t11.*t35.*8.0-Lxcm6.*Lycm6.*dQ1.*dQ6.*m6.*t2.*t4.*t5.*t7.*t10.*t36.*8.0-Lxcm6.*Lycm6.*dQ3.*dQ4.*m6.*t2.*t4.*t5.*t8.*t9.*t36.*8.0-Lxcm6.*Lycm6.*dQ3.*dQ4.*m6.*t3.*t4.*t5.*t7.*t9.*t36.*8.0-Lxcm6.*Lycm6.*dQ1.*dQ2.*m6.*t4.*t5.*t6.*t10.*t11.*t33.*8.0-Lxcm6.*Lycm6.*dQ1.*dQ3.*m6.*t4.*t5.*t6.*t10.*t11.*t32.*8.0-Lxcm6.*Lycm6.*dQ1.*dQ3.*m6.*t4.*t5.*t6.*t10.*t11.*t33.*8.0-Lxcm6.*Lycm6.*dQ1.*dQ5.*m6.*t3.*t4.*t6.*t8.*t11.*t35.*8.0-Lxcm6.*Lycm6.*dQ1.*dQ6.*m6.*t3.*t4.*t5.*t8.*t10.*t36.*8.0;
et331 = Lxcm6.*Lycm6.*dQ2.*dQ5.*m6.*t2.*t3.*t6.*t9.*t11.*t35.*-4.0-Lxcm6.*Lycm6.*dQ2.*dQ6.*m6.*t2.*t3.*t5.*t9.*t10.*t36.*4.0-Lxcm6.*Lycm6.*dQ1.*dQ6.*m6.*t4.*t5.*t6.*t9.*t11.*t32.*8.0-Lxcm6.*Lycm6.*dQ2.*dQ6.*m6.*t2.*t5.*t6.*t8.*t11.*t34.*8.0-Lxcm6.*Lycm6.*dQ2.*dQ6.*m6.*t3.*t5.*t6.*t7.*t11.*t34.*8.0-Lxcm6.*Lycm6.*dQ3.*dQ5.*m6.*t2.*t3.*t6.*t9.*t11.*t35.*4.0-Lxcm6.*Lycm6.*dQ3.*dQ6.*m6.*t2.*t3.*t5.*t9.*t10.*t36.*4.0-Lxcm6.*Lycm6.*dQ1.*dQ6.*m6.*t4.*t5.*t6.*t9.*t11.*t33.*8.0-Lxcm6.*Lycm6.*dQ3.*dQ6.*m6.*t2.*t5.*t6.*t8.*t11.*t34.*8.0-Lxcm6.*Lycm6.*dQ3.*dQ6.*m6.*t3.*t5.*t6.*t7.*t11.*t34.*8.0+Lxcm6.*Lycm6.*dQ4.*dQ5.*m6.*t2.*t4.*t6.*t8.*t11.*t35.*4.0+Lxcm6.*Lycm6.*dQ4.*dQ5.*m6.*t3.*t4.*t6.*t7.*t11.*t35.*4.0+Lxcm6.*Lycm6.*dQ4.*dQ6.*m6.*t2.*t4.*t5.*t8.*t10.*t36.*4.0+Lxcm6.*Lycm6.*dQ4.*dQ6.*m6.*t3.*t4.*t5.*t7.*t10.*t36.*4.0;
et332 = Lxcm6.*Lycm6.*dQ2.*dQ5.*m6.*t6.*t7.*t8.*t9.*t11.*t35.*4.0+Lxcm6.*Lycm6.*dQ2.*dQ6.*m6.*t5.*t7.*t8.*t9.*t10.*t36.*4.0+Lxcm6.*Lycm6.*dQ3.*dQ5.*m6.*t6.*t7.*t8.*t9.*t11.*t35.*4.0+Lxcm6.*Lycm6.*dQ3.*dQ6.*m6.*t5.*t7.*t8.*t9.*t10.*t36.*4.0+Lxcm6.*Lycm6.*dQ1.*dQ2.*m6.*t2.*t6.*t7.*t11.*t33.*t34.*8.0-Lxcm6.*Lycm6.*dQ1.*dQ6.*m6.*t2.*t3.*t7.*t8.*t34.*t35.*4.0+Lxcm6.*Lycm6.*dQ1.*dQ2.*m6.*t2.*t6.*t7.*t11.*t33.*t35.*8.0+Lxcm6.*Lycm6.*dQ1.*dQ2.*m6.*t3.*t6.*t8.*t11.*t32.*t34.*8.0+Lxcm6.*Lycm6.*dQ1.*dQ3.*m6.*t2.*t6.*t7.*t11.*t33.*t34.*8.0+Lxcm6.*Lycm6.*dQ1.*dQ4.*m6.*t2.*t4.*t7.*t10.*t33.*t36.*8.0+Lxcm6.*Lycm6.*dQ1.*dQ6.*m6.*t2.*t3.*t7.*t8.*t34.*t36.*8.0-Lxcm6.*Lycm6.*dQ1.*dQ2.*m6.*t2.*t6.*t7.*t11.*t34.*t35.*4.0+Lxcm6.*Lycm6.*dQ1.*dQ2.*m6.*t3.*t6.*t8.*t11.*t32.*t35.*8.0+Lxcm6.*Lycm6.*dQ1.*dQ3.*m6.*t2.*t6.*t7.*t11.*t33.*t35.*8.0;
et333 = Lxcm6.*Lycm6.*dQ1.*dQ3.*m6.*t3.*t6.*t8.*t11.*t32.*t34.*8.0+Lxcm6.*Lycm6.*dQ1.*dQ4.*m6.*t3.*t4.*t8.*t10.*t32.*t36.*8.0+Lxcm6.*Lycm6.*dQ1.*dQ5.*m6.*t2.*t5.*t7.*t9.*t33.*t36.*8.0+Lxcm6.*Lycm6.*dQ1.*dQ6.*m6.*t2.*t3.*t7.*t8.*t35.*t36.*8.0-Lxcm6.*Lycm6.*dQ1.*dQ3.*m6.*t2.*t6.*t7.*t11.*t34.*t35.*4.0+Lxcm6.*Lycm6.*dQ1.*dQ3.*m6.*t3.*t6.*t8.*t11.*t32.*t35.*8.0+Lxcm6.*Lycm6.*dQ1.*dQ5.*m6.*t3.*t5.*t8.*t9.*t32.*t36.*8.0-Lxcm6.*Lycm6.*dQ1.*dQ2.*m6.*t3.*t6.*t8.*t11.*t34.*t35.*4.0+Lxcm6.*Lycm6.*dQ1.*dQ4.*m6.*t4.*t6.*t9.*t11.*t32.*t33.*8.0-Lxcm6.*Lycm6.*dQ1.*dQ3.*m6.*t3.*t6.*t8.*t11.*t34.*t35.*4.0-Lxcm6.*Lycm6.*dQ1.*dQ4.*m6.*t4.*t6.*t9.*t11.*t32.*t35.*4.0-Lxcm6.*Lycm6.*dQ2.*dQ4.*m6.*t2.*t6.*t8.*t11.*t34.*t35.*4.0-Lxcm6.*Lycm6.*dQ2.*dQ4.*m6.*t3.*t6.*t7.*t11.*t34.*t35.*4.0-Lxcm6.*Lycm6.*dQ2.*dQ6.*m6.*t2.*t4.*t8.*t9.*t35.*t36.*4.0;
et334 = Lxcm6.*Lycm6.*dQ2.*dQ6.*m6.*t3.*t4.*t7.*t9.*t35.*t36.*-4.0-Lxcm6.*Lycm6.*dQ1.*dQ4.*m6.*t4.*t6.*t9.*t11.*t33.*t35.*4.0+Lxcm6.*Lycm6.*dQ1.*dQ5.*m6.*t5.*t6.*t10.*t11.*t32.*t33.*8.0-Lxcm6.*Lycm6.*dQ3.*dQ4.*m6.*t2.*t6.*t8.*t11.*t34.*t35.*4.0-Lxcm6.*Lycm6.*dQ3.*dQ4.*m6.*t3.*t6.*t7.*t11.*t34.*t35.*4.0-Lxcm6.*Lycm6.*dQ3.*dQ6.*m6.*t2.*t4.*t8.*t9.*t35.*t36.*4.0-Lxcm6.*Lycm6.*dQ3.*dQ6.*m6.*t3.*t4.*t7.*t9.*t35.*t36.*4.0-Lxcm6.*Lycm6.*dQ1.*dQ5.*m6.*t5.*t6.*t10.*t11.*t32.*t34.*4.0-Lxcm6.*Lycm6.*dQ1.*dQ5.*m6.*t5.*t6.*t10.*t11.*t33.*t34.*4.0+Lxcm6.*Lycm6.*dQ1.*dQ5.*m6.*t4.*t9.*t10.*t32.*t33.*t36.*8.0-Lx3.*Lz5.*dQ1.*dQ5.*m6.*t2.*t3.*t4.*t5.*t7.*t8.*4.0+Lx3.*Lz5.*dQ1.*dQ4.*m6.*t2.*t3.*t7.*t8.*t9.*t10.*4.0-Lxcm5.*Lz4.*dQ1.*dQ2.*m5.*t2.*t3.*t4.*t5.*t7.*t8.*8.0-Lxcm5.*Lz4.*dQ1.*dQ3.*m5.*t2.*t3.*t4.*t5.*t7.*t8.*8.0;
et335 = Lx3.*Lzcm5.*dQ1.*dQ5.*m5.*t2.*t3.*t4.*t5.*t7.*t8.*-4.0-Lx3.*Lzcm6.*dQ1.*dQ5.*m6.*t2.*t3.*t4.*t5.*t7.*t8.*4.0+Lxcm6.*Lz5.*dQ1.*dQ2.*m6.*t2.*t3.*t4.*t6.*t7.*t8.*8.0+Lxcm6.*Lz5.*dQ1.*dQ3.*m6.*t2.*t3.*t4.*t6.*t7.*t8.*8.0-Lxcm6.*Lz4.*dQ1.*dQ5.*m6.*t2.*t3.*t5.*t6.*t7.*t8.*4.0+Lx3.*Lzcm5.*dQ1.*dQ4.*m5.*t2.*t3.*t7.*t8.*t9.*t10.*4.0+Lxcm6.*Lz5.*dQ1.*dQ5.*m6.*t2.*t4.*t5.*t6.*t7.*t10.*8.0+Lx3.*Lzcm6.*dQ1.*dQ4.*m6.*t2.*t3.*t7.*t8.*t9.*t10.*4.0+Lxcm6.*Lz4.*dQ1.*dQ2.*m6.*t2.*t3.*t7.*t8.*t9.*t11.*8.0+Lxcm6.*Lz5.*dQ1.*dQ5.*m6.*t3.*t4.*t5.*t6.*t8.*t10.*8.0+Lxcm6.*Lz5.*dQ2.*dQ5.*m6.*t2.*t3.*t5.*t6.*t9.*t10.*4.0+Lxcm6.*Lz4.*dQ1.*dQ3.*m6.*t2.*t3.*t7.*t8.*t9.*t11.*8.0+Lxcm6.*Lz5.*dQ3.*dQ5.*m6.*t2.*t3.*t5.*t6.*t9.*t10.*4.0-Lxcm6.*Lz5.*dQ4.*dQ5.*m6.*t2.*t4.*t5.*t6.*t8.*t10.*4.0;
